simulink model "KUKA_LBR_Simulink_model_flatness_based_control"  (R2017a)
settings: Solver=VariableStepAuto  StartTime=0.0  StopTime=T  RelTol=1e-3
InitFcn:
  | main
values from neighbouring files (symbols this model uses):
  elbowAngle = elbowAngle * pi/180    (= 0)    [KUKA_LBR_init.m]    (also in Untitled2.m)
  KAnaJacNum = [k_ind 0 0 0 0 0 ;                 0  k_ind 0 0 0 0 ;                    0 0 k_ind 0 0 0 ;                      0 0 0 k_ind 0 0 ;                        0 0 0 0 k_ind 0 ;                          0 0 0 0 0 k_ind ;                            ]    [KUKA_LBR_init.m]
  Kuka_LBR_param_simu = Simulink.Parameter(Kuka_LBR_param_simu)    [KUKA_LBR_init.m]
  KUKA_LBR_x0 = [x1_0 x2_0 x3_0 x4_0 x5_0 x6_0 x7_0 x8_0 x9_0 x10_0 x11_0 x12_0 x13_0 x14_0]    [KUKA_LBR_init.m]
  rpyDes = rpyDes * pi/180    [KUKA_LBR_init.m]    (also in Untitled2.m)
  T = 0.5    [KUKA_LBR_init.m]
  vecGlobalConfig = [1; 1; 1]    [KUKA_LBR_init.m]    (also in Untitled2.m = [1, 1, 1])
undefined symbols (not defined in the file or in its folder): Kuka_LBR_param
(part 5 of 19)

== matlab function KUKA_LBR_Simulink_model_flatness_based_control/KUKA_LBR_Computed_Torque ==
  data: KUKA_LBR_param_ input; vecJointPos_ input; tau output; vecJointVel_ input; vecJointAcc_ input
function tau = KUKA_LBR_Computed_Torque(KUKA_LBR_param_,vecJointPos_,vecJointVel_,vecJointAcc_)

q1 = vecJointPos_(1);
q2 = vecJointPos_(2);
q3 = vecJointPos_(3);
q4 = vecJointPos_(4);
q5 = vecJointPos_(5);
q6 = vecJointPos_(6);
q7 = vecJointPos_(7);
q8 = vecJointVel_(1);
q9 = vecJointVel_(2);
q10 = vecJointVel_(3);
q11 = vecJointVel_(4);
q12 = vecJointVel_(5);
q13 = vecJointVel_(6);
q14 = vecJointVel_(7);


dblMassInertFullRow1Col1 = KUKA_LBR_param_.dblLink1InertZZ + (power(KUKA_LBR_param_.dblLink1CogX,2) + power(KUKA_LBR_param_.dblLink1CogY,2))*KUKA_LBR_param_.dblLink1Mass + KUKA_LBR_param_.dblLink2InertZZ + KUKA_LBR_param_.dblLink3InertZZ + KUKA_LBR_param_.dblLink4InertZZ + KUKA_LBR_param_.dblLink5InertZZ + KUKA_LBR_param_.dblLink6InertZZ + KUKA_LBR_param_.dblLink7InertZZ + KUKA_LBR_param_.dblLink2Mass*power(KUKA_LBR_param_.dblLink2CogZ*sin(q1) + cos(q1)*(KUKA_LBR_param_.dblLink2CogX*cos(q2) - KUKA_LBR_param_.dblLink2CogY*sin(q2)),2) + KUKA_LBR_param_.dblLink2Mass*power(KUKA_LBR_param_.dblLink2CogZ*cos(q1) + sin(q1)*(-(KUKA_LBR_param_.dblLink2CogX*cos(q2)) + KUKA_LBR_param_.dblLink2CogY*sin(q2)),2) + KUKA_LBR_param_.dblLink3Mass*power(cos(q1)*(KUKA_LBR_param_.dblLink3CogY*cos(q3) + KUKA_LBR_param_.dblLink3CogX*sin(q3)) + sin(q1)*(-((KUKA_LBR_param_.dblLink23Len + KUKA_LBR_param_.dblLink3CogZ)*sin(q2)) + cos(q2)*(KUKA_LBR_param_.dblLink3CogX*cos(q3) - KUKA_LBR_param_.dblLink3CogY*sin(q3))),2) + KUKA_LBR_param_.dblLink3Mass*power(sin(q1)*(KUKA_LBR_param_.dblLink3CogY*cos(q3) + KUKA_LBR_param_.dblLink3CogX*sin(q3)) + cos(q1)*((KUKA_LBR_param_.dblLink23Len + KUKA_LBR_param_.dblLink3CogZ)*sin(q2) + cos(q2)*(-(KUKA_LBR_param_.dblLink3CogX*cos(q3)) + KUKA_LBR_param_.dblLink3CogY*sin(q3))),2) + KUKA_LBR_param_.dblLink4Mass*power(cos(q1)*(KUKA_LBR_param_.dblLink4CogZ*cos(q3) + sin(q3)*(KUKA_LBR_param_.dblLink4CogX*cos(q4) - KUKA_LBR_param_.dblLink4CogY*sin(q4))) + sin(q1)*(sin(q2)*(-KUKA_LBR_param_.dblLink23Len + KUKA_LBR_param_.dblLink4CogY*cos(q4) + KUKA_LBR_param_.dblLink4CogX*sin(q4)) + cos(q2)*(KUKA_LBR_param_.dblLink4CogX*cos(q3)*cos(q4) - KUKA_LBR_param_.dblLink4CogZ*sin(q3) - KUKA_LBR_param_.dblLink4CogY*cos(q3)*sin(q4))),2) + KUKA_LBR_param_.dblLink4Mass*power(sin(q1)*(KUKA_LBR_param_.dblLink4CogZ*cos(q3) + sin(q3)*(KUKA_LBR_param_.dblLink4CogX*cos(q4) - KUKA_LBR_param_.dblLink4CogY*sin(q4))) + cos(q1)*(sin(q2)*(KUKA_LBR_param_.dblLink23Len - KUKA_LBR_param_.dblLink4CogY*cos(q4) - KUKA_LBR_param_.dblLink4CogX*sin(q4)) + cos(q2)*(-(KUKA_LBR_param_.dblLink4CogX*cos(q3)*cos(q4)) + KUKA_LBR_param_.dblLink4CogZ*sin(q3) + KUKA_LBR_param_.dblLink4CogY*cos(q3)*sin(q4))),2) + KUKA_LBR_param_.dblLink5Mass*power(sin(q1)*(cos(q3)*(KUKA_LBR_param_.dblLink5CogY*cos(q5) + KUKA_LBR_param_.dblLink5CogX*sin(q5)) + sin(q3)*((KUKA_LBR_param_.dblLink45Len + KUKA_LBR_param_.dblLink5CogZ)*sin(q4) + cos(q4)*(KUKA_LBR_param_.dblLink5CogX*cos(q5) - KUKA_LBR_param_.dblLink5CogY*sin(q5)))) + cos(q1)*(sin(q2)*(KUKA_LBR_param_.dblLink23Len + (KUKA_LBR_param_.dblLink45Len + KUKA_LBR_param_.dblLink5CogZ)*cos(q4) - KUKA_LBR_param_.dblLink5CogX*cos(q5)*sin(q4) + KUKA_LBR_param_.dblLink5CogY*sin(q4)*sin(q5)) + cos(q2)*(sin(q3)*(KUKA_LBR_param_.dblLink5CogY*cos(q5) + KUKA_LBR_param_.dblLink5CogX*sin(q5)) - cos(q3)*((KUKA_LBR_param_.dblLink45Len + KUKA_LBR_param_.dblLink5CogZ)*sin(q4) + cos(q4)*(KUKA_LBR_param_.dblLink5CogX*cos(q5) - KUKA_LBR_param_.dblLink5CogY*sin(q5))))),2) + KUKA_LBR_param_.dblLink5Mass*power(cos(q1)*(cos(q3)*(KUKA_LBR_param_.dblLink5CogY*cos(q5) + KUKA_LBR_param_.dblLink5CogX*sin(q5)) + sin(q3)*((KUKA_LBR_param_.dblLink45Len + KUKA_LBR_param_.dblLink5CogZ)*sin(q4) + cos(q4)*(KUKA_LBR_param_.dblLink5CogX*cos(q5) - KUKA_LBR_param_.dblLink5CogY*sin(q5)))) + sin(q1)*(-(sin(q2)*(KUKA_LBR_param_.dblLink23Len + (KUKA_LBR_param_.dblLink45Len + KUKA_LBR_param_.dblLink5CogZ)*cos(q4) - KUKA_LBR_param_.dblLink5CogX*cos(q5)*sin(q4) + KUKA_LBR_param_.dblLink5CogY*sin(q4)*sin(q5))) + cos(q2)*(-(sin(q3)*(KUKA_LBR_param_.dblLink5CogY*cos(q5) + KUKA_LBR_param_.dblLink5CogX*sin(q5))) + cos(q3)*((KUKA_LBR_param_.dblLink45Len + KUKA_LBR_param_.dblLink5CogZ)*sin(q4) + cos(q4)*(KUKA_LBR_param_.dblLink5CogX*cos(q5) - KUKA_LBR_param_.dblLink5CogY*sin(q5))))),2) + KUKA_LBR_param_.dblLink6Mass*power(sin(q1)*(-(cos(q3)*(KUKA_LBR_param_.dblLink6CogZ*cos(q5) + sin(q5)*(-(KUKA_LBR_param_.dblLink6CogX*cos(q6)) + KUKA_LBR_param_.dblLink6CogY*sin(q6)))) + sin(q3)*(sin(q4)*(KUKA_LBR_param_.dblLink45Len + KUKA_LBR_param_.dblLink6CogY*cos(q6) + KUKA_LBR_param_.dblLink6CogX*sin(q6)) + cos(q4)*(KUKA_LBR_param_.dblLink6CogX*cos(q5)*cos(q6) + KUKA_LBR_param_.dblLink6CogZ*sin(q5) - KUKA_LBR_param_.dblLink6CogY*cos(q5)*sin(q6)))) - cos(q1)*(-(sin(q2)*(KUKA_LBR_param_.dblLink23Len - KUKA_LBR_param_.dblLink6CogX*cos(q5)*cos(q6)*sin(q4) - KUKA_LBR_param_.dblLink6CogZ*sin(q4)*sin(q5) + KUKA_LBR_param_.dblLink6CogY*cos(q5)*sin(q4)*sin(q6) + cos(q4)*(KUKA_LBR_param_.dblLink45Len + KUKA_LBR_param_.dblLink6CogY*cos(q6) + KUKA_LBR_param_.dblLink6CogX*sin(q6)))) + cos(q2)*(sin(q3)*(KUKA_LBR_param_.dblLink6CogZ*cos(q5) + sin(q5)*(-(KUKA_LBR_param_.dblLink6CogX*cos(q6)) + KUKA_LBR_param_.dblLink6CogY*sin(q6))) + cos(q3)*(sin(q4)*(KUKA_LBR_param_.dblLink45Len + KUKA_LBR_param_.dblLink6CogY*cos(q6) + KUKA_LBR_param_.dblLink6CogX*sin(q6)) + cos(q4)*(KUKA_LBR_param_.dblLink6CogX*cos(q5)*cos(q6) + KUKA_LBR_param_.dblLink6CogZ*sin(q5) - KUKA_LBR_param_.dblLink6CogY*cos(q5)*sin(q6))))),2) + KUKA_LBR_param_.dblLink6Mass*power(cos(q1)*(-(cos(q3)*(KUKA_LBR_param_.dblLink6CogZ*cos(q5) + sin(q5)*(-(KUKA_LBR_param_.dblLink6CogX*cos(q6)) + KUKA_LBR_param_.dblLink6CogY*sin(q6)))) + sin(q3)*(sin(q4)*(KUKA_LBR_param_.dblLink45Len + KUKA_LBR_param_.dblLink6CogY*cos(q6) + KUKA_LBR_param_.dblLink6CogX*sin(q6)) + cos(q4)*(KUKA_LBR_param_.dblLink6CogX*cos(q5)*cos(q6) + KUKA_LBR_param_.dblLink6CogZ*sin(q5) - KUKA_LBR_param_.dblLink6CogY*cos(q5)*sin(q6)))) + sin(q1)*(-(sin(q2)*(KUKA_LBR_param_.dblLink23Len - KUKA_LBR_param_.dblLink6CogX*cos(q5)*cos(q6)*sin(q4) - KUKA_LBR_param_.dblLink6CogZ*sin(q4)*sin(q5) + KUKA_LBR_param_.dblLink6CogY*cos(q5)*sin(q4)*sin(q6) + cos(q4)*(KUKA_LBR_param_.dblLink45Len + KUKA_LBR_param_.dblLink6CogY*cos(q6) + KUKA_LBR_param_.dblLink6CogX*sin(q6)))) + cos(q2)*(sin(q3)*(KUKA_LBR_param_.dblLink6CogZ*cos(q5) + sin(q5)*(-(KUKA_LBR_param_.dblLink6CogX*cos(q6)) + KUKA_LBR_param_.dblLink6CogY*sin(q6))) + cos(q3)*(sin(q4)*(KUKA_LBR_param_.dblLink45Len + KUKA_LBR_param_.dblLink6CogY*cos(q6) + KUKA_LBR_param_.dblLink6CogX*sin(q6)) + cos(q4)*(KUKA_LBR_param_.dblLink6CogX*cos(q5)*cos(q6) + KUKA_LBR_param_.dblLink6CogZ*sin(q5) - KUKA_LBR_param_.dblLink6CogY*cos(q5)*sin(q6))))),2) + KUKA_LBR_param_.dblLink7Mass*power(cos(q1)*(cos(q3)*(cos(q5)*(KUKA_LBR_param_.dblLink7CogY*cos(q7) + KUKA_LBR_param_.dblLink7CogX*sin(q7)) + sin(q5)*(KUKA_LBR_param_.dblLink7CogX*cos(q6)*cos(q7) - KUKA_LBR_param_.dblLink7CogZ*sin(q6) - KUKA_LBR_param_.dblLink7CogY*cos(q6)*sin(q7))) + sin(q3)*(sin(q4)*(KUKA_LBR_param_.dblLink45Len + KUKA_LBR_param_.dblLink7CogZ*cos(q6) + KUKA_LBR_param_.dblLink7CogX*cos(q7)*sin(q6) - KUKA_LBR_param_.dblLink7CogY*sin(q6)*sin(q7)) - cos(q4)*(sin(q5)*(KUKA_LBR_param_.dblLink7CogY*cos(q7) + KUKA_LBR_param_.dblLink7CogX*sin(q7)) + cos(q5)*(-(KUKA_LBR_param_.dblLink7CogX*cos(q6)*cos(q7)) + KUKA_LBR_param_.dblLink7CogZ*sin(q6) + KUKA_LBR_param_.dblLink7CogY*cos(q6)*sin(q7))))) + sin(q1)*(-(sin(q2)*(KUKA_LBR_param_.dblLink23Len + KUKA_LBR_param_.dblLink7CogY*cos(q7)*sin(q4)*sin(q5) + KUKA_LBR_param_.dblLink7CogX*sin(q4)*sin(q5)*sin(q7) + cos(q5)*sin(q4)*(-(KUKA_LBR_param_.dblLink7CogX*cos(q6)*cos(q7)) + KUKA_LBR_param_.dblLink7CogZ*sin(q6) + KUKA_LBR_param_.dblLink7CogY*cos(q6)*sin(q7)) + cos(q4)*(KUKA_LBR_param_.dblLink45Len + KUKA_LBR_param_.dblLink7CogZ*cos(q6) + KUKA_LBR_param_.dblLink7CogX*cos(q7)*sin(q6) - KUKA_LBR_param_.dblLink7CogY*sin(q6)*sin(q7)))) + cos(q2)*(-(sin(q3)*(cos(q5)*(KUKA_LBR_param_.dblLink7CogY*cos(q7) + KUKA_LBR_param_.dblLink7CogX*sin(q7)) + sin(q5)*(KUKA_LBR_param_.dblLink7CogX*cos(q6)*cos(q7) - KUKA_LBR_param_.dblLink7CogZ*sin(q6) - KUKA_LBR_param_.dblLink7CogY*cos(q6)*sin(q7)))) + cos(q3)*(sin(q4)*(KUKA_LBR_param_.dblLink45Len + KUKA_LBR_param_.dblLink7CogZ*cos(q6) + KUKA_LBR_param_.dblLink7CogX*cos(q7)*sin(q6) - KUKA_LBR_param_.dblLink7CogY*sin(q6)*sin(q7)) - cos(q4)*(sin(q5)*(KUKA_LBR_param_.dblLink7CogY*cos(q7) + KUKA_LBR_param_.dblLink7CogX*sin(q7)) + cos(q5)*(-(KUKA_LBR_param_.dblLink7CogX*cos(q6)*cos(q7)) + KUKA_LBR_param_.dblLink7CogZ*sin(q6) + KUKA_LBR_param_.dblLink7CogY*cos(q6)*sin(q7)))))),2) + KUKA_LBR_param_.dblLink7Mass*power(sin(q1)*(cos(q3)*(cos(q5)*(KUKA_LBR_param_.dblLink7CogY*cos(q7) + KUKA_LBR_param_.dblLink7CogX*sin(q7)) + sin(q5)*(KUKA_LBR_param_.dblLink7CogX*cos(q6)*cos(q7) - KUKA_LBR_param_.dblLink7CogZ*sin(q6) - KUKA_LBR_param_.dblLink7CogY*cos(q6)*sin(q7))) + sin(q3)*(sin(q4)*(KUKA_LBR_param_.dblLink45Len + KUKA_LBR_param_.dblLink7CogZ*cos(q6) + KUKA_LBR_param_.dblLink7CogX*cos(q7)*sin(q6) - KUKA_LBR_param_.dblLink7CogY*sin(q6)*sin(q7)) - cos(q4)*(sin(q5)*(KUKA_LBR_param_.dblLink7CogY*cos(q7) + KUKA_LBR_param_.dblLink7CogX*sin(q7)) + cos(q5)*(-(KUKA_LBR_param_.dblLink7CogX*cos(q6)*cos(q7)) + KUKA_LBR_param_.dblLink7CogZ*sin(q6) + KUKA_LBR_param_.dblLink7CogY*cos(q6)*sin(q7))))) + cos(q1)*(sin(q2)*(KUKA_LBR_param_.dblLink23Len + KUKA_LBR_param_.dblLink7CogY*cos(q7)*sin(q4)*sin(q5) + KUKA_LBR_param_.dblLink7CogX*sin(q4)*sin(q5)*sin(q7) + cos(q5)*sin(q4)*(-(KUKA_LBR_param_.dblLink7CogX*cos(q6)*cos(q7)) + KUKA_LBR_param_.dblLink7CogZ*sin(q6) + KUKA_LBR_param_.dblLink7CogY*cos(q6)*sin(q7)) + cos(q4)*(KUKA_LBR_param_.dblLink45Len + KUKA_LBR_param_.dblLink7CogZ*cos(q6) + KUKA_LBR_param_.dblLink7CogX*cos(q7)*sin(q6) - KUKA_LBR_param_.dblLink7CogY*sin(q6)*sin(q7))) + cos(q2)*(sin(q3)*(cos(q5)*(KUKA_LBR_param_.dblLink7CogY*cos(q7) + KUKA_LBR_param_.dblLink7CogX*sin(q7)) + sin(q5)*(KUKA_LBR_param_.dblLink7CogX*cos(q6)*cos(q7) - KUKA_LBR_param_.dblLink7CogZ*sin(q6) - KUKA_LBR_param_.dblLink7CogY*cos(q6)*sin(q7))) + cos(q3)*(-(sin(q4)*(KUKA_LBR_param_.dblLink45Len + KUKA_LBR_param_.dblLink7CogZ*cos(q6) + KUKA_LBR_param_.dblLink7CogX*cos(q7)*sin(q6) - KUKA_LBR_param_.dblLink7CogY*sin(q6)*sin(q7))) + cos(q4)*(sin(q5)*(KUKA_LBR_param_.dblLink7CogY*cos(q7) + KUKA_LBR_param_.dblLink7CogX*sin(q7)) + cos(q5)*(-(KUKA_LBR_param_.dblLink7CogX*cos(q6)*cos(q7)) + KUKA_LBR_param_.dblLink7CogZ*sin(q6) + KUKA_LBR_param_.dblLink7CogY*cos(q6)*sin(q7)))))),2);
dblMassInertFullRow1Col2 = KUKA_LBR_param_.dblLink2InertYZ*cos(q1) + KUKA_LBR_param_.dblLink3InertYZ*cos(q1) + KUKA_LBR_param_.dblLink4InertYZ*cos(q1) + KUKA_LBR_param_.dblLink5InertYZ*cos(q1) + KUKA_LBR_param_.dblLink6InertYZ*cos(q1) + KUKA_LBR_param_.dblLink7InertYZ*cos(q1) - KUKA_LBR_param_.dblLink2CogY*KUKA_LBR_param_.dblLink2CogZ*KUKA_LBR_param_.dblLink2Mass*cos(q2) - KUKA_LBR_param_.dblLink2InertXZ*sin(q1) - KUKA_LBR_param_.dblLink3InertXZ*sin(q1) - KUKA_LBR_param_.dblLink4InertXZ*sin(q1) - KUKA_LBR_param_.dblLink5InertXZ*sin(q1) - KUKA_LBR_param_.dblLink6InertXZ*sin(q1) - KUKA_LBR_param_.dblLink7InertXZ*sin(q1) - KUKA_LBR_param_.dblLink2CogX*KUKA_LBR_param_.dblLink2CogZ*KUKA_LBR_param_.dblLink2Mass*sin(q2) + KUKA_LBR_param_.dblLink3CogX*KUKA_LBR_param_.dblLink3CogY*KUKA_LBR_param_.dblLink3Mass*power(cos(q3),2)*sin(q2) + power(KUKA_LBR_param_.dblLink3CogX,2)*KUKA_LBR_param_.dblLink3Mass*cos(q3)*sin(q2)*sin(q3) - power(KUKA_LBR_param_.dblLink3CogY,2)*KUKA_LBR_param_.dblLink3Mass*cos(q3)*sin(q2)*sin(q3) - KUKA_LBR_param_.dblLink3CogX*KUKA_LBR_param_.dblLink3CogY*KUKA_LBR_param_.dblLink3Mass*sin(q2)*power(sin(q3),2) + (KUKA_LBR_param_.dblLink23Len + KUKA_LBR_param_.dblLink3CogZ)*KUKA_LBR_param_.dblLink3Mass*cos(q2)*(KUKA_LBR_param_.dblLink3CogY*cos(q3) + KUKA_LBR_param_.dblLink3CogX*sin(q3)) + KUKA_LBR_param_.dblLink4Mass*cos(q1)*(cos(q2)*(KUKA_LBR_param_.dblLink23Len - KUKA_LBR_param_.dblLink4CogY*cos(q4) - KUKA_LBR_param_.dblLink4CogX*sin(q4)) - sin(q2)*(KUKA_LBR_param_.dblLink4CogZ*sin(q3) + cos(q3)*(-(KUKA_LBR_param_.dblLink4CogX*cos(q4)) + KUKA_LBR_param_.dblLink4CogY*sin(q4))))*(cos(q1)*(KUKA_LBR_param_.dblLink4CogZ*cos(q3) + sin(q3)*(KUKA_LBR_param_.dblLink4CogX*cos(q4) - KUKA_LBR_param_.dblLink4CogY*sin(q4))) + sin(q1)*(sin(q2)*(-KUKA_LBR_param_.dblLink23Len + KUKA_LBR_param_.dblLink4CogY*cos(q4) + KUKA_LBR_param_.dblLink4CogX*sin(q4)) + cos(q2)*(KUKA_LBR_param_.dblLink4CogX*cos(q3)*cos(q4) - KUKA_LBR_param_.dblLink4CogZ*sin(q3) - KUKA_LBR_param_.dblLink4CogY*cos(q3)*sin(q4)))) + KUKA_LBR_param_.dblLink4Mass*sin(q1)*(cos(q2)*(KUKA_LBR_param_.dblLink23Len - KUKA_LBR_param_.dblLink4CogY*cos(q4) - KUKA_LBR_param_.dblLink4CogX*sin(q4)) - sin(q2)*(KUKA_LBR_param_.dblLink4CogZ*sin(q3) + cos(q3)*(-(KUKA_LBR_param_.dblLink4CogX*cos(q4)) + KUKA_LBR_param_.dblLink4CogY*sin(q4))))*(sin(q1)*(KUKA_LBR_param_.dblLink4CogZ*cos(q3) + sin(q3)*(KUKA_LBR_param_.dblLink4CogX*cos(q4) - KUKA_LBR_param_.dblLink4CogY*sin(q4))) + cos(q1)*(sin(q2)*(KUKA_LBR_param_.dblLink23Len - KUKA_LBR_param_.dblLink4CogY*cos(q4) - KUKA_LBR_param_.dblLink4CogX*sin(q4)) + cos(q2)*(-(KUKA_LBR_param_.dblLink4CogX*cos(q3)*cos(q4)) + KUKA_LBR_param_.dblLink4CogZ*sin(q3) + KUKA_LBR_param_.dblLink4CogY*cos(q3)*sin(q4)))) + KUKA_LBR_param_.dblLink5Mass*sin(q1)*(cos(q2)*(KUKA_LBR_param_.dblLink23Len + (KUKA_LBR_param_.dblLink45Len + KUKA_LBR_param_.dblLink5CogZ)*cos(q4) - KUKA_LBR_param_.dblLink5CogX*cos(q5)*sin(q4) + KUKA_LBR_param_.dblLink5CogY*sin(q4)*sin(q5)) + sin(q2)*(-(sin(q3)*(KUKA_LBR_param_.dblLink5CogY*cos(q5) + KUKA_LBR_param_.dblLink5CogX*sin(q5))) + cos(q3)*((KUKA_LBR_param_.dblLink45Len + KUKA_LBR_param_.dblLink5CogZ)*sin(q4) + cos(q4)*(KUKA_LBR_param_.dblLink5CogX*cos(q5) - KUKA_LBR_param_.dblLink5CogY*sin(q5)))))*(sin(q1)*(cos(q3)*(KUKA_LBR_param_.dblLink5CogY*cos(q5) + KUKA_LBR_param_.dblLink5CogX*sin(q5)) + sin(q3)*((KUKA_LBR_param_.dblLink45Len + KUKA_LBR_param_.dblLink5CogZ)*sin(q4) + cos(q4)*(KUKA_LBR_param_.dblLink5CogX*cos(q5) - KUKA_LBR_param_.dblLink5CogY*sin(q5)))) + cos(q1)*(sin(q2)*(KUKA_LBR_param_.dblLink23Len + (KUKA_LBR_param_.dblLink45Len + KUKA_LBR_param_.dblLink5CogZ)*cos(q4) - KUKA_LBR_param_.dblLink5CogX*cos(q5)*sin(q4) + KUKA_LBR_param_.dblLink5CogY*sin(q4)*sin(q5)) + cos(q2)*(sin(q3)*(KUKA_LBR_param_.dblLink5CogY*cos(q5) + KUKA_LBR_param_.dblLink5CogX*sin(q5)) - cos(q3)*((KUKA_LBR_param_.dblLink45Len + KUKA_LBR_param_.dblLink5CogZ)*sin(q4) + cos(q4)*(KUKA_LBR_param_.dblLink5CogX*cos(q5) - KUKA_LBR_param_.dblLink5CogY*sin(q5)))))) + KUKA_LBR_param_.dblLink5Mass*cos(q1)*(cos(q2)*(KUKA_LBR_param_.dblLink23Len + (KUKA_LBR_param_.dblLink45Len + KUKA_LBR_param_.dblLink5CogZ)*cos(q4) - KUKA_LBR_param_.dblLink5CogX*cos(q5)*sin(q4) + KUKA_LBR_param_.dblLink5CogY*sin(q4)*sin(q5)) + sin(q2)*(-(sin(q3)*(KUKA_LBR_param_.dblLink5CogY*cos(q5) + KUKA_LBR_param_.dblLink5CogX*sin(q5))) + cos(q3)*((KUKA_LBR_param_.dblLink45Len + KUKA_LBR_param_.dblLink5CogZ)*sin(q4) + cos(q4)*(KUKA_LBR_param_.dblLink5CogX*cos(q5) - KUKA_LBR_param_.dblLink5CogY*sin(q5)))))*(cos(q1)*(cos(q3)*(KUKA_LBR_param_.dblLink5CogY*cos(q5) + KUKA_LBR_param_.dblLink5CogX*sin(q5)) + sin(q3)*((KUKA_LBR_param_.dblLink45Len + KUKA_LBR_param_.dblLink5CogZ)*sin(q4) + cos(q4)*(KUKA_LBR_param_.dblLink5CogX*cos(q5) - KUKA_LBR_param_.dblLink5CogY*sin(q5)))) + sin(q1)*(-(sin(q2)*(KUKA_LBR_param_.dblLink23Len + (KUKA_LBR_param_.dblLink45Len + KUKA_LBR_param_.dblLink5CogZ)*cos(q4) - KUKA_LBR_param_.dblLink5CogX*cos(q5)*sin(q4) + KUKA_LBR_param_.dblLink5CogY*sin(q4)*sin(q5))) + cos(q2)*(-(sin(q3)*(KUKA_LBR_param_.dblLink5CogY*cos(q5) + KUKA_LBR_param_.dblLink5CogX*sin(q5))) + cos(q3)*((KUKA_LBR_param_.dblLink45Len + KUKA_LBR_param_.dblLink5CogZ)*sin(q4) + cos(q4)*(KUKA_LBR_param_.dblLink5CogX*cos(q5) - KUKA_LBR_param_.dblLink5CogY*sin(q5)))))) + KUKA_LBR_param_.dblLink6Mass*sin(q1)*(cos(q2)*(KUKA_LBR_param_.dblLink23Len - KUKA_LBR_param_.dblLink6CogX*cos(q5)*cos(q6)*sin(q4) - KUKA_LBR_param_.dblLink6CogZ*sin(q4)*sin(q5) + KUKA_LBR_param_.dblLink6CogY*cos(q5)*sin(q4)*sin(q6) + cos(q4)*(KUKA_LBR_param_.dblLink45Len + KUKA_LBR_param_.dblLink6CogY*cos(q6) + KUKA_LBR_param_.dblLink6CogX*sin(q6))) + sin(q2)*(sin(q3)*(KUKA_LBR_param_.dblLink6CogZ*cos(q5) + sin(q5)*(-(KUKA_LBR_param_.dblLink6CogX*cos(q6)) + KUKA_LBR_param_.dblLink6CogY*sin(q6))) + cos(q3)*(sin(q4)*(KUKA_LBR_param_.dblLink45Len + KUKA_LBR_param_.dblLink6CogY*cos(q6) + KUKA_LBR_param_.dblLink6CogX*sin(q6)) + cos(q4)*(KUKA_LBR_param_.dblLink6CogX*cos(q5)*cos(q6) + KUKA_LBR_param_.dblLink6CogZ*sin(q5) - KUKA_LBR_param_.dblLink6CogY*cos(q5)*sin(q6)))))*(sin(q1)*(-(cos(q3)*(KUKA_LBR_param_.dblLink6CogZ*cos(q5) + sin(q5)*(-(KUKA_LBR_param_.dblLink6CogX*cos(q6)) + KUKA_LBR_param_.dblLink6CogY*sin(q6)))) + sin(q3)*(sin(q4)*(KUKA_LBR_param_.dblLink45Len + KUKA_LBR_param_.dblLink6CogY*cos(q6) + KUKA_LBR_param_.dblLink6CogX*sin(q6)) + cos(q4)*(KUKA_LBR_param_.dblLink6CogX*cos(q5)*cos(q6) + KUKA_LBR_param_.dblLink6CogZ*sin(q5) - KUKA_LBR_param_.dblLink6CogY*cos(q5)*sin(q6)))) - cos(q1)*(-(sin(q2)*(KUKA_LBR_param_.dblLink23Len - KUKA_LBR_param_.dblLink6CogX*cos(q5)*cos(q6)*sin(q4) - KUKA_LBR_param_.dblLink6CogZ*sin(q4)*sin(q5) + KUKA_LBR_param_.dblLink6CogY*cos(q5)*sin(q4)*sin(q6) + cos(q4)*(KUKA_LBR_param_.dblLink45Len + KUKA_LBR_param_.dblLink6CogY*cos(q6) + KUKA_LBR_param_.dblLink6CogX*sin(q6)))) + cos(q2)*(sin(q3)*(KUKA_LBR_param_.dblLink6CogZ*cos(q5) + sin(q5)*(-(KUKA_LBR_param_.dblLink6CogX*cos(q6)) + KUKA_LBR_param_.dblLink6CogY*sin(q6))) + cos(q3)*(sin(q4)*(KUKA_LBR_param_.dblLink45Len + KUKA_LBR_param_.dblLink6CogY*cos(q6) + KUKA_LBR_param_.dblLink6CogX*sin(q6)) + cos(q4)*(KUKA_LBR_param_.dblLink6CogX*cos(q5)*cos(q6) + KUKA_LBR_param_.dblLink6CogZ*sin(q5) - KUKA_LBR_param_.dblLink6CogY*cos(q5)*sin(q6)))))) + KUKA_LBR_param_.dblLink6Mass*cos(q1)*(cos(q2)*(KUKA_LBR_param_.dblLink23Len - KUKA_LBR_param_.dblLink6CogX*cos(q5)*cos(q6)*sin(q4) - KUKA_LBR_param_.dblLink6CogZ*sin(q4)*sin(q5) + KUKA_LBR_param_.dblLink6CogY*cos(q5)*sin(q4)*sin(q6) + cos(q4)*(KUKA_LBR_param_.dblLink45Len + KUKA_LBR_param_.dblLink6CogY*cos(q6) + KUKA_LBR_param_.dblLink6CogX*sin(q6))) + sin(q2)*(sin(q3)*(KUKA_LBR_param_.dblLink6CogZ*cos(q5) + sin(q5)*(-(KUKA_LBR_param_.dblLink6CogX*cos(q6)) + KUKA_LBR_param_.dblLink6CogY*sin(q6))) + cos(q3)*(sin(q4)*(KUKA_LBR_param_.dblLink45Len + KUKA_LBR_param_.dblLink6CogY*cos(q6) + KUKA_LBR_param_.dblLink6CogX*sin(q6)) + cos(q4)*(KUKA_LBR_param_.dblLink6CogX*cos(q5)*cos(q6) + KUKA_LBR_param_.dblLink6CogZ*sin(q5) - KUKA_LBR_param_.dblLink6CogY*cos(q5)*sin(q6)))))*(cos(q1)*(-(cos(q3)*(KUKA_LBR_param_.dblLink6CogZ*cos(q5) + sin(q5)*(-(KUKA_LBR_param_.dblLink6CogX*cos(q6)) + KUKA_LBR_param_.dblLink6CogY*sin(q6)))) + sin(q3)*(sin(q4)*(KUKA_LBR_param_.dblLink45Len + KUKA_LBR_param_.dblLink6CogY*cos(q6) + KUKA_LBR_param_.dblLink6CogX*sin(q6)) + cos(q4)*(KUKA_LBR_param_.dblLink6CogX*cos(q5)*cos(q6) + KUKA_LBR_param_.dblLink6CogZ*sin(q5) - KUKA_LBR_param_.dblLink6CogY*cos(q5)*sin(q6)))) + sin(q1)*(-(sin(q2)*(KUKA_LBR_param_.dblLink23Len - KUKA_LBR_param_.dblLink6CogX*cos(q5)*cos(q6)*sin(q4) - KUKA_LBR_param_.dblLink6CogZ*sin(q4)*sin(q5) + KUKA_LBR_param_.dblLink6CogY*cos(q5)*sin(q4)*sin(q6) + cos(q4)*(KUKA_LBR_param_.dblLink45Len + KUKA_LBR_param_.dblLink6CogY*cos(q6) + KUKA_LBR_param_.dblLink6CogX*sin(q6)))) + cos(q2)*(sin(q3)*(KUKA_LBR_param_.dblLink6CogZ*cos(q5) + sin(q5)*(-(KUKA_LBR_param_.dblLink6CogX*cos(q6)) + KUKA_LBR_param_.dblLink6CogY*sin(q6))) + cos(q3)*(sin(q4)*(KUKA_LBR_param_.dblLink45Len + KUKA_LBR_param_.dblLink6CogY*cos(q6) + KUKA_LBR_param_.dblLink6CogX*sin(q6)) + cos(q4)*(KUKA_LBR_param_.dblLink6CogX*cos(q5)*cos(q6) + KUKA_LBR_param_.dblLink6CogZ*sin(q5) - KUKA_LBR_param_.dblLink6CogY*cos(q5)*sin(q6)))))) + KUKA_LBR_param_.dblLink7Mass*sin(q1)*(cos(q2)*(KUKA_LBR_param_.dblLink23Len + KUKA_LBR_param_.dblLink7CogY*cos(q7)*sin(q4)*sin(q5) + KUKA_LBR_param_.dblLink7CogX*sin(q4)*sin(q5)*sin(q7) + cos(q5)*sin(q4)*(-(KUKA_LBR_param_.dblLink7CogX*cos(q6)*cos(q7)) + KUKA_LBR_param_.dblLink7CogZ*sin(q6) + KUKA_LBR_param_.dblLink7CogY*cos(q6)*sin(q7)) + cos(q4)*(KUKA_LBR_param_.dblLink45Len + KUKA_LBR_param_.dblLink7CogZ*cos(q6) + KUKA_LBR_param_.dblLink7CogX*cos(q7)*sin(q6) - KUKA_LBR_param_.dblLink7CogY*sin(q6)*sin(q7))) + sin(q2)*(-(sin(q3)*(cos(q5)*(KUKA_LBR_param_.dblLink7CogY*cos(q7) + KUKA_LBR_param_.dblLink7CogX*sin(q7)) + sin(q5)*(KUKA_LBR_param_.dblLink7CogX*cos(q6)*cos(q7) - KUKA_LBR_param_.dblLink7CogZ*sin(q6) - KUKA_LBR_param_.dblLink7CogY*cos(q6)*sin(q7)))) + cos(q3)*(sin(q4)*(KUKA_LBR_param_.dblLink45Len + KUKA_LBR_param_.dblLink7CogZ*cos(q6) + KUKA_LBR_param_.dblLink7CogX*cos(q7)*sin(q6) - KUKA_LBR_param_.dblLink7CogY*sin(q6)*sin(q7)) - cos(q4)*(sin(q5)*(KUKA_LBR_param_.dblLink7CogY*cos(q7) + KUKA_LBR_param_.dblLink7CogX*sin(q7)) + cos(q5)*(-(KUKA_LBR_param_.dblLink7CogX*cos(q6)*cos(q7)) + KUKA_LBR_param_.dblLink7CogZ*sin(q6) + KUKA_LBR_param_.dblLink7CogY*cos(q6)*sin(q7))))))*(sin(q1)*(cos(q3)*(cos(q5)*(KUKA_LBR_param_.dblLink7CogY*cos(q7) + KUKA_LBR_param_.dblLink7CogX*sin(q7)) + sin(q5)*(KUKA_LBR_param_.dblLink7CogX*cos(q6)*cos(q7) - KUKA_LBR_param_.dblLink7CogZ*sin(q6) - KUKA_LBR_param_.dblLink7CogY*cos(q6)*sin(q7))) + sin(q3)*(sin(q4)*(KUKA_LBR_param_.dblLink45Len + KUKA_LBR_param_.dblLink7CogZ*cos(q6) + KUKA_LBR_param_.dblLink7CogX*cos(q7)*sin(q6) - KUKA_LBR_param_.dblLink7CogY*sin(q6)*sin(q7)) - cos(q4)*(sin(q5)*(KUKA_LBR_param_.dblLink7CogY*cos(q7) + KUKA_LBR_param_.dblLink7CogX*sin(q7)) + cos(q5)*(-(KUKA_LBR_param_.dblLink7CogX*cos(q6)*cos(q7)) + KUKA_LBR_param_.dblLink7CogZ*sin(q6) + KUKA_LBR_param_.dblLink7CogY*cos(q6)*sin(q7))))) + cos(q1)*(sin(q2)*(KUKA_LBR_param_.dblLink23Len + KUKA_LBR_param_.dblLink7CogY*cos(q7)*sin(q4)*sin(q5) + KUKA_LBR_param_.dblLink7CogX*sin(q4)*sin(q5)*sin(q7) + cos(q5)*sin(q4)*(-(KUKA_LBR_param_.dblLink7CogX*cos(q6)*cos(q7)) + KUKA_LBR_param_.dblLink7CogZ*sin(q6) + KUKA_LBR_param_.dblLink7CogY*cos(q6)*sin(q7)) + cos(q4)*(KUKA_LBR_param_.dblLink45Len + KUKA_LBR_param_.dblLink7CogZ*cos(q6) + KUKA_LBR_param_.dblLink7CogX*cos(q7)*sin(q6) - KUKA_LBR_param_.dblLink7CogY*sin(q6)*sin(q7))) + cos(q2)*(sin(q3)*(cos(q5)*(KUKA_LBR_param_.dblLink7CogY*cos(q7) + KUKA_LBR_param_.dblLink7CogX*sin(q7)) + sin(q5)*(KUKA_LBR_param_.dblLink7CogX*cos(q6)*cos(q7) - KUKA_LBR_param_.dblLink7CogZ*sin(q6) - KUKA_LBR_param_.dblLink7CogY*cos(q6)*sin(q7))) + cos(q3)*(-(sin(q4)*(KUKA_LBR_param_.dblLink45Len + KUKA_LBR_param_.dblLink7CogZ*cos(q6) + KUKA_LBR_param_.dblLink7CogX*cos(q7)*sin(q6) - KUKA_LBR_param_.dblLink7CogY*sin(q6)*sin(q7))) + cos(q4)*(sin(q5)*(KUKA_LBR_param_.dblLink7CogY*cos(q7) + KUKA_LBR_param_.dblLink7CogX*sin(q7)) + cos(q5)*(-(KUKA_LBR_param_.dblLink7CogX*cos(q6)*cos(q7)) + KUKA_LBR_param_.dblLink7CogZ*sin(q6) + KUKA_LBR_param_.dblLink7CogY*cos(q6)*sin(q7))))))) - KUKA_LBR_param_.dblLink7Mass*cos(q1)*(cos(q2)*(KUKA_LBR_param_.dblLink23Len + KUKA_LBR_param_.dblLink7CogY*cos(q7)*sin(q4)*sin(q5) + KUKA_LBR_param_.dblLink7CogX*sin(q4)*sin(q5)*sin(q7) + cos(q5)*sin(q4)*(-(KUKA_LBR_param_.dblLink7CogX*cos(q6)*cos(q7)) + KUKA_LBR_param_.dblLink7CogZ*sin(q6) + KUKA_LBR_param_.dblLink7CogY*cos(q6)*sin(q7)) + cos(q4)*(KUKA_LBR_param_.dblLink45Len + KUKA_LBR_param_.dblLink7CogZ*cos(q6) + KUKA_LBR_param_.dblLink7CogX*cos(q7)*sin(q6) - KUKA_LBR_param_.dblLink7CogY*sin(q6)*sin(q7))) + sin(q2)*(-(sin(q3)*(cos(q5)*(KUKA_LBR_param_.dblLink7CogY*cos(q7) + KUKA_LBR_param_.dblLink7CogX*sin(q7)) + sin(q5)*(KUKA_LBR_param_.dblLink7CogX*cos(q6)*cos(q7) - KUKA_LBR_param_.dblLink7CogZ*sin(q6) - KUKA_LBR_param_.dblLink7CogY*cos(q6)*sin(q7)))) + cos(q3)*(sin(q4)*(KUKA_LBR_param_.dblLink45Len + KUKA_LBR_param_.dblLink7CogZ*cos(q6) + KUKA_LBR_param_.dblLink7CogX*cos(q7)*sin(q6) - KUKA_LBR_param_.dblLink7CogY*sin(q6)*sin(q7)) - cos(q4)*(sin(q5)*(KUKA_LBR_param_.dblLink7CogY*cos(q7) + KUKA_LBR_param_.dblLink7CogX*sin(q7)) + cos(q5)*(-(KUKA_LBR_param_.dblLink7CogX*cos(q6)*cos(q7)) + KUKA_LBR_param_.dblLink7CogZ*sin(q6) + KUKA_LBR_param_.dblLink7CogY*cos(q6)*sin(q7))))))*(cos(q1)*(-(cos(q3)*(cos(q5)*(KUKA_LBR_param_.dblLink7CogY*cos(q7) + KUKA_LBR_param_.dblLink7CogX*sin(q7)) + sin(q5)*(KUKA_LBR_param_.dblLink7CogX*cos(q6)*cos(q7) - KUKA_LBR_param_.dblLink7CogZ*sin(q6) - KUKA_LBR_param_.dblLink7CogY*cos(q6)*sin(q7)))) + sin(q3)*(-(sin(q4)*(KUKA_LBR_param_.dblLink45Len + KUKA_LBR_param_.dblLink7CogZ*cos(q6) + KUKA_LBR_param_.dblLink7CogX*cos(q7)*sin(q6) - KUKA_LBR_param_.dblLink7CogY*sin(q6)*sin(q7))) + cos(q4)*(sin(q5)*(KUKA_LBR_param_.dblLink7CogY*cos(q7) + KUKA_LBR_param_.dblLink7CogX*sin(q7)) + cos(q5)*(-(KUKA_LBR_param_.dblLink7CogX*cos(q6)*cos(q7)) + KUKA_LBR_param_.dblLink7CogZ*sin(q6) + KUKA_LBR_param_.dblLink7CogY*cos(q6)*sin(q7))))) + sin(q1)*(sin(q2)*(KUKA_LBR_param_.dblLink23Len + KUKA_LBR_param_.dblLink7CogY*cos(q7)*sin(q4)*sin(q5) + KUKA_LBR_param_.dblLink7CogX*sin(q4)*sin(q5)*sin(q7) + cos(q5)*sin(q4)*(-(KUKA_LBR_param_.dblLink7CogX*cos(q6)*cos(q7)) + KUKA_LBR_param_.dblLink7CogZ*sin(q6) + KUKA_LBR_param_.dblLink7CogY*cos(q6)*sin(q7)) + cos(q4)*(KUKA_LBR_param_.dblLink45Len + KUKA_LBR_param_.dblLink7CogZ*cos(q6) + KUKA_LBR_param_.dblLink7CogX*cos(q7)*sin(q6) - KUKA_LBR_param_.dblLink7CogY*sin(q6)*sin(q7))) + cos(q2)*(sin(q3)*(cos(q5)*(KUKA_LBR_param_.dblLink7CogY*cos(q7) + KUKA_LBR_param_.dblLink7CogX*sin(q7)) + sin(q5)*(KUKA_LBR_param_.dblLink7CogX*cos(q6)*cos(q7) - KUKA_LBR_param_.dblLink7CogZ*sin(q6) - KUKA_LBR_param_.dblLink7CogY*cos(q6)*sin(q7))) + cos(q3)*(-(sin(q4)*(KUKA_LBR_param_.dblLink45Len + KUKA_LBR_param_.dblLink7CogZ*cos(q6) + KUKA_LBR_param_.dblLink7CogX*cos(q7)*sin(q6) - KUKA_LBR_param_.dblLink7CogY*sin(q6)*sin(q7))) + cos(q4)*(sin(q5)*(KUKA_LBR_param_.dblLink7CogY*cos(q7) + KUKA_LBR_param_.dblLink7CogX*sin(q7)) + cos(q5)*(-(KUKA_LBR_param_.dblLink7CogX*cos(q6)*cos(q7)) + KUKA_LBR_param_.dblLink7CogZ*sin(q6) + KUKA_LBR_param_.dblLink7CogY*cos(q6)*sin(q7)))))));
dblMassInertFullRow1Col3 = (KUKA_LBR_param_.dblLink3InertZZ + (power(KUKA_LBR_param_.dblLink3CogX,2) + power(KUKA_LBR_param_.dblLink3CogY,2))*KUKA_LBR_param_.dblLink3Mass)*cos(q2) + KUKA_LBR_param_.dblLink5InertZZ*cos(q2) + KUKA_LBR_param_.dblLink6InertZZ*cos(q2) + KUKA_LBR_param_.dblLink7InertZZ*cos(q2) + KUKA_LBR_param_.dblLink5InertXZ*cos(q1)*sin(q2) + KUKA_LBR_param_.dblLink6InertXZ*cos(q1)*sin(q2) + KUKA_LBR_param_.dblLink7InertXZ*cos(q1)*sin(q2) + KUKA_LBR_param_.dblLink5InertYZ*sin(q1)*sin(q2) + KUKA_LBR_param_.dblLink6InertYZ*sin(q1)*sin(q2) + KUKA_LBR_param_.dblLink7InertYZ*sin(q1)*sin(q2) + sin(q2)*(KUKA_LBR_param_.dblLink3InertXZ*cos(q1) - KUKA_LBR_param_.dblLink3CogX*(KUKA_LBR_param_.dblLink23Len + KUKA_LBR_param_.dblLink3CogZ)*KUKA_LBR_param_.dblLink3Mass*cos(q3) + KUKA_LBR_param_.dblLink3InertYZ*sin(q1) + KUKA_LBR_param_.dblLink23Len*KUKA_LBR_param_.dblLink3CogY*KUKA_LBR_param_.dblLink3Mass*sin(q3) + KUKA_LBR_param_.dblLink3CogY*KUKA_LBR_param_.dblLink3CogZ*KUKA_LBR_param_.dblLink3Mass*sin(q3)) + (2*sin(q2)*(KUKA_LBR_param_.dblLink4InertXZ*cos(q1) + KUKA_LBR_param_.dblLink4InertYZ*sin(q1) + KUKA_LBR_param_.dblLink23Len*KUKA_LBR_param_.dblLink4CogZ*KUKA_LBR_param_.dblLink4Mass*sin(q3) - KUKA_LBR_param_.dblLink4CogY*KUKA_LBR_param_.dblLink4CogZ*KUKA_LBR_param_.dblLink4Mass*cos(q4)*sin(q3) - KUKA_LBR_param_.dblLink4CogX*KUKA_LBR_param_.dblLink4CogZ*KUKA_LBR_param_.dblLink4Mass*sin(q3)*sin(q4) + KUKA_LBR_param_.dblLink4Mass*cos(q3)*(-KUKA_LBR_param_.dblLink23Len + KUKA_LBR_param_.dblLink4CogY*cos(q4) + KUKA_LBR_param_.dblLink4CogX*sin(q4))*(KUKA_LBR_param_.dblLink4CogX*cos(q4) - KUKA_LBR_param_.dblLink4CogY*sin(q4))) + cos(q2)*(2*KUKA_LBR_param_.dblLink4InertZZ + power(KUKA_LBR_param_.dblLink4CogX,2)*KUKA_LBR_param_.dblLink4Mass + power(KUKA_LBR_param_.dblLink4CogY,2)*KUKA_LBR_param_.dblLink4Mass + 2*power(KUKA_LBR_param_.dblLink4CogZ,2)*KUKA_LBR_param_.dblLink4Mass + (power(KUKA_LBR_param_.dblLink4CogX,2) - power(KUKA_LBR_param_.dblLink4CogY,2))*KUKA_LBR_param_.dblLink4Mass*cos(2*q4) - 2*KUKA_LBR_param_.dblLink4CogX*KUKA_LBR_param_.dblLink4CogY*KUKA_LBR_param_.dblLink4Mass*sin(2*q4)))/2.0 + KUKA_LBR_param_.dblLink5Mass*(cos(q1)*(sin(q3)*(KUKA_LBR_param_.dblLink5CogY*cos(q5) + KUKA_LBR_param_.dblLink5CogX*sin(q5)) - cos(q3)*((KUKA_LBR_param_.dblLink45Len + KUKA_LBR_param_.dblLink5CogZ)*sin(q4) + cos(q4)*(KUKA_LBR_param_.dblLink5CogX*cos(q5) - KUKA_LBR_param_.dblLink5CogY*sin(q5)))) + cos(q2)*sin(q1)*(cos(q3)*(KUKA_LBR_param_.dblLink5CogY*cos(q5) + KUKA_LBR_param_.dblLink5CogX*sin(q5)) + sin(q3)*((KUKA_LBR_param_.dblLink45Len + KUKA_LBR_param_.dblLink5CogZ)*sin(q4) + cos(q4)*(KUKA_LBR_param_.dblLink5CogX*cos(q5) - KUKA_LBR_param_.dblLink5CogY*sin(q5)))))*(sin(q1)*(cos(q3)*(KUKA_LBR_param_.dblLink5CogY*cos(q5) + KUKA_LBR_param_.dblLink5CogX*sin(q5)) + sin(q3)*((KUKA_LBR_param_.dblLink45Len + KUKA_LBR_param_.dblLink5CogZ)*sin(q4) + cos(q4)*(KUKA_LBR_param_.dblLink5CogX*cos(q5) - KUKA_LBR_param_.dblLink5CogY*sin(q5)))) + cos(q1)*(sin(q2)*(KUKA_LBR_param_.dblLink23Len + (KUKA_LBR_param_.dblLink45Len + KUKA_LBR_param_.dblLink5CogZ)*cos(q4) - KUKA_LBR_param_.dblLink5CogX*cos(q5)*sin(q4) + KUKA_LBR_param_.dblLink5CogY*sin(q4)*sin(q5)) + cos(q2)*(sin(q3)*(KUKA_LBR_param_.dblLink5CogY*cos(q5) + KUKA_LBR_param_.dblLink5CogX*sin(q5)) - cos(q3)*((KUKA_LBR_param_.dblLink45Len + KUKA_LBR_param_.dblLink5CogZ)*sin(q4) + cos(q4)*(KUKA_LBR_param_.dblLink5CogX*cos(q5) - KUKA_LBR_param_.dblLink5CogY*sin(q5)))))) + KUKA_LBR_param_.dblLink5Mass*(sin(q1)*(-(sin(q3)*(KUKA_LBR_param_.dblLink5CogY*cos(q5) + KUKA_LBR_param_.dblLink5CogX*sin(q5))) + cos(q3)*((KUKA_LBR_param_.dblLink45Len + KUKA_LBR_param_.dblLink5CogZ)*sin(q4) + cos(q4)*(KUKA_LBR_param_.dblLink5CogX*cos(q5) - KUKA_LBR_param_.dblLink5CogY*sin(q5)))) + cos(q1)*cos(q2)*(cos(q3)*(KUKA_LBR_param_.dblLink5CogY*cos(q5) + KUKA_LBR_param_.dblLink5CogX*sin(q5)) + sin(q3)*((KUKA_LBR_param_.dblLink45Len + KUKA_LBR_param_.dblLink5CogZ)*sin(q4) + cos(q4)*(KUKA_LBR_param_.dblLink5CogX*cos(q5) - KUKA_LBR_param_.dblLink5CogY*sin(q5)))))*(cos(q1)*(cos(q3)*(KUKA_LBR_param_.dblLink5CogY*cos(q5) + KUKA_LBR_param_.dblLink5CogX*sin(q5)) + sin(q3)*((KUKA_LBR_param_.dblLink45Len + KUKA_LBR_param_.dblLink5CogZ)*sin(q4) + cos(q4)*(KUKA_LBR_param_.dblLink5CogX*cos(q5) - KUKA_LBR_param_.dblLink5CogY*sin(q5)))) + sin(q1)*(-(sin(q2)*(KUKA_LBR_param_.dblLink23Len + (KUKA_LBR_param_.dblLink45Len + KUKA_LBR_param_.dblLink5CogZ)*cos(q4) - KUKA_LBR_param_.dblLink5CogX*cos(q5)*sin(q4) + KUKA_LBR_param_.dblLink5CogY*sin(q4)*sin(q5))) + cos(q2)*(-(sin(q3)*(KUKA_LBR_param_.dblLink5CogY*cos(q5) + KUKA_LBR_param_.dblLink5CogX*sin(q5))) + cos(q3)*((KUKA_LBR_param_.dblLink45Len + KUKA_LBR_param_.dblLink5CogZ)*sin(q4) + cos(q4)*(KUKA_LBR_param_.dblLink5CogX*cos(q5) - KUKA_LBR_param_.dblLink5CogY*sin(q5)))))) + KUKA_LBR_param_.dblLink6Mass*(cos(q1)*(sin(q3)*(KUKA_LBR_param_.dblLink6CogZ*cos(q5) + sin(q5)*(-(KUKA_LBR_param_.dblLink6CogX*cos(q6)) + KUKA_LBR_param_.dblLink6CogY*sin(q6))) + cos(q3)*(sin(q4)*(KUKA_LBR_param_.dblLink45Len + KUKA_LBR_param_.dblLink6CogY*cos(q6) + KUKA_LBR_param_.dblLink6CogX*sin(q6)) + cos(q4)*(KUKA_LBR_param_.dblLink6CogX*cos(q5)*cos(q6) + KUKA_LBR_param_.dblLink6CogZ*sin(q5) - KUKA_LBR_param_.dblLink6CogY*cos(q5)*sin(q6)))) + cos(q2)*sin(q1)*(cos(q3)*(KUKA_LBR_param_.dblLink6CogZ*cos(q5) + sin(q5)*(-(KUKA_LBR_param_.dblLink6CogX*cos(q6)) + KUKA_LBR_param_.dblLink6CogY*sin(q6))) - sin(q3)*(sin(q4)*(KUKA_LBR_param_.dblLink45Len + KUKA_LBR_param_.dblLink6CogY*cos(q6) + KUKA_LBR_param_.dblLink6CogX*sin(q6)) + cos(q4)*(KUKA_LBR_param_.dblLink6CogX*cos(q5)*cos(q6) + KUKA_LBR_param_.dblLink6CogZ*sin(q5) - KUKA_LBR_param_.dblLink6CogY*cos(q5)*sin(q6)))))*(sin(q1)*(cos(q3)*(KUKA_LBR_param_.dblLink6CogZ*cos(q5) + sin(q5)*(-(KUKA_LBR_param_.dblLink6CogX*cos(q6)) + KUKA_LBR_param_.dblLink6CogY*sin(q6))) - sin(q3)*(sin(q4)*(KUKA_LBR_param_.dblLink45Len + KUKA_LBR_param_.dblLink6CogY*cos(q6) + KUKA_LBR_param_.dblLink6CogX*sin(q6)) + cos(q4)*(KUKA_LBR_param_.dblLink6CogX*cos(q5)*cos(q6) + KUKA_LBR_param_.dblLink6CogZ*sin(q5) - KUKA_LBR_param_.dblLink6CogY*cos(q5)*sin(q6)))) + cos(q1)*(-(sin(q2)*(KUKA_LBR_param_.dblLink23Len - KUKA_LBR_param_.dblLink6CogX*cos(q5)*cos(q6)*sin(q4) - KUKA_LBR_param_.dblLink6CogZ*sin(q4)*sin(q5) + KUKA_LBR_param_.dblLink6CogY*cos(q5)*sin(q4)*sin(q6) + cos(q4)*(KUKA_LBR_param_.dblLink45Len + KUKA_LBR_param_.dblLink6CogY*cos(q6) + KUKA_LBR_param_.dblLink6CogX*sin(q6)))) + cos(q2)*(sin(q3)*(KUKA_LBR_param_.dblLink6CogZ*cos(q5) + sin(q5)*(-(KUKA_LBR_param_.dblLink6CogX*cos(q6)) + KUKA_LBR_param_.dblLink6CogY*sin(q6))) + cos(q3)*(sin(q4)*(KUKA_LBR_param_.dblLink45Len + KUKA_LBR_param_.dblLink6CogY*cos(q6) + KUKA_LBR_param_.dblLink6CogX*sin(q6)) + cos(q4)*(KUKA_LBR_param_.dblLink6CogX*cos(q5)*cos(q6) + KUKA_LBR_param_.dblLink6CogZ*sin(q5) - KUKA_LBR_param_.dblLink6CogY*cos(q5)*sin(q6)))))) + KUKA_LBR_param_.dblLink6Mass*(sin(q1)*(sin(q3)*(KUKA_LBR_param_.dblLink6CogZ*cos(q5) + sin(q5)*(-(KUKA_LBR_param_.dblLink6CogX*cos(q6)) + KUKA_LBR_param_.dblLink6CogY*sin(q6))) + cos(q3)*(sin(q4)*(KUKA_LBR_param_.dblLink45Len + KUKA_LBR_param_.dblLink6CogY*cos(q6) + KUKA_LBR_param_.dblLink6CogX*sin(q6)) + cos(q4)*(KUKA_LBR_param_.dblLink6CogX*cos(q5)*cos(q6) + KUKA_LBR_param_.dblLink6CogZ*sin(q5) - KUKA_LBR_param_.dblLink6CogY*cos(q5)*sin(q6)))) + cos(q1)*cos(q2)*(-(cos(q3)*(KUKA_LBR_param_.dblLink6CogZ*cos(q5) + sin(q5)*(-(KUKA_LBR_param_.dblLink6CogX*cos(q6)) + KUKA_LBR_param_.dblLink6CogY*sin(q6)))) + sin(q3)*(sin(q4)*(KUKA_LBR_param_.dblLink45Len + KUKA_LBR_param_.dblLink6CogY*cos(q6) + KUKA_LBR_param_.dblLink6CogX*sin(q6)) + cos(q4)*(KUKA_LBR_param_.dblLink6CogX*cos(q5)*cos(q6) + KUKA_LBR_param_.dblLink6CogZ*sin(q5) - KUKA_LBR_param_.dblLink6CogY*cos(q5)*sin(q6)))))*(cos(q1)*(-(cos(q3)*(KUKA_LBR_param_.dblLink6CogZ*cos(q5) + sin(q5)*(-(KUKA_LBR_param_.dblLink6CogX*cos(q6)) + KUKA_LBR_param_.dblLink6CogY*sin(q6)))) + sin(q3)*(sin(q4)*(KUKA_LBR_param_.dblLink45Len + KUKA_LBR_param_.dblLink6CogY*cos(q6) + KUKA_LBR_param_.dblLink6CogX*sin(q6)) + cos(q4)*(KUKA_LBR_param_.dblLink6CogX*cos(q5)*cos(q6) + KUKA_LBR_param_.dblLink6CogZ*sin(q5) - KUKA_LBR_param_.dblLink6CogY*cos(q5)*sin(q6)))) + sin(q1)*(-(sin(q2)*(KUKA_LBR_param_.dblLink23Len - KUKA_LBR_param_.dblLink6CogX*cos(q5)*cos(q6)*sin(q4) - KUKA_LBR_param_.dblLink6CogZ*sin(q4)*sin(q5) + KUKA_LBR_param_.dblLink6CogY*cos(q5)*sin(q4)*sin(q6) + cos(q4)*(KUKA_LBR_param_.dblLink45Len + KUKA_LBR_param_.dblLink6CogY*cos(q6) + KUKA_LBR_param_.dblLink6CogX*sin(q6)))) + cos(q2)*(sin(q3)*(KUKA_LBR_param_.dblLink6CogZ*cos(q5) + sin(q5)*(-(KUKA_LBR_param_.dblLink6CogX*cos(q6)) + KUKA_LBR_param_.dblLink6CogY*sin(q6))) + cos(q3)*(sin(q4)*(KUKA_LBR_param_.dblLink45Len + KUKA_LBR_param_.dblLink6CogY*cos(q6) + KUKA_LBR_param_.dblLink6CogX*sin(q6)) + cos(q4)*(KUKA_LBR_param_.dblLink6CogX*cos(q5)*cos(q6) + KUKA_LBR_param_.dblLink6CogZ*sin(q5) - KUKA_LBR_param_.dblLink6CogY*cos(q5)*sin(q6)))))) + KUKA_LBR_param_.dblLink7Mass*(sin(q1)*(-(sin(q3)*(cos(q5)*(KUKA_LBR_param_.dblLink7CogY*cos(q7) + KUKA_LBR_param_.dblLink7CogX*sin(q7)) + sin(q5)*(KUKA_LBR_param_.dblLink7CogX*cos(q6)*cos(q7) - KUKA_LBR_param_.dblLink7CogZ*sin(q6) - KUKA_LBR_param_.dblLink7CogY*cos(q6)*sin(q7)))) + cos(q3)*(sin(q4)*(KUKA_LBR_param_.dblLink45Len + KUKA_LBR_param_.dblLink7CogZ*cos(q6) + KUKA_LBR_param_.dblLink7CogX*cos(q7)*sin(q6) - KUKA_LBR_param_.dblLink7CogY*sin(q6)*sin(q7)) - cos(q4)*(sin(q5)*(KUKA_LBR_param_.dblLink7CogY*cos(q7) + KUKA_LBR_param_.dblLink7CogX*sin(q7)) + cos(q5)*(-(KUKA_LBR_param_.dblLink7CogX*cos(q6)*cos(q7)) + KUKA_LBR_param_.dblLink7CogZ*sin(q6) + KUKA_LBR_param_.dblLink7CogY*cos(q6)*sin(q7))))) + cos(q1)*cos(q2)*(cos(q3)*(cos(q5)*(KUKA_LBR_param_.dblLink7CogY*cos(q7) + KUKA_LBR_param_.dblLink7CogX*sin(q7)) + sin(q5)*(KUKA_LBR_param_.dblLink7CogX*cos(q6)*cos(q7) - KUKA_LBR_param_.dblLink7CogZ*sin(q6) - KUKA_LBR_param_.dblLink7CogY*cos(q6)*sin(q7))) + sin(q3)*(sin(q4)*(KUKA_LBR_param_.dblLink45Len + KUKA_LBR_param_.dblLink7CogZ*cos(q6) + KUKA_LBR_param_.dblLink7CogX*cos(q7)*sin(q6) - KUKA_LBR_param_.dblLink7CogY*sin(q6)*sin(q7)) - cos(q4)*(sin(q5)*(KUKA_LBR_param_.dblLink7CogY*cos(q7) + KUKA_LBR_param_.dblLink7CogX*sin(q7)) + cos(q5)*(-(KUKA_LBR_param_.dblLink7CogX*cos(q6)*cos(q7)) + KUKA_LBR_param_.dblLink7CogZ*sin(q6) + KUKA_LBR_param_.dblLink7CogY*cos(q6)*sin(q7))))))*(cos(q1)*(cos(q3)*(cos(q5)*(KUKA_LBR_param_.dblLink7CogY*cos(q7) + KUKA_LBR_param_.dblLink7CogX*sin(q7)) + sin(q5)*(KUKA_LBR_param_.dblLink7CogX*cos(q6)*cos(q7) - KUKA_LBR_param_.dblLink7CogZ*sin(q6) - KUKA_LBR_param_.dblLink7CogY*cos(q6)*sin(q7))) + sin(q3)*(sin(q4)*(KUKA_LBR_param_.dblLink45Len + KUKA_LBR_param_.dblLink7CogZ*cos(q6) + KUKA_LBR_param_.dblLink7CogX*cos(q7)*sin(q6) - KUKA_LBR_param_.dblLink7CogY*sin(q6)*sin(q7)) - cos(q4)*(sin(q5)*(KUKA_LBR_param_.dblLink7CogY*cos(q7) + KUKA_LBR_param_.dblLink7CogX*sin(q7)) + cos(q5)*(-(KUKA_LBR_param_.dblLink7CogX*cos(q6)*cos(q7)) + KUKA_LBR_param_.dblLink7CogZ*sin(q6) + KUKA_LBR_param_.dblLink7CogY*cos(q6)*sin(q7))))) + sin(q1)*(-(sin(q2)*(KUKA_LBR_param_.dblLink23Len + KUKA_LBR_param_.dblLink7CogY*cos(q7)*sin(q4)*sin(q5) + KUKA_LBR_param_.dblLink7CogX*sin(q4)*sin(q5)*sin(q7) + cos(q5)*sin(q4)*(-(KUKA_LBR_param_.dblLink7CogX*cos(q6)*cos(q7)) + KUKA_LBR_param_.dblLink7CogZ*sin(q6) + KUKA_LBR_param_.dblLink7CogY*cos(q6)*sin(q7)) + cos(q4)*(KUKA_LBR_param_.dblLink45Len + KUKA_LBR_param_.dblLink7CogZ*cos(q6) + KUKA_LBR_param_.dblLink7CogX*cos(q7)*sin(q6) - KUKA_LBR_param_.dblLink7CogY*sin(q6)*sin(q7)))) + cos(q2)*(-(sin(q3)*(cos(q5)*(KUKA_LBR_param_.dblLink7CogY*cos(q7) + KUKA_LBR_param_.dblLink7CogX*sin(q7)) + sin(q5)*(KUKA_LBR_param_.dblLink7CogX*cos(q6)*cos(q7) - KUKA_LBR_param_.dblLink7CogZ*sin(q6) - KUKA_LBR_param_.dblLink7CogY*cos(q6)*sin(q7)))) + cos(q3)*(sin(q4)*(KUKA_LBR_param_.dblLink45Len + KUKA_LBR_param_.dblLink7CogZ*cos(q6) + KUKA_LBR_param_.dblLink7CogX*cos(q7)*sin(q6) - KUKA_LBR_param_.dblLink7CogY*sin(q6)*sin(q7)) - cos(q4)*(sin(q5)*(KUKA_LBR_param_.dblLink7CogY*cos(q7) + KUKA_LBR_param_.dblLink7CogX*sin(q7)) + cos(q5)*(-(KUKA_LBR_param_.dblLink7CogX*cos(q6)*cos(q7)) + KUKA_LBR_param_.dblLink7CogZ*sin(q6) + KUKA_LBR_param_.dblLink7CogY*cos(q6)*sin(q7))))))) + KUKA_LBR_param_.dblLink7Mass*(cos(q2)*sin(q1)*(cos(q3)*(cos(q5)*(KUKA_LBR_param_.dblLink7CogY*cos(q7) + KUKA_LBR_param_.dblLink7CogX*sin(q7)) + sin(q5)*(KUKA_LBR_param_.dblLink7CogX*cos(q6)*cos(q7) - KUKA_LBR_param_.dblLink7CogZ*sin(q6) - KUKA_LBR_param_.dblLink7CogY*cos(q6)*sin(q7))) + sin(q3)*(sin(q4)*(KUKA_LBR_param_.dblLink45Len + KUKA_LBR_param_.dblLink7CogZ*cos(q6) + KUKA_LBR_param_.dblLink7CogX*cos(q7)*sin(q6) - KUKA_LBR_param_.dblLink7CogY*sin(q6)*sin(q7)) - cos(q4)*(sin(q5)*(KUKA_LBR_param_.dblLink7CogY*cos(q7) + KUKA_LBR_param_.dblLink7CogX*sin(q7)) + cos(q5)*(-(KUKA_LBR_param_.dblLink7CogX*cos(q6)*cos(q7)) + KUKA_LBR_param_.dblLink7CogZ*sin(q6) + KUKA_LBR_param_.dblLink7CogY*cos(q6)*sin(q7))))) + cos(q1)*(sin(q3)*(cos(q5)*(KUKA_LBR_param_.dblLink7CogY*cos(q7) + KUKA_LBR_param_.dblLink7CogX*sin(q7)) + sin(q5)*(KUKA_LBR_param_.dblLink7CogX*cos(q6)*cos(q7) - KUKA_LBR_param_.dblLink7CogZ*sin(q6) - KUKA_LBR_param_.dblLink7CogY*cos(q6)*sin(q7))) + cos(q3)*(-(sin(q4)*(KUKA_LBR_param_.dblLink45Len + KUKA_LBR_param_.dblLink7CogZ*cos(q6) + KUKA_LBR_param_.dblLink7CogX*cos(q7)*sin(q6) - KUKA_LBR_param_.dblLink7CogY*sin(q6)*sin(q7))) + cos(q4)*(sin(q5)*(KUKA_LBR_param_.dblLink7CogY*cos(q7) + KUKA_LBR_param_.dblLink7CogX*sin(q7)) + cos(q5)*(-(KUKA_LBR_param_.dblLink7CogX*cos(q6)*cos(q7)) + KUKA_LBR_param_.dblLink7CogZ*sin(q6) + KUKA_LBR_param_.dblLink7CogY*cos(q6)*sin(q7))))))*(sin(q1)*(cos(q3)*(cos(q5)*(KUKA_LBR_param_.dblLink7CogY*cos(q7) + KUKA_LBR_param_.dblLink7CogX*sin(q7)) + sin(q5)*(KUKA_LBR_param_.dblLink7CogX*cos(q6)*cos(q7) - KUKA_LBR_param_.dblLink7CogZ*sin(q6) - KUKA_LBR_param_.dblLink7CogY*cos(q6)*sin(q7))) + sin(q3)*(sin(q4)*(KUKA_LBR_param_.dblLink45Len + KUKA_LBR_param_.dblLink7CogZ*cos(q6) + KUKA_LBR_param_.dblLink7CogX*cos(q7)*sin(q6) - KUKA_LBR_param_.dblLink7CogY*sin(q6)*sin(q7)) - cos(q4)*(sin(q5)*(KUKA_LBR_param_.dblLink7CogY*cos(q7) + KUKA_LBR_param_.dblLink7CogX*sin(q7)) + cos(q5)*(-(KUKA_LBR_param_.dblLink7CogX*cos(q6)*cos(q7)) + KUKA_LBR_param_.dblLink7CogZ*sin(q6) + KUKA_LBR_param_.dblLink7CogY*cos(q6)*sin(q7))))) + cos(q1)*(sin(q2)*(KUKA_LBR_param_.dblLink23Len + KUKA_LBR_param_.dblLink7CogY*cos(q7)*sin(q4)*sin(q5) + KUKA_LBR_param_.dblLink7CogX*sin(q4)*sin(q5)*sin(q7) + cos(q5)*sin(q4)*(-(KUKA_LBR_param_.dblLink7CogX*cos(q6)*cos(q7)) + KUKA_LBR_param_.dblLink7CogZ*sin(q6) + KUKA_LBR_param_.dblLink7CogY*cos(q6)*sin(q7)) + cos(q4)*(KUKA_LBR_param_.dblLink45Len + KUKA_LBR_param_.dblLink7CogZ*cos(q6) + KUKA_LBR_param_.dblLink7CogX*cos(q7)*sin(q6) - KUKA_LBR_param_.dblLink7CogY*sin(q6)*sin(q7))) + cos(q2)*(sin(q3)*(cos(q5)*(KUKA_LBR_param_.dblLink7CogY*cos(q7) + KUKA_LBR_param_.dblLink7CogX*sin(q7)) + sin(q5)*(KUKA_LBR_param_.dblLink7CogX*cos(q6)*cos(q7) - KUKA_LBR_param_.dblLink7CogZ*sin(q6) - KUKA_LBR_param_.dblLink7CogY*cos(q6)*sin(q7))) + cos(q3)*(-(sin(q4)*(KUKA_LBR_param_.dblLink45Len + KUKA_LBR_param_.dblLink7CogZ*cos(q6) + KUKA_LBR_param_.dblLink7CogX*cos(q7)*sin(q6) - KUKA_LBR_param_.dblLink7CogY*sin(q6)*sin(q7))) + cos(q4)*(sin(q5)*(KUKA_LBR_param_.dblLink7CogY*cos(q7) + KUKA_LBR_param_.dblLink7CogX*sin(q7)) + cos(q5)*(-(KUKA_LBR_param_.dblLink7CogX*cos(q6)*cos(q7)) + KUKA_LBR_param_.dblLink7CogZ*sin(q6) + KUKA_LBR_param_.dblLink7CogY*cos(q6)*sin(q7)))))));
dblMassInertFullRow1Col4 = KUKA_LBR_param_.dblLink4InertXZ*cos(q3)*sin(q1) - KUKA_LBR_param_.dblLink4CogX*KUKA_LBR_param_.dblLink4CogZ*KUKA_LBR_param_.dblLink4Mass*cos(q3)*cos(q4)*sin(q2) - KUKA_LBR_param_.dblLink4InertZZ*sin(q2)*sin(q3) - power(KUKA_LBR_param_.dblLink4CogX,2)*KUKA_LBR_param_.dblLink4Mass*sin(q2)*sin(q3) - power(KUKA_LBR_param_.dblLink4CogY,2)*KUKA_LBR_param_.dblLink4Mass*sin(q2)*sin(q3) - KUKA_LBR_param_.dblLink7InertZZ*sin(q2)*sin(q3) + KUKA_LBR_param_.dblLink23Len*KUKA_LBR_param_.dblLink4CogY*KUKA_LBR_param_.dblLink4Mass*cos(q4)*sin(q2)*sin(q3) + cos(q1)*(-(KUKA_LBR_param_.dblLink4InertYZ*cos(q3)) + KUKA_LBR_param_.dblLink4InertXZ*cos(q2)*sin(q3)) + KUKA_LBR_param_.dblLink7InertXZ*(cos(q3)*sin(q1) + cos(q1)*cos(q2)*sin(q3)) + KUKA_LBR_param_.dblLink7InertYZ*(-(cos(q1)*cos(q3)) + cos(q2)*sin(q1)*sin(q3)) + KUKA_LBR_param_.dblLink4CogY*KUKA_LBR_param_.dblLink4CogZ*KUKA_LBR_param_.dblLink4Mass*cos(q3)*sin(q2)*sin(q4) + KUKA_LBR_param_.dblLink23Len*KUKA_LBR_param_.dblLink4CogX*KUKA_LBR_param_.dblLink4Mass*sin(q2)*sin(q3)*sin(q4) + cos(q2)*(KUKA_LBR_param_.dblLink4CogY*KUKA_LBR_param_.dblLink4CogZ*KUKA_LBR_param_.dblLink4Mass*cos(q4) + KUKA_LBR_param_.dblLink4InertYZ*sin(q1)*sin(q3) + KUKA_LBR_param_.dblLink4CogX*KUKA_LBR_param_.dblLink4CogZ*KUKA_LBR_param_.dblLink4Mass*sin(q4)) + (2*KUKA_LBR_param_.dblLink5InertXZ*cos(q3)*sin(q1) - 2*KUKA_LBR_param_.dblLink5CogX*KUKA_LBR_param_.dblLink5CogY*KUKA_LBR_param_.dblLink5Mass*cos(q3)*cos(q4)*power(cos(q5),2)*sin(q2) - 2*KUKA_LBR_param_.dblLink5InertZZ*sin(q2)*sin(q3) - 2*power(KUKA_LBR_param_.dblLink45Len,2)*KUKA_LBR_param_.dblLink5Mass*sin(q2)*sin(q3) - power(KUKA_LBR_param_.dblLink5CogX,2)*KUKA_LBR_param_.dblLink5Mass*sin(q2)*sin(q3) - power(KUKA_LBR_param_.dblLink5CogY,2)*KUKA_LBR_param_.dblLink5Mass*sin(q2)*sin(q3) - 4*KUKA_LBR_param_.dblLink45Len*KUKA_LBR_param_.dblLink5CogZ*KUKA_LBR_param_.dblLink5Mass*sin(q2)*sin(q3) - 2*power(KUKA_LBR_param_.dblLink5CogZ,2)*KUKA_LBR_param_.dblLink5Mass*sin(q2)*sin(q3) - 2*KUKA_LBR_param_.dblLink23Len*KUKA_LBR_param_.dblLink45Len*KUKA_LBR_param_.dblLink5Mass*cos(q4)*sin(q2)*sin(q3) - 2*KUKA_LBR_param_.dblLink23Len*KUKA_LBR_param_.dblLink5CogZ*KUKA_LBR_param_.dblLink5Mass*cos(q4)*sin(q2)*sin(q3) - power(KUKA_LBR_param_.dblLink5CogX,2)*KUKA_LBR_param_.dblLink5Mass*power(cos(q5),2)*sin(q2)*sin(q3) + power(KUKA_LBR_param_.dblLink5CogY,2)*KUKA_LBR_param_.dblLink5Mass*power(cos(q5),2)*sin(q2)*sin(q3) + cos(q1)*(-2*KUKA_LBR_param_.dblLink5InertYZ*cos(q3) + 2*KUKA_LBR_param_.dblLink5InertXZ*cos(q2)*sin(q3)) - 2*KUKA_LBR_param_.dblLink45Len*KUKA_LBR_param_.dblLink5CogY*KUKA_LBR_param_.dblLink5Mass*cos(q3)*cos(q5)*sin(q2)*sin(q4) - 2*KUKA_LBR_param_.dblLink5CogY*KUKA_LBR_param_.dblLink5CogZ*KUKA_LBR_param_.dblLink5Mass*cos(q3)*cos(q5)*sin(q2)*sin(q4) + 2*KUKA_LBR_param_.dblLink23Len*KUKA_LBR_param_.dblLink5CogX*KUKA_LBR_param_.dblLink5Mass*cos(q5)*sin(q2)*sin(q3)*sin(q4) - 2*power(KUKA_LBR_param_.dblLink5CogX,2)*KUKA_LBR_param_.dblLink5Mass*cos(q3)*cos(q4)*cos(q5)*sin(q2)*sin(q5) + 4*KUKA_LBR_param_.dblLink5CogX*KUKA_LBR_param_.dblLink5CogY*KUKA_LBR_param_.dblLink5Mass*cos(q5)*sin(q2)*sin(q3)*sin(q5) - 2*KUKA_LBR_param_.dblLink45Len*KUKA_LBR_param_.dblLink5CogX*KUKA_LBR_param_.dblLink5Mass*cos(q3)*sin(q2)*sin(q4)*sin(q5) - 2*KUKA_LBR_param_.dblLink5CogX*KUKA_LBR_param_.dblLink5CogZ*KUKA_LBR_param_.dblLink5Mass*cos(q3)*sin(q2)*sin(q4)*sin(q5) - 2*KUKA_LBR_param_.dblLink23Len*KUKA_LBR_param_.dblLink5CogY*KUKA_LBR_param_.dblLink5Mass*sin(q2)*sin(q3)*sin(q4)*sin(q5) + 2*KUKA_LBR_param_.dblLink5CogX*KUKA_LBR_param_.dblLink5CogY*KUKA_LBR_param_.dblLink5Mass*cos(q3)*cos(q4)*sin(q2)*power(sin(q5),2) + power(KUKA_LBR_param_.dblLink5CogX,2)*KUKA_LBR_param_.dblLink5Mass*sin(q2)*sin(q3)*power(sin(q5),2) - power(KUKA_LBR_param_.dblLink5CogY,2)*KUKA_LBR_param_.dblLink5Mass*sin(q2)*sin(q3)*power(sin(q5),2) + power(KUKA_LBR_param_.dblLink5CogY,2)*KUKA_LBR_param_.dblLink5Mass*cos(q3)*cos(q4)*sin(q2)*sin(2*q5) - cos(q2)*(-2*KUKA_LBR_param_.dblLink5InertYZ*sin(q1)*sin(q3) + 2*(KUKA_LBR_param_.dblLink45Len + KUKA_LBR_param_.dblLink5CogZ)*KUKA_LBR_param_.dblLink5Mass*cos(q4)*(KUKA_LBR_param_.dblLink5CogY*cos(q5) + KUKA_LBR_param_.dblLink5CogX*sin(q5)) + KUKA_LBR_param_.dblLink5Mass*sin(q4)*(-2*KUKA_LBR_param_.dblLink5CogX*KUKA_LBR_param_.dblLink5CogY*cos(2*q5) + (-power(KUKA_LBR_param_.dblLink5CogX,2) + power(KUKA_LBR_param_.dblLink5CogY,2))*sin(2*q5))))/2.0 + (4*KUKA_LBR_param_.dblLink6InertXZ*cos(q3)*sin(q1) + 4*KUKA_LBR_param_.dblLink6CogX*KUKA_LBR_param_.dblLink6CogZ*KUKA_LBR_param_.dblLink6Mass*cos(q3)*cos(q4)*power(cos(q5),2)*cos(q6)*sin(q2) - 4*KUKA_LBR_param_.dblLink6InertZZ*sin(q2)*sin(q3) - 4*power(KUKA_LBR_param_.dblLink45Len,2)*KUKA_LBR_param_.dblLink6Mass*sin(q2)*sin(q3) - 3*power(KUKA_LBR_param_.dblLink6CogX,2)*KUKA_LBR_param_.dblLink6Mass*sin(q2)*sin(q3) - 3*power(KUKA_LBR_param_.dblLink6CogY,2)*KUKA_LBR_param_.dblLink6Mass*sin(q2)*sin(q3) - 2*power(KUKA_LBR_param_.dblLink6CogZ,2)*KUKA_LBR_param_.dblLink6Mass*sin(q2)*sin(q3) - 4*KUKA_LBR_param_.dblLink23Len*KUKA_LBR_param_.dblLink45Len*KUKA_LBR_param_.dblLink6Mass*cos(q4)*sin(q2)*sin(q3) - power(KUKA_LBR_param_.dblLink6CogX,2)*KUKA_LBR_param_.dblLink6Mass*power(cos(q5),2)*sin(q2)*sin(q3) - power(KUKA_LBR_param_.dblLink6CogY,2)*KUKA_LBR_param_.dblLink6Mass*power(cos(q5),2)*sin(q2)*sin(q3) + 2*power(KUKA_LBR_param_.dblLink6CogZ,2)*KUKA_LBR_param_.dblLink6Mass*power(cos(q5),2)*sin(q2)*sin(q3) - 8*KUKA_LBR_param_.dblLink45Len*KUKA_LBR_param_.dblLink6CogY*KUKA_LBR_param_.dblLink6Mass*cos(q6)*sin(q2)*sin(q3) - 4*KUKA_LBR_param_.dblLink23Len*KUKA_LBR_param_.dblLink6CogY*KUKA_LBR_param_.dblLink6Mass*cos(q4)*cos(q6)*sin(q2)*sin(q3) + power(KUKA_LBR_param_.dblLink6CogX,2)*KUKA_LBR_param_.dblLink6Mass*power(cos(q6),2)*sin(q2)*sin(q3) - power(KUKA_LBR_param_.dblLink6CogY,2)*KUKA_LBR_param_.dblLink6Mass*power(cos(q6),2)*sin(q2)*sin(q3) - power(KUKA_LBR_param_.dblLink6CogX,2)*KUKA_LBR_param_.dblLink6Mass*power(cos(q5),2)*power(cos(q6),2)*sin(q2)*sin(q3) + power(KUKA_LBR_param_.dblLink6CogY,2)*KUKA_LBR_param_.dblLink6Mass*power(cos(q5),2)*power(cos(q6),2)*sin(q2)*sin(q3) + cos(q1)*(-4*KUKA_LBR_param_.dblLink6InertYZ*cos(q3) + 4*KUKA_LBR_param_.dblLink6InertXZ*cos(q2)*sin(q3)) + 4*KUKA_LBR_param_.dblLink45Len*KUKA_LBR_param_.dblLink6CogZ*KUKA_LBR_param_.dblLink6Mass*cos(q3)*cos(q5)*sin(q2)*sin(q4) + 4*KUKA_LBR_param_.dblLink6CogY*KUKA_LBR_param_.dblLink6CogZ*KUKA_LBR_param_.dblLink6Mass*cos(q3)*cos(q5)*cos(q6)*sin(q2)*sin(q4) + 4*KUKA_LBR_param_.dblLink23Len*KUKA_LBR_param_.dblLink6CogX*KUKA_LBR_param_.dblLink6Mass*cos(q5)*cos(q6)*sin(q2)*sin(q3)*sin(q4) - 2*power(KUKA_LBR_param_.dblLink6CogX,2)*KUKA_LBR_param_.dblLink6Mass*cos(q3)*cos(q4)*cos(q5)*sin(q2)*sin(q5) - 2*power(KUKA_LBR_param_.dblLink6CogY,2)*KUKA_LBR_param_.dblLink6Mass*cos(q3)*cos(q4)*cos(q5)*sin(q2)*sin(q5) + 4*power(KUKA_LBR_param_.dblLink6CogZ,2)*KUKA_LBR_param_.dblLink6Mass*cos(q3)*cos(q4)*cos(q5)*sin(q2)*sin(q5) - 2*power(KUKA_LBR_param_.dblLink6CogX,2)*KUKA_LBR_param_.dblLink6Mass*cos(q3)*cos(q4)*cos(q5)*power(cos(q6),2)*sin(q2)*sin(q5) - 8*KUKA_LBR_param_.dblLink6CogX*KUKA_LBR_param_.dblLink6CogZ*KUKA_LBR_param_.dblLink6Mass*cos(q5)*cos(q6)*sin(q2)*sin(q3)*sin(q5) - 4*KUKA_LBR_param_.dblLink45Len*KUKA_LBR_param_.dblLink6CogX*KUKA_LBR_param_.dblLink6Mass*cos(q3)*cos(q6)*sin(q2)*sin(q4)*sin(q5) - 4*KUKA_LBR_param_.dblLink6CogX*KUKA_LBR_param_.dblLink6CogY*KUKA_LBR_param_.dblLink6Mass*cos(q3)*power(cos(q6),2)*sin(q2)*sin(q4)*sin(q5) + 4*KUKA_LBR_param_.dblLink23Len*KUKA_LBR_param_.dblLink6CogZ*KUKA_LBR_param_.dblLink6Mass*sin(q2)*sin(q3)*sin(q4)*sin(q5) - 4*KUKA_LBR_param_.dblLink6CogX*KUKA_LBR_param_.dblLink6CogZ*KUKA_LBR_param_.dblLink6Mass*cos(q3)*cos(q4)*cos(q6)*sin(q2)*power(sin(q5),2) + power(KUKA_LBR_param_.dblLink6CogX,2)*KUKA_LBR_param_.dblLink6Mass*sin(q2)*sin(q3)*power(sin(q5),2) + power(KUKA_LBR_param_.dblLink6CogY,2)*KUKA_LBR_param_.dblLink6Mass*sin(q2)*sin(q3)*power(sin(q5),2) - 2*power(KUKA_LBR_param_.dblLink6CogZ,2)*KUKA_LBR_param_.dblLink6Mass*sin(q2)*sin(q3)*power(sin(q5),2) + power(KUKA_LBR_param_.dblLink6CogX,2)*KUKA_LBR_param_.dblLink6Mass*power(cos(q6),2)*sin(q2)*sin(q3)*power(sin(q5),2) - power(KUKA_LBR_param_.dblLink6CogY,2)*KUKA_LBR_param_.dblLink6Mass*power(cos(q6),2)*sin(q2)*sin(q3)*power(sin(q5),2) + power(KUKA_LBR_param_.dblLink6CogY,2)*KUKA_LBR_param_.dblLink6Mass*cos(q3)*cos(q4)*power(cos(q6),2)*sin(q2)*sin(2*q5) - 4*KUKA_LBR_param_.dblLink6CogY*KUKA_LBR_param_.dblLink6CogZ*KUKA_LBR_param_.dblLink6Mass*cos(q3)*cos(q4)*power(cos(q5),2)*sin(q2)*sin(q6) - 8*KUKA_LBR_param_.dblLink45Len*KUKA_LBR_param_.dblLink6CogX*KUKA_LBR_param_.dblLink6Mass*sin(q2)*sin(q3)*sin(q6) - 4*KUKA_LBR_param_.dblLink23Len*KUKA_LBR_param_.dblLink6CogX*KUKA_LBR_param_.dblLink6Mass*cos(q4)*sin(q2)*sin(q3)*sin(q6) - 4*KUKA_LBR_param_.dblLink6CogX*KUKA_LBR_param_.dblLink6CogY*KUKA_LBR_param_.dblLink6Mass*cos(q6)*sin(q2)*sin(q3)*sin(q6) + 4*KUKA_LBR_param_.dblLink6CogX*KUKA_LBR_param_.dblLink6CogY*KUKA_LBR_param_.dblLink6Mass*power(cos(q5),2)*cos(q6)*sin(q2)*sin(q3)*sin(q6) + 4*KUKA_LBR_param_.dblLink6CogX*KUKA_LBR_param_.dblLink6CogZ*KUKA_LBR_param_.dblLink6Mass*cos(q3)*cos(q5)*sin(q2)*sin(q4)*sin(q6) - 4*KUKA_LBR_param_.dblLink23Len*KUKA_LBR_param_.dblLink6CogY*KUKA_LBR_param_.dblLink6Mass*cos(q5)*sin(q2)*sin(q3)*sin(q4)*sin(q6) + 8*KUKA_LBR_param_.dblLink6CogX*KUKA_LBR_param_.dblLink6CogY*KUKA_LBR_param_.dblLink6Mass*cos(q3)*cos(q4)*cos(q5)*cos(q6)*sin(q2)*sin(q5)*sin(q6) + 8*KUKA_LBR_param_.dblLink6CogY*KUKA_LBR_param_.dblLink6CogZ*KUKA_LBR_param_.dblLink6Mass*cos(q5)*sin(q2)*sin(q3)*sin(q5)*sin(q6) + 4*KUKA_LBR_param_.dblLink45Len*KUKA_LBR_param_.dblLink6CogY*KUKA_LBR_param_.dblLink6Mass*cos(q3)*sin(q2)*sin(q4)*sin(q5)*sin(q6) - 4*power(KUKA_LBR_param_.dblLink6CogX,2)*KUKA_LBR_param_.dblLink6Mass*cos(q3)*cos(q6)*sin(q2)*sin(q4)*sin(q5)*sin(q6) + 4*power(KUKA_LBR_param_.dblLink6CogY,2)*KUKA_LBR_param_.dblLink6Mass*cos(q3)*cos(q6)*sin(q2)*sin(q4)*sin(q5)*sin(q6) + 4*KUKA_LBR_param_.dblLink6CogY*KUKA_LBR_param_.dblLink6CogZ*KUKA_LBR_param_.dblLink6Mass*cos(q3)*cos(q4)*sin(q2)*power(sin(q5),2)*sin(q6) - 4*KUKA_LBR_param_.dblLink6CogX*KUKA_LBR_param_.dblLink6CogY*KUKA_LBR_param_.dblLink6Mass*cos(q6)*sin(q2)*sin(q3)*power(sin(q5),2)*sin(q6) - power(KUKA_LBR_param_.dblLink6CogX,2)*KUKA_LBR_param_.dblLink6Mass*sin(q2)*sin(q3)*power(sin(q6),2) + power(KUKA_LBR_param_.dblLink6CogY,2)*KUKA_LBR_param_.dblLink6Mass*sin(q2)*sin(q3)*power(sin(q6),2) + power(KUKA_LBR_param_.dblLink6CogX,2)*KUKA_LBR_param_.dblLink6Mass*power(cos(q5),2)*sin(q2)*sin(q3)*power(sin(q6),2) - power(KUKA_LBR_param_.dblLink6CogY,2)*KUKA_LBR_param_.dblLink6Mass*power(cos(q5),2)*sin(q2)*sin(q3)*power(sin(q6),2) - 2*power(KUKA_LBR_param_.dblLink6CogY,2)*KUKA_LBR_param_.dblLink6Mass*cos(q3)*cos(q4)*cos(q5)*sin(q2)*sin(q5)*power(sin(q6),2) + 4*KUKA_LBR_param_.dblLink6CogX*KUKA_LBR_param_.dblLink6CogY*KUKA_LBR_param_.dblLink6Mass*cos(q3)*sin(q2)*sin(q4)*sin(q5)*power(sin(q6),2) - power(KUKA_LBR_param_.dblLink6CogX,2)*KUKA_LBR_param_.dblLink6Mass*sin(q2)*sin(q3)*power(sin(q5),2)*power(sin(q6),2) + power(KUKA_LBR_param_.dblLink6CogY,2)*KUKA_LBR_param_.dblLink6Mass*sin(q2)*sin(q3)*power(sin(q5),2)*power(sin(q6),2) + power(KUKA_LBR_param_.dblLink6CogX,2)*KUKA_LBR_param_.dblLink6Mass*cos(q3)*cos(q4)*sin(q2)*sin(2*q5)*power(sin(q6),2) + cos(q2)*(4*KUKA_LBR_param_.dblLink6InertYZ*sin(q1)*sin(q3) + 4*KUKA_LBR_param_.dblLink6Mass*cos(q4)*(KUKA_LBR_param_.dblLink45Len + KUKA_LBR_param_.dblLink6CogY*cos(q6) + KUKA_LBR_param_.dblLink6CogX*sin(q6))*(KUKA_LBR_param_.dblLink6CogZ*cos(q5) + sin(q5)*(-(KUKA_LBR_param_.dblLink6CogX*cos(q6)) + KUKA_LBR_param_.dblLink6CogY*sin(q6))) + KUKA_LBR_param_.dblLink6Mass*sin(q4)*(4*KUKA_LBR_param_.dblLink6CogX*KUKA_LBR_param_.dblLink6CogZ*cos(q6)*power(sin(q5),2) + power(KUKA_LBR_param_.dblLink6CogX,2)*sin(2*q5) + power(KUKA_LBR_param_.dblLink6CogY,2)*sin(2*q5) + power(KUKA_LBR_param_.dblLink6CogX,2)*power(cos(q6),2)*sin(2*q5) - 4*KUKA_LBR_param_.dblLink6CogY*KUKA_LBR_param_.dblLink6CogZ*power(sin(q5),2)*sin(q6) + power(KUKA_LBR_param_.dblLink6CogY,2)*sin(2*q5)*power(sin(q6),2) - 4*KUKA_LBR_param_.dblLink6CogZ*power(cos(q5),2)*(KUKA_LBR_param_.dblLink6CogX*cos(q6) - KUKA_LBR_param_.dblLink6CogY*sin(q6)) - 2*cos(q5)*sin(q5)*(2*power(KUKA_LBR_param_.dblLink6CogZ,2) + power(KUKA_LBR_param_.dblLink6CogY,2)*power(cos(q6),2) + 4*KUKA_LBR_param_.dblLink6CogX*KUKA_LBR_param_.dblLink6CogY*cos(q6)*sin(q6) + power(KUKA_LBR_param_.dblLink6CogX,2)*power(sin(q6),2)))))/4.0 + KUKA_LBR_param_.dblLink7Mass*(cos(q4)*(-(sin(q1)*sin(q2)*sin(q5)*(KUKA_LBR_param_.dblLink7CogY*cos(q7) + KUKA_LBR_param_.dblLink7CogX*sin(q7))) + cos(q1)*sin(q3)*(KUKA_LBR_param_.dblLink45Len + KUKA_LBR_param_.dblLink7CogZ*cos(q6) + KUKA_LBR_param_.dblLink7CogX*cos(q7)*sin(q6) - KUKA_LBR_param_.dblLink7CogY*sin(q6)*sin(q7)) - cos(q5)*sin(q1)*sin(q2)*(KUKA_LBR_param_.dblLink7CogZ*sin(q6) + cos(q6)*(-(KUKA_LBR_param_.dblLink7CogX*cos(q7)) + KUKA_LBR_param_.dblLink7CogY*sin(q7)))) + sin(q4)*(sin(q1)*sin(q2)*(KUKA_LBR_param_.dblLink45Len + KUKA_LBR_param_.dblLink7CogZ*cos(q6) + KUKA_LBR_param_.dblLink7CogX*cos(q7)*sin(q6) - KUKA_LBR_param_.dblLink7CogY*sin(q6)*sin(q7)) + cos(q1)*sin(q3)*(sin(q5)*(KUKA_LBR_param_.dblLink7CogY*cos(q7) + KUKA_LBR_param_.dblLink7CogX*sin(q7)) + cos(q5)*(-(KUKA_LBR_param_.dblLink7CogX*cos(q6)*cos(q7)) + KUKA_LBR_param_.dblLink7CogZ*sin(q6) + KUKA_LBR_param_.dblLink7CogY*cos(q6)*sin(q7)))) + cos(q2)*cos(q3)*sin(q1)*(cos(q4)*(KUKA_LBR_param_.dblLink45Len + KUKA_LBR_param_.dblLink7CogZ*cos(q6) + KUKA_LBR_param_.dblLink7CogX*cos(q7)*sin(q6) - KUKA_LBR_param_.dblLink7CogY*sin(q6)*sin(q7)) + sin(q4)*(sin(q5)*(KUKA_LBR_param_.dblLink7CogY*cos(q7) + KUKA_LBR_param_.dblLink7CogX*sin(q7)) + cos(q5)*(-(KUKA_LBR_param_.dblLink7CogX*cos(q6)*cos(q7)) + KUKA_LBR_param_.dblLink7CogZ*sin(q6) + KUKA_LBR_param_.dblLink7CogY*cos(q6)*sin(q7)))))*(sin(q1)*(-(cos(q3)*(cos(q5)*(KUKA_LBR_param_.dblLink7CogY*cos(q7) + KUKA_LBR_param_.dblLink7CogX*sin(q7)) + sin(q5)*(KUKA_LBR_param_.dblLink7CogX*cos(q6)*cos(q7) - KUKA_LBR_param_.dblLink7CogZ*sin(q6) - KUKA_LBR_param_.dblLink7CogY*cos(q6)*sin(q7)))) + sin(q3)*(-(sin(q4)*(KUKA_LBR_param_.dblLink45Len + KUKA_LBR_param_.dblLink7CogZ*cos(q6) + KUKA_LBR_param_.dblLink7CogX*cos(q7)*sin(q6) - KUKA_LBR_param_.dblLink7CogY*sin(q6)*sin(q7))) + cos(q4)*(sin(q5)*(KUKA_LBR_param_.dblLink7CogY*cos(q7) + KUKA_LBR_param_.dblLink7CogX*sin(q7)) + cos(q5)*(-(KUKA_LBR_param_.dblLink7CogX*cos(q6)*cos(q7)) + KUKA_LBR_param_.dblLink7CogZ*sin(q6) + KUKA_LBR_param_.dblLink7CogY*cos(q6)*sin(q7))))) + cos(q1)*(-(sin(q2)*(KUKA_LBR_param_.dblLink23Len + KUKA_LBR_param_.dblLink7CogY*cos(q7)*sin(q4)*sin(q5) + KUKA_LBR_param_.dblLink7CogX*sin(q4)*sin(q5)*sin(q7) + cos(q5)*sin(q4)*(-(KUKA_LBR_param_.dblLink7CogX*cos(q6)*cos(q7)) + KUKA_LBR_param_.dblLink7CogZ*sin(q6) + KUKA_LBR_param_.dblLink7CogY*cos(q6)*sin(q7)) + cos(q4)*(KUKA_LBR_param_.dblLink45Len + KUKA_LBR_param_.dblLink7CogZ*cos(q6) + KUKA_LBR_param_.dblLink7CogX*cos(q7)*sin(q6) - KUKA_LBR_param_.dblLink7CogY*sin(q6)*sin(q7)))) + cos(q2)*(-(sin(q3)*(cos(q5)*(KUKA_LBR_param_.dblLink7CogY*cos(q7) + KUKA_LBR_param_.dblLink7CogX*sin(q7)) + sin(q5)*(KUKA_LBR_param_.dblLink7CogX*cos(q6)*cos(q7) - KUKA_LBR_param_.dblLink7CogZ*sin(q6) - KUKA_LBR_param_.dblLink7CogY*cos(q6)*sin(q7)))) + cos(q3)*(sin(q4)*(KUKA_LBR_param_.dblLink45Len + KUKA_LBR_param_.dblLink7CogZ*cos(q6) + KUKA_LBR_param_.dblLink7CogX*cos(q7)*sin(q6) - KUKA_LBR_param_.dblLink7CogY*sin(q6)*sin(q7)) - cos(q4)*(sin(q5)*(KUKA_LBR_param_.dblLink7CogY*cos(q7) + KUKA_LBR_param_.dblLink7CogX*sin(q7)) + cos(q5)*(-(KUKA_LBR_param_.dblLink7CogX*cos(q6)*cos(q7)) + KUKA_LBR_param_.dblLink7CogZ*sin(q6) + KUKA_LBR_param_.dblLink7CogY*cos(q6)*sin(q7))))))) + KUKA_LBR_param_.dblLink7Mass*(sin(q1)*sin(q3)*(cos(q4)*(KUKA_LBR_param_.dblLink45Len + KUKA_LBR_param_.dblLink7CogZ*cos(q6) + KUKA_LBR_param_.dblLink7CogX*cos(q7)*sin(q6) - KUKA_LBR_param_.dblLink7CogY*sin(q6)*sin(q7)) + sin(q4)*(sin(q5)*(KUKA_LBR_param_.dblLink7CogY*cos(q7) + KUKA_LBR_param_.dblLink7CogX*sin(q7)) + cos(q5)*(-(KUKA_LBR_param_.dblLink7CogX*cos(q6)*cos(q7)) + KUKA_LBR_param_.dblLink7CogZ*sin(q6) + KUKA_LBR_param_.dblLink7CogY*cos(q6)*sin(q7)))) - cos(q1)*(sin(q2)*(sin(q4)*(KUKA_LBR_param_.dblLink45Len + KUKA_LBR_param_.dblLink7CogZ*cos(q6) + KUKA_LBR_param_.dblLink7CogX*cos(q7)*sin(q6) - KUKA_LBR_param_.dblLink7CogY*sin(q6)*sin(q7)) - cos(q4)*(sin(q5)*(KUKA_LBR_param_.dblLink7CogY*cos(q7) + KUKA_LBR_param_.dblLink7CogX*sin(q7)) + cos(q5)*(-(KUKA_LBR_param_.dblLink7CogX*cos(q6)*cos(q7)) + KUKA_LBR_param_.dblLink7CogZ*sin(q6) + KUKA_LBR_param_.dblLink7CogY*cos(q6)*sin(q7)))) + cos(q2)*cos(q3)*(cos(q4)*(KUKA_LBR_param_.dblLink45Len + KUKA_LBR_param_.dblLink7CogZ*cos(q6) + KUKA_LBR_param_.dblLink7CogX*cos(q7)*sin(q6) - KUKA_LBR_param_.dblLink7CogY*sin(q6)*sin(q7)) + sin(q4)*(sin(q5)*(KUKA_LBR_param_.dblLink7CogY*cos(q7) + KUKA_LBR_param_.dblLink7CogX*sin(q7)) + cos(q5)*(-(KUKA_LBR_param_.dblLink7CogX*cos(q6)*cos(q7)) + KUKA_LBR_param_.dblLink7CogZ*sin(q6) + KUKA_LBR_param_.dblLink7CogY*cos(q6)*sin(q7))))))*(cos(q1)*(cos(q3)*(cos(q5)*(KUKA_LBR_param_.dblLink7CogY*cos(q7) + KUKA_LBR_param_.dblLink7CogX*sin(q7)) + sin(q5)*(KUKA_LBR_param_.dblLink7CogX*cos(q6)*cos(q7) - KUKA_LBR_param_.dblLink7CogZ*sin(q6) - KUKA_LBR_param_.dblLink7CogY*cos(q6)*sin(q7))) + sin(q3)*(sin(q4)*(KUKA_LBR_param_.dblLink45Len + KUKA_LBR_param_.dblLink7CogZ*cos(q6) + KUKA_LBR_param_.dblLink7CogX*cos(q7)*sin(q6) - KUKA_LBR_param_.dblLink7CogY*sin(q6)*sin(q7)) - cos(q4)*(sin(q5)*(KUKA_LBR_param_.dblLink7CogY*cos(q7) + KUKA_LBR_param_.dblLink7CogX*sin(q7)) + cos(q5)*(-(KUKA_LBR_param_.dblLink7CogX*cos(q6)*cos(q7)) + KUKA_LBR_param_.dblLink7CogZ*sin(q6) + KUKA_LBR_param_.dblLink7CogY*cos(q6)*sin(q7))))) + sin(q1)*(-(sin(q2)*(KUKA_LBR_param_.dblLink23Len + KUKA_LBR_param_.dblLink7CogY*cos(q7)*sin(q4)*sin(q5) + KUKA_LBR_param_.dblLink7CogX*sin(q4)*sin(q5)*sin(q7) + cos(q5)*sin(q4)*(-(KUKA_LBR_param_.dblLink7CogX*cos(q6)*cos(q7)) + KUKA_LBR_param_.dblLink7CogZ*sin(q6) + KUKA_LBR_param_.dblLink7CogY*cos(q6)*sin(q7)) + cos(q4)*(KUKA_LBR_param_.dblLink45Len + KUKA_LBR_param_.dblLink7CogZ*cos(q6) + KUKA_LBR_param_.dblLink7CogX*cos(q7)*sin(q6) - KUKA_LBR_param_.dblLink7CogY*sin(q6)*sin(q7)))) + cos(q2)*(-(sin(q3)*(cos(q5)*(KUKA_LBR_param_.dblLink7CogY*cos(q7) + KUKA_LBR_param_.dblLink7CogX*sin(q7)) + sin(q5)*(KUKA_LBR_param_.dblLink7CogX*cos(q6)*cos(q7) - KUKA_LBR_param_.dblLink7CogZ*sin(q6) - KUKA_LBR_param_.dblLink7CogY*cos(q6)*sin(q7)))) + cos(q3)*(sin(q4)*(KUKA_LBR_param_.dblLink45Len + KUKA_LBR_param_.dblLink7CogZ*cos(q6) + KUKA_LBR_param_.dblLink7CogX*cos(q7)*sin(q6) - KUKA_LBR_param_.dblLink7CogY*sin(q6)*sin(q7)) - cos(q4)*(sin(q5)*(KUKA_LBR_param_.dblLink7CogY*cos(q7) + KUKA_LBR_param_.dblLink7CogX*sin(q7)) + cos(q5)*(-(KUKA_LBR_param_.dblLink7CogX*cos(q6)*cos(q7)) + KUKA_LBR_param_.dblLink7CogZ*sin(q6) + KUKA_LBR_param_.dblLink7CogY*cos(q6)*sin(q7)))))));
dblMassInertFullRow1Col5 = -(KUKA_LBR_param_.dblLink23Len*KUKA_LBR_param_.dblLink5CogX*KUKA_LBR_param_.dblLink5Mass*cos(q3)*cos(q5)*sin(q2)) - KUKA_LBR_param_.dblLink45Len*KUKA_LBR_param_.dblLink5CogX*KUKA_LBR_param_.dblLink5Mass*cos(q3)*cos(q4)*cos(q5)*sin(q2) - KUKA_LBR_param_.dblLink5CogX*KUKA_LBR_param_.dblLink5CogZ*KUKA_LBR_param_.dblLink5Mass*cos(q3)*cos(q4)*cos(q5)*sin(q2) + KUKA_LBR_param_.dblLink5InertYZ*cos(q4)*sin(q1)*sin(q2) + KUKA_LBR_param_.dblLink45Len*KUKA_LBR_param_.dblLink5CogY*KUKA_LBR_param_.dblLink5Mass*cos(q5)*sin(q2)*sin(q3) + KUKA_LBR_param_.dblLink5CogY*KUKA_LBR_param_.dblLink5CogZ*KUKA_LBR_param_.dblLink5Mass*cos(q5)*sin(q2)*sin(q3) + KUKA_LBR_param_.dblLink23Len*KUKA_LBR_param_.dblLink5CogY*KUKA_LBR_param_.dblLink5Mass*cos(q4)*cos(q5)*sin(q2)*sin(q3) + KUKA_LBR_param_.dblLink5InertZZ*cos(q3)*sin(q2)*sin(q4) + power(KUKA_LBR_param_.dblLink5CogX,2)*KUKA_LBR_param_.dblLink5Mass*cos(q3)*sin(q2)*sin(q4) + power(KUKA_LBR_param_.dblLink5CogY,2)*KUKA_LBR_param_.dblLink5Mass*cos(q3)*sin(q2)*sin(q4) + KUKA_LBR_param_.dblLink5InertXZ*sin(q1)*sin(q3)*sin(q4) + KUKA_LBR_param_.dblLink7InertZZ*(cos(q2)*cos(q4) + cos(q3)*sin(q2)*sin(q4)) + cos(q1)*(KUKA_LBR_param_.dblLink5InertXZ*cos(q4)*sin(q2) - KUKA_LBR_param_.dblLink5InertYZ*sin(q3)*sin(q4)) + KUKA_LBR_param_.dblLink7InertYZ*(cos(q4)*sin(q1)*sin(q2) - (cos(q2)*cos(q3)*sin(q1) + cos(q1)*sin(q3))*sin(q4)) + KUKA_LBR_param_.dblLink7InertXZ*(sin(q1)*sin(q3)*sin(q4) + cos(q1)*(cos(q4)*sin(q2) - cos(q2)*cos(q3)*sin(q4))) + KUKA_LBR_param_.dblLink23Len*KUKA_LBR_param_.dblLink5CogY*KUKA_LBR_param_.dblLink5Mass*cos(q3)*sin(q2)*sin(q5) + KUKA_LBR_param_.dblLink45Len*KUKA_LBR_param_.dblLink5CogY*KUKA_LBR_param_.dblLink5Mass*cos(q3)*cos(q4)*sin(q2)*sin(q5) + KUKA_LBR_param_.dblLink5CogY*KUKA_LBR_param_.dblLink5CogZ*KUKA_LBR_param_.dblLink5Mass*cos(q3)*cos(q4)*sin(q2)*sin(q5) + KUKA_LBR_param_.dblLink45Len*KUKA_LBR_param_.dblLink5CogX*KUKA_LBR_param_.dblLink5Mass*sin(q2)*sin(q3)*sin(q5) + KUKA_LBR_param_.dblLink5CogX*KUKA_LBR_param_.dblLink5CogZ*KUKA_LBR_param_.dblLink5Mass*sin(q2)*sin(q3)*sin(q5) + KUKA_LBR_param_.dblLink23Len*KUKA_LBR_param_.dblLink5CogX*KUKA_LBR_param_.dblLink5Mass*cos(q4)*sin(q2)*sin(q3)*sin(q5) + cos(q2)*((KUKA_LBR_param_.dblLink5InertZZ + (power(KUKA_LBR_param_.dblLink5CogX,2) + power(KUKA_LBR_param_.dblLink5CogY,2))*KUKA_LBR_param_.dblLink5Mass)*cos(q4) - sin(q4)*(KUKA_LBR_param_.dblLink5InertXZ*cos(q1)*cos(q3) - KUKA_LBR_param_.dblLink5CogX*(KUKA_LBR_param_.dblLink45Len + KUKA_LBR_param_.dblLink5CogZ)*KUKA_LBR_param_.dblLink5Mass*cos(q5) + KUKA_LBR_param_.dblLink5InertYZ*cos(q3)*sin(q1) + KUKA_LBR_param_.dblLink45Len*KUKA_LBR_param_.dblLink5CogY*KUKA_LBR_param_.dblLink5Mass*sin(q5) + KUKA_LBR_param_.dblLink5CogY*KUKA_LBR_param_.dblLink5CogZ*KUKA_LBR_param_.dblLink5Mass*sin(q5))) + (-2*KUKA_LBR_param_.dblLink23Len*KUKA_LBR_param_.dblLink6CogX*KUKA_LBR_param_.dblLink6Mass*cos(q3)*cos(q5)*cos(q6)*sin(q2) - 2*KUKA_LBR_param_.dblLink45Len*KUKA_LBR_param_.dblLink6CogX*KUKA_LBR_param_.dblLink6Mass*cos(q3)*cos(q4)*cos(q5)*cos(q6)*sin(q2) - 2*KUKA_LBR_param_.dblLink6CogX*KUKA_LBR_param_.dblLink6CogY*KUKA_LBR_param_.dblLink6Mass*cos(q3)*cos(q4)*cos(q5)*power(cos(q6),2)*sin(q2) + 2*KUKA_LBR_param_.dblLink6InertYZ*cos(q4)*sin(q1)*sin(q2) - 2*KUKA_LBR_param_.dblLink45Len*KUKA_LBR_param_.dblLink6CogZ*KUKA_LBR_param_.dblLink6Mass*cos(q5)*sin(q2)*sin(q3) - 2*KUKA_LBR_param_.dblLink23Len*KUKA_LBR_param_.dblLink6CogZ*KUKA_LBR_param_.dblLink6Mass*cos(q4)*cos(q5)*sin(q2)*sin(q3) - 2*KUKA_LBR_param_.dblLink6CogY*KUKA_LBR_param_.dblLink6CogZ*KUKA_LBR_param_.dblLink6Mass*cos(q5)*cos(q6)*sin(q2)*sin(q3) + 2*KUKA_LBR_param_.dblLink6InertZZ*cos(q3)*sin(q2)*sin(q4) + power(KUKA_LBR_param_.dblLink6CogX,2)*KUKA_LBR_param_.dblLink6Mass*cos(q3)*sin(q2)*sin(q4) + power(KUKA_LBR_param_.dblLink6CogY,2)*KUKA_LBR_param_.dblLink6Mass*cos(q3)*sin(q2)*sin(q4) + 2*power(KUKA_LBR_param_.dblLink6CogZ,2)*KUKA_LBR_param_.dblLink6Mass*cos(q3)*sin(q2)*sin(q4) + power(KUKA_LBR_param_.dblLink6CogX,2)*KUKA_LBR_param_.dblLink6Mass*cos(q3)*power(cos(q6),2)*sin(q2)*sin(q4) - power(KUKA_LBR_param_.dblLink6CogY,2)*KUKA_LBR_param_.dblLink6Mass*cos(q3)*power(cos(q6),2)*sin(q2)*sin(q4) + 2*KUKA_LBR_param_.dblLink6InertXZ*sin(q1)*sin(q3)*sin(q4) + 2*cos(q1)*(KUKA_LBR_param_.dblLink6InertXZ*cos(q4)*sin(q2) - KUKA_LBR_param_.dblLink6InertYZ*sin(q3)*sin(q4)) - 2*KUKA_LBR_param_.dblLink23Len*KUKA_LBR_param_.dblLink6CogZ*KUKA_LBR_param_.dblLink6Mass*cos(q3)*sin(q2)*sin(q5) - 2*KUKA_LBR_param_.dblLink45Len*KUKA_LBR_param_.dblLink6CogZ*KUKA_LBR_param_.dblLink6Mass*cos(q3)*cos(q4)*sin(q2)*sin(q5) - 2*KUKA_LBR_param_.dblLink6CogY*KUKA_LBR_param_.dblLink6CogZ*KUKA_LBR_param_.dblLink6Mass*cos(q3)*cos(q4)*cos(q6)*sin(q2)*sin(q5) + 2*KUKA_LBR_param_.dblLink45Len*KUKA_LBR_param_.dblLink6CogX*KUKA_LBR_param_.dblLink6Mass*cos(q6)*sin(q2)*sin(q3)*sin(q5) + 2*KUKA_LBR_param_.dblLink23Len*KUKA_LBR_param_.dblLink6CogX*KUKA_LBR_param_.dblLink6Mass*cos(q4)*cos(q6)*sin(q2)*sin(q3)*sin(q5) + 2*KUKA_LBR_param_.dblLink6CogX*KUKA_LBR_param_.dblLink6CogY*KUKA_LBR_param_.dblLink6Mass*power(cos(q6),2)*sin(q2)*sin(q3)*sin(q5) + 2*KUKA_LBR_param_.dblLink23Len*KUKA_LBR_param_.dblLink6CogY*KUKA_LBR_param_.dblLink6Mass*cos(q3)*cos(q5)*sin(q2)*sin(q6) + 2*KUKA_LBR_param_.dblLink45Len*KUKA_LBR_param_.dblLink6CogY*KUKA_LBR_param_.dblLink6Mass*cos(q3)*cos(q4)*cos(q5)*sin(q2)*sin(q6) - 2*power(KUKA_LBR_param_.dblLink6CogX,2)*KUKA_LBR_param_.dblLink6Mass*cos(q3)*cos(q4)*cos(q5)*cos(q6)*sin(q2)*sin(q6) - 2*KUKA_LBR_param_.dblLink6CogX*KUKA_LBR_param_.dblLink6CogZ*KUKA_LBR_param_.dblLink6Mass*cos(q5)*sin(q2)*sin(q3)*sin(q6) - 4*KUKA_LBR_param_.dblLink6CogX*KUKA_LBR_param_.dblLink6CogY*KUKA_LBR_param_.dblLink6Mass*cos(q3)*cos(q6)*sin(q2)*sin(q4)*sin(q6) - 2*KUKA_LBR_param_.dblLink6CogX*KUKA_LBR_param_.dblLink6CogZ*KUKA_LBR_param_.dblLink6Mass*cos(q3)*cos(q4)*sin(q2)*sin(q5)*sin(q6) - 2*KUKA_LBR_param_.dblLink45Len*KUKA_LBR_param_.dblLink6CogY*KUKA_LBR_param_.dblLink6Mass*sin(q2)*sin(q3)*sin(q5)*sin(q6) - 2*KUKA_LBR_param_.dblLink23Len*KUKA_LBR_param_.dblLink6CogY*KUKA_LBR_param_.dblLink6Mass*cos(q4)*sin(q2)*sin(q3)*sin(q5)*sin(q6) - 2*power(KUKA_LBR_param_.dblLink6CogY,2)*KUKA_LBR_param_.dblLink6Mass*cos(q6)*sin(q2)*sin(q3)*sin(q5)*sin(q6) + 2*KUKA_LBR_param_.dblLink6CogX*KUKA_LBR_param_.dblLink6CogY*KUKA_LBR_param_.dblLink6Mass*cos(q3)*cos(q4)*cos(q5)*sin(q2)*power(sin(q6),2) - power(KUKA_LBR_param_.dblLink6CogX,2)*KUKA_LBR_param_.dblLink6Mass*cos(q3)*sin(q2)*sin(q4)*power(sin(q6),2) + power(KUKA_LBR_param_.dblLink6CogY,2)*KUKA_LBR_param_.dblLink6Mass*cos(q3)*sin(q2)*sin(q4)*power(sin(q6),2) - 2*KUKA_LBR_param_.dblLink6CogX*KUKA_LBR_param_.dblLink6CogY*KUKA_LBR_param_.dblLink6Mass*sin(q2)*sin(q3)*sin(q5)*power(sin(q6),2) + power(KUKA_LBR_param_.dblLink6CogY,2)*KUKA_LBR_param_.dblLink6Mass*cos(q3)*cos(q4)*cos(q5)*sin(q2)*sin(2*q6) + power(KUKA_LBR_param_.dblLink6CogX,2)*KUKA_LBR_param_.dblLink6Mass*sin(q2)*sin(q3)*sin(q5)*sin(2*q6) + cos(q2)*(-2*sin(q4)*(KUKA_LBR_param_.dblLink6InertXZ*cos(q1)*cos(q3) + KUKA_LBR_param_.dblLink6InertYZ*cos(q3)*sin(q1) - KUKA_LBR_param_.dblLink45Len*KUKA_LBR_param_.dblLink6CogZ*KUKA_LBR_param_.dblLink6Mass*sin(q5) - KUKA_LBR_param_.dblLink6CogY*KUKA_LBR_param_.dblLink6CogZ*KUKA_LBR_param_.dblLink6Mass*cos(q6)*sin(q5) - KUKA_LBR_param_.dblLink6CogX*KUKA_LBR_param_.dblLink6CogZ*KUKA_LBR_param_.dblLink6Mass*sin(q5)*sin(q6) + KUKA_LBR_param_.dblLink6Mass*cos(q5)*(KUKA_LBR_param_.dblLink45Len + KUKA_LBR_param_.dblLink6CogY*cos(q6) + KUKA_LBR_param_.dblLink6CogX*sin(q6))*(-(KUKA_LBR_param_.dblLink6CogX*cos(q6)) + KUKA_LBR_param_.dblLink6CogY*sin(q6))) + cos(q4)*(2*KUKA_LBR_param_.dblLink6InertZZ + power(KUKA_LBR_param_.dblLink6CogX,2)*KUKA_LBR_param_.dblLink6Mass + power(KUKA_LBR_param_.dblLink6CogY,2)*KUKA_LBR_param_.dblLink6Mass + 2*power(KUKA_LBR_param_.dblLink6CogZ,2)*KUKA_LBR_param_.dblLink6Mass + (power(KUKA_LBR_param_.dblLink6CogX,2) - power(KUKA_LBR_param_.dblLink6CogY,2))*KUKA_LBR_param_.dblLink6Mass*cos(2*q6) - 2*KUKA_LBR_param_.dblLink6CogX*KUKA_LBR_param_.dblLink6CogY*KUKA_LBR_param_.dblLink6Mass*sin(2*q6))))/2.0 + KUKA_LBR_param_.dblLink7Mass*(sin(q1)*(-(cos(q4)*sin(q3)*(cos(q5)*(KUKA_LBR_param_.dblLink7CogY*cos(q7) + KUKA_LBR_param_.dblLink7CogX*sin(q7)) + sin(q5)*(KUKA_LBR_param_.dblLink7CogX*cos(q6)*cos(q7) - KUKA_LBR_param_.dblLink7CogZ*sin(q6) - KUKA_LBR_param_.dblLink7CogY*cos(q6)*sin(q7)))) - cos(q3)*(sin(q5)*(KUKA_LBR_param_.dblLink7CogY*cos(q7) + KUKA_LBR_param_.dblLink7CogX*sin(q7)) + cos(q5)*(-(KUKA_LBR_param_.dblLink7CogX*cos(q6)*cos(q7)) + KUKA_LBR_param_.dblLink7CogZ*sin(q6) + KUKA_LBR_param_.dblLink7CogY*cos(q6)*sin(q7)))) + cos(q1)*(sin(q2)*sin(q4)*(cos(q5)*(KUKA_LBR_param_.dblLink7CogY*cos(q7) + KUKA_LBR_param_.dblLink7CogX*sin(q7)) + sin(q5)*(KUKA_LBR_param_.dblLink7CogX*cos(q6)*cos(q7) - KUKA_LBR_param_.dblLink7CogZ*sin(q6) - KUKA_LBR_param_.dblLink7CogY*cos(q6)*sin(q7))) + cos(q2)*(cos(q3)*cos(q4)*(cos(q5)*(KUKA_LBR_param_.dblLink7CogY*cos(q7) + KUKA_LBR_param_.dblLink7CogX*sin(q7)) + sin(q5)*(KUKA_LBR_param_.dblLink7CogX*cos(q6)*cos(q7) - KUKA_LBR_param_.dblLink7CogZ*sin(q6) - KUKA_LBR_param_.dblLink7CogY*cos(q6)*sin(q7))) - sin(q3)*(sin(q5)*(KUKA_LBR_param_.dblLink7CogY*cos(q7) + KUKA_LBR_param_.dblLink7CogX*sin(q7)) + cos(q5)*(-(KUKA_LBR_param_.dblLink7CogX*cos(q6)*cos(q7)) + KUKA_LBR_param_.dblLink7CogZ*sin(q6) + KUKA_LBR_param_.dblLink7CogY*cos(q6)*sin(q7))))))*(cos(q1)*(cos(q3)*(cos(q5)*(KUKA_LBR_param_.dblLink7CogY*cos(q7) + KUKA_LBR_param_.dblLink7CogX*sin(q7)) + sin(q5)*(KUKA_LBR_param_.dblLink7CogX*cos(q6)*cos(q7) - KUKA_LBR_param_.dblLink7CogZ*sin(q6) - KUKA_LBR_param_.dblLink7CogY*cos(q6)*sin(q7))) + sin(q3)*(sin(q4)*(KUKA_LBR_param_.dblLink45Len + KUKA_LBR_param_.dblLink7CogZ*cos(q6) + KUKA_LBR_param_.dblLink7CogX*cos(q7)*sin(q6) - KUKA_LBR_param_.dblLink7CogY*sin(q6)*sin(q7)) - cos(q4)*(sin(q5)*(KUKA_LBR_param_.dblLink7CogY*cos(q7) + KUKA_LBR_param_.dblLink7CogX*sin(q7)) + cos(q5)*(-(KUKA_LBR_param_.dblLink7CogX*cos(q6)*cos(q7)) + KUKA_LBR_param_.dblLink7CogZ*sin(q6) + KUKA_LBR_param_.dblLink7CogY*cos(q6)*sin(q7))))) + sin(q1)*(-(sin(q2)*(KUKA_LBR_param_.dblLink23Len + KUKA_LBR_param_.dblLink7CogY*cos(q7)*sin(q4)*sin(q5) + KUKA_LBR_param_.dblLink7CogX*sin(q4)*sin(q5)*sin(q7) + cos(q5)*sin(q4)*(-(KUKA_LBR_param_.dblLink7CogX*cos(q6)*cos(q7)) + KUKA_LBR_param_.dblLink7CogZ*sin(q6) + KUKA_LBR_param_.dblLink7CogY*cos(q6)*sin(q7)) + cos(q4)*(KUKA_LBR_param_.dblLink45Len + KUKA_LBR_param_.dblLink7CogZ*cos(q6) + KUKA_LBR_param_.dblLink7CogX*cos(q7)*sin(q6) - KUKA_LBR_param_.dblLink7CogY*sin(q6)*sin(q7)))) + cos(q2)*(-(sin(q3)*(cos(q5)*(KUKA_LBR_param_.dblLink7CogY*cos(q7) + KUKA_LBR_param_.dblLink7CogX*sin(q7)) + sin(q5)*(KUKA_LBR_param_.dblLink7CogX*cos(q6)*cos(q7) - KUKA_LBR_param_.dblLink7CogZ*sin(q6) - KUKA_LBR_param_.dblLink7CogY*cos(q6)*sin(q7)))) + cos(q3)*(sin(q4)*(KUKA_LBR_param_.dblLink45Len + KUKA_LBR_param_.dblLink7CogZ*cos(q6) + KUKA_LBR_param_.dblLink7CogX*cos(q7)*sin(q6) - KUKA_LBR_param_.dblLink7CogY*sin(q6)*sin(q7)) - cos(q4)*(sin(q5)*(KUKA_LBR_param_.dblLink7CogY*cos(q7) + KUKA_LBR_param_.dblLink7CogX*sin(q7)) + cos(q5)*(-(KUKA_LBR_param_.dblLink7CogX*cos(q6)*cos(q7)) + KUKA_LBR_param_.dblLink7CogZ*sin(q6) + KUKA_LBR_param_.dblLink7CogY*cos(q6)*sin(q7))))))) + KUKA_LBR_param_.dblLink7Mass*(cos(q1)*(cos(q4)*sin(q3)*(cos(q5)*(KUKA_LBR_param_.dblLink7CogY*cos(q7) + KUKA_LBR_param_.dblLink7CogX*sin(q7)) + sin(q5)*(KUKA_LBR_param_.dblLink7CogX*cos(q6)*cos(q7) - KUKA_LBR_param_.dblLink7CogZ*sin(q6) - KUKA_LBR_param_.dblLink7CogY*cos(q6)*sin(q7))) + cos(q3)*(sin(q5)*(KUKA_LBR_param_.dblLink7CogY*cos(q7) + KUKA_LBR_param_.dblLink7CogX*sin(q7)) + cos(q5)*(-(KUKA_LBR_param_.dblLink7CogX*cos(q6)*cos(q7)) + KUKA_LBR_param_.dblLink7CogZ*sin(q6) + KUKA_LBR_param_.dblLink7CogY*cos(q6)*sin(q7)))) + sin(q1)*(sin(q2)*sin(q4)*(cos(q5)*(KUKA_LBR_param_.dblLink7CogY*cos(q7) + KUKA_LBR_param_.dblLink7CogX*sin(q7)) + sin(q5)*(KUKA_LBR_param_.dblLink7CogX*cos(q6)*cos(q7) - KUKA_LBR_param_.dblLink7CogZ*sin(q6) - KUKA_LBR_param_.dblLink7CogY*cos(q6)*sin(q7))) + cos(q2)*(cos(q3)*cos(q4)*(cos(q5)*(KUKA_LBR_param_.dblLink7CogY*cos(q7) + KUKA_LBR_param_.dblLink7CogX*sin(q7)) + sin(q5)*(KUKA_LBR_param_.dblLink7CogX*cos(q6)*cos(q7) - KUKA_LBR_param_.dblLink7CogZ*sin(q6) - KUKA_LBR_param_.dblLink7CogY*cos(q6)*sin(q7))) - sin(q3)*(sin(q5)*(KUKA_LBR_param_.dblLink7CogY*cos(q7) + KUKA_LBR_param_.dblLink7CogX*sin(q7)) + cos(q5)*(-(KUKA_LBR_param_.dblLink7CogX*cos(q6)*cos(q7)) + KUKA_LBR_param_.dblLink7CogZ*sin(q6) + KUKA_LBR_param_.dblLink7CogY*cos(q6)*sin(q7))))))*(sin(q1)*(cos(q3)*(cos(q5)*(KUKA_LBR_param_.dblLink7CogY*cos(q7) + KUKA_LBR_param_.dblLink7CogX*sin(q7)) + sin(q5)*(KUKA_LBR_param_.dblLink7CogX*cos(q6)*cos(q7) - KUKA_LBR_param_.dblLink7CogZ*sin(q6) - KUKA_LBR_param_.dblLink7CogY*cos(q6)*sin(q7))) + sin(q3)*(sin(q4)*(KUKA_LBR_param_.dblLink45Len + KUKA_LBR_param_.dblLink7CogZ*cos(q6) + KUKA_LBR_param_.dblLink7CogX*cos(q7)*sin(q6) - KUKA_LBR_param_.dblLink7CogY*sin(q6)*sin(q7)) - cos(q4)*(sin(q5)*(KUKA_LBR_param_.dblLink7CogY*cos(q7) + KUKA_LBR_param_.dblLink7CogX*sin(q7)) + cos(q5)*(-(KUKA_LBR_param_.dblLink7CogX*cos(q6)*cos(q7)) + KUKA_LBR_param_.dblLink7CogZ*sin(q6) + KUKA_LBR_param_.dblLink7CogY*cos(q6)*sin(q7))))) + cos(q1)*(sin(q2)*(KUKA_LBR_param_.dblLink23Len + KUKA_LBR_param_.dblLink7CogY*cos(q7)*sin(q4)*sin(q5) + KUKA_LBR_param_.dblLink7CogX*sin(q4)*sin(q5)*sin(q7) + cos(q5)*sin(q4)*(-(KUKA_LBR_param_.dblLink7CogX*cos(q6)*cos(q7)) + KUKA_LBR_param_.dblLink7CogZ*sin(q6) + KUKA_LBR_param_.dblLink7CogY*cos(q6)*sin(q7)) + cos(q4)*(KUKA_LBR_param_.dblLink45Len + KUKA_LBR_param_.dblLink7CogZ*cos(q6) + KUKA_LBR_param_.dblLink7CogX*cos(q7)*sin(q6) - KUKA_LBR_param_.dblLink7CogY*sin(q6)*sin(q7))) + cos(q2)*(sin(q3)*(cos(q5)*(KUKA_LBR_param_.dblLink7CogY*cos(q7) + KUKA_LBR_param_.dblLink7CogX*sin(q7)) + sin(q5)*(KUKA_LBR_param_.dblLink7CogX*cos(q6)*cos(q7) - KUKA_LBR_param_.dblLink7CogZ*sin(q6) - KUKA_LBR_param_.dblLink7CogY*cos(q6)*sin(q7))) + cos(q3)*(-(sin(q4)*(KUKA_LBR_param_.dblLink45Len + KUKA_LBR_param_.dblLink7CogZ*cos(q6) + KUKA_LBR_param_.dblLink7CogX*cos(q7)*sin(q6) - KUKA_LBR_param_.dblLink7CogY*sin(q6)*sin(q7))) + cos(q4)*(sin(q5)*(KUKA_LBR_param_.dblLink7CogY*cos(q7) + KUKA_LBR_param_.dblLink7CogX*sin(q7)) + cos(q5)*(-(KUKA_LBR_param_.dblLink7CogX*cos(q6)*cos(q7)) + KUKA_LBR_param_.dblLink7CogZ*sin(q6) + KUKA_LBR_param_.dblLink7CogY*cos(q6)*sin(q7)))))));
dblMassInertFullRow1Col6 = -(KUKA_LBR_param_.dblLink6InertXZ*cos(q3)*cos(q5)*sin(q1)) - KUKA_LBR_param_.dblLink6CogX*KUKA_LBR_param_.dblLink6CogZ*KUKA_LBR_param_.dblLink6Mass*cos(q3)*cos(q4)*cos(q5)*cos(q6)*sin(q2) + KUKA_LBR_param_.dblLink6InertZZ*cos(q5)*sin(q2)*sin(q3) + power(KUKA_LBR_param_.dblLink6CogX,2)*KUKA_LBR_param_.dblLink6Mass*cos(q5)*sin(q2)*sin(q3) + power(KUKA_LBR_param_.dblLink6CogY,2)*KUKA_LBR_param_.dblLink6Mass*cos(q5)*sin(q2)*sin(q3) + KUKA_LBR_param_.dblLink45Len*KUKA_LBR_param_.dblLink6CogY*KUKA_LBR_param_.dblLink6Mass*cos(q5)*cos(q6)*sin(q2)*sin(q3) + KUKA_LBR_param_.dblLink23Len*KUKA_LBR_param_.dblLink6CogY*KUKA_LBR_param_.dblLink6Mass*cos(q4)*cos(q5)*cos(q6)*sin(q2)*sin(q3) - KUKA_LBR_param_.dblLink6CogY*KUKA_LBR_param_.dblLink6CogZ*KUKA_LBR_param_.dblLink6Mass*cos(q3)*cos(q6)*sin(q2)*sin(q4) - KUKA_LBR_param_.dblLink23Len*KUKA_LBR_param_.dblLink6CogX*KUKA_LBR_param_.dblLink6Mass*cos(q6)*sin(q2)*sin(q3)*sin(q4) + KUKA_LBR_param_.dblLink6InertZZ*cos(q3)*cos(q4)*sin(q2)*sin(q5) + power(KUKA_LBR_param_.dblLink6CogX,2)*KUKA_LBR_param_.dblLink6Mass*cos(q3)*cos(q4)*sin(q2)*sin(q5) + power(KUKA_LBR_param_.dblLink6CogY,2)*KUKA_LBR_param_.dblLink6Mass*cos(q3)*cos(q4)*sin(q2)*sin(q5) + KUKA_LBR_param_.dblLink23Len*KUKA_LBR_param_.dblLink6CogY*KUKA_LBR_param_.dblLink6Mass*cos(q3)*cos(q6)*sin(q2)*sin(q5) + KUKA_LBR_param_.dblLink45Len*KUKA_LBR_param_.dblLink6CogY*KUKA_LBR_param_.dblLink6Mass*cos(q3)*cos(q4)*cos(q6)*sin(q2)*sin(q5) + KUKA_LBR_param_.dblLink6InertXZ*cos(q4)*sin(q1)*sin(q3)*sin(q5) + KUKA_LBR_param_.dblLink6CogX*KUKA_LBR_param_.dblLink6CogZ*KUKA_LBR_param_.dblLink6Mass*cos(q6)*sin(q2)*sin(q3)*sin(q5) - KUKA_LBR_param_.dblLink6InertYZ*sin(q1)*sin(q2)*sin(q4)*sin(q5) + KUKA_LBR_param_.dblLink7InertZZ*(cos(q5)*sin(q2)*sin(q3) + (cos(q3)*cos(q4)*sin(q2) - cos(q2)*sin(q4))*sin(q5)) + KUKA_LBR_param_.dblLink7InertXZ*(-(cos(q5)*(cos(q3)*sin(q1) + cos(q1)*cos(q2)*sin(q3))) + (cos(q4)*sin(q1)*sin(q3) - cos(q1)*(cos(q2)*cos(q3)*cos(q4) + sin(q2)*sin(q4)))*sin(q5)) - cos(q1)*(KUKA_LBR_param_.dblLink6InertXZ*cos(q2)*cos(q5)*sin(q3) + (KUKA_LBR_param_.dblLink6InertYZ*cos(q4)*sin(q3) + KUKA_LBR_param_.dblLink6InertXZ*sin(q2)*sin(q4))*sin(q5) + cos(q3)*(-(KUKA_LBR_param_.dblLink6InertYZ*cos(q5)) + KUKA_LBR_param_.dblLink6InertXZ*cos(q2)*cos(q4)*sin(q5))) + KUKA_LBR_param_.dblLink7InertYZ*(cos(q1)*(cos(q3)*cos(q5) - cos(q4)*sin(q3)*sin(q5)) - sin(q1)*(sin(q2)*sin(q4)*sin(q5) + cos(q2)*(cos(q5)*sin(q3) + cos(q3)*cos(q4)*sin(q5)))) + KUKA_LBR_param_.dblLink6CogY*KUKA_LBR_param_.dblLink6CogZ*KUKA_LBR_param_.dblLink6Mass*cos(q3)*cos(q4)*cos(q5)*sin(q2)*sin(q6) + KUKA_LBR_param_.dblLink45Len*KUKA_LBR_param_.dblLink6CogX*KUKA_LBR_param_.dblLink6Mass*cos(q5)*sin(q2)*sin(q3)*sin(q6) + KUKA_LBR_param_.dblLink23Len*KUKA_LBR_param_.dblLink6CogX*KUKA_LBR_param_.dblLink6Mass*cos(q4)*cos(q5)*sin(q2)*sin(q3)*sin(q6) - KUKA_LBR_param_.dblLink6CogX*KUKA_LBR_param_.dblLink6CogZ*KUKA_LBR_param_.dblLink6Mass*cos(q3)*sin(q2)*sin(q4)*sin(q6) + KUKA_LBR_param_.dblLink23Len*KUKA_LBR_param_.dblLink6CogY*KUKA_LBR_param_.dblLink6Mass*sin(q2)*sin(q3)*sin(q4)*sin(q6) + KUKA_LBR_param_.dblLink23Len*KUKA_LBR_param_.dblLink6CogX*KUKA_LBR_param_.dblLink6Mass*cos(q3)*sin(q2)*sin(q5)*sin(q6) + KUKA_LBR_param_.dblLink45Len*KUKA_LBR_param_.dblLink6CogX*KUKA_LBR_param_.dblLink6Mass*cos(q3)*cos(q4)*sin(q2)*sin(q5)*sin(q6) - KUKA_LBR_param_.dblLink6CogY*KUKA_LBR_param_.dblLink6CogZ*KUKA_LBR_param_.dblLink6Mass*sin(q2)*sin(q3)*sin(q5)*sin(q6) - cos(q2)*(sin(q4)*sin(q5)*(KUKA_LBR_param_.dblLink6InertZZ + power(KUKA_LBR_param_.dblLink6CogX,2)*KUKA_LBR_param_.dblLink6Mass + power(KUKA_LBR_param_.dblLink6CogY,2)*KUKA_LBR_param_.dblLink6Mass + KUKA_LBR_param_.dblLink45Len*KUKA_LBR_param_.dblLink6CogY*KUKA_LBR_param_.dblLink6Mass*cos(q6) + KUKA_LBR_param_.dblLink45Len*KUKA_LBR_param_.dblLink6CogX*KUKA_LBR_param_.dblLink6Mass*sin(q6)) + cos(q4)*(KUKA_LBR_param_.dblLink6CogY*KUKA_LBR_param_.dblLink6CogZ*KUKA_LBR_param_.dblLink6Mass*cos(q6) + KUKA_LBR_param_.dblLink6InertYZ*cos(q3)*sin(q1)*sin(q5) + KUKA_LBR_param_.dblLink6CogX*KUKA_LBR_param_.dblLink6CogZ*KUKA_LBR_param_.dblLink6Mass*sin(q6)) + cos(q5)*(KUKA_LBR_param_.dblLink6InertYZ*sin(q1)*sin(q3) + KUKA_LBR_param_.dblLink6CogZ*KUKA_LBR_param_.dblLink6Mass*sin(q4)*(-(KUKA_LBR_param_.dblLink6CogX*cos(q6)) + KUKA_LBR_param_.dblLink6CogY*sin(q6)))) - KUKA_LBR_param_.dblLink7Mass*(sin(q1)*(cos(q6)*(-(KUKA_LBR_param_.dblLink7CogX*cos(q7)*sin(q3)*sin(q4)) + KUKA_LBR_param_.dblLink7CogZ*cos(q3)*sin(q5) + KUKA_LBR_param_.dblLink7CogY*sin(q3)*sin(q4)*sin(q7)) + sin(q6)*(KUKA_LBR_param_.dblLink7CogZ*sin(q3)*sin(q4) + cos(q3)*sin(q5)*(KUKA_LBR_param_.dblLink7CogX*cos(q7) - KUKA_LBR_param_.dblLink7CogY*sin(q7))) + cos(q4)*cos(q5)*sin(q3)*(KUKA_LBR_param_.dblLink7CogZ*cos(q6) + sin(q6)*(KUKA_LBR_param_.dblLink7CogX*cos(q7) - KUKA_LBR_param_.dblLink7CogY*sin(q7)))) - cos(q1)*(sin(q2)*(cos(q4)*(KUKA_LBR_param_.dblLink7CogX*cos(q6)*cos(q7) - KUKA_LBR_param_.dblLink7CogZ*sin(q6) - KUKA_LBR_param_.dblLink7CogY*cos(q6)*sin(q7)) + cos(q5)*sin(q4)*(KUKA_LBR_param_.dblLink7CogZ*cos(q6) + KUKA_LBR_param_.dblLink7CogX*cos(q7)*sin(q6) - KUKA_LBR_param_.dblLink7CogY*sin(q6)*sin(q7))) + cos(q2)*(-(sin(q3)*sin(q5)*(KUKA_LBR_param_.dblLink7CogZ*cos(q6) + sin(q6)*(KUKA_LBR_param_.dblLink7CogX*cos(q7) - KUKA_LBR_param_.dblLink7CogY*sin(q7)))) + cos(q3)*(sin(q4)*(-(KUKA_LBR_param_.dblLink7CogX*cos(q6)*cos(q7)) + KUKA_LBR_param_.dblLink7CogZ*sin(q6) + KUKA_LBR_param_.dblLink7CogY*cos(q6)*sin(q7)) + cos(q4)*cos(q5)*(KUKA_LBR_param_.dblLink7CogZ*cos(q6) + KUKA_LBR_param_.dblLink7CogX*cos(q7)*sin(q6) - KUKA_LBR_param_.dblLink7CogY*sin(q6)*sin(q7))))))*(cos(q1)*(cos(q3)*(cos(q5)*(KUKA_LBR_param_.dblLink7CogY*cos(q7) + KUKA_LBR_param_.dblLink7CogX*sin(q7)) + sin(q5)*(KUKA_LBR_param_.dblLink7CogX*cos(q6)*cos(q7) - KUKA_LBR_param_.dblLink7CogZ*sin(q6) - KUKA_LBR_param_.dblLink7CogY*cos(q6)*sin(q7))) + sin(q3)*(sin(q4)*(KUKA_LBR_param_.dblLink45Len + KUKA_LBR_param_.dblLink7CogZ*cos(q6) + KUKA_LBR_param_.dblLink7CogX*cos(q7)*sin(q6) - KUKA_LBR_param_.dblLink7CogY*sin(q6)*sin(q7)) - cos(q4)*(sin(q5)*(KUKA_LBR_param_.dblLink7CogY*cos(q7) + KUKA_LBR_param_.dblLink7CogX*sin(q7)) + cos(q5)*(-(KUKA_LBR_param_.dblLink7CogX*cos(q6)*cos(q7)) + KUKA_LBR_param_.dblLink7CogZ*sin(q6) + KUKA_LBR_param_.dblLink7CogY*cos(q6)*sin(q7))))) + sin(q1)*(-(sin(q2)*(KUKA_LBR_param_.dblLink23Len + KUKA_LBR_param_.dblLink7CogY*cos(q7)*sin(q4)*sin(q5) + KUKA_LBR_param_.dblLink7CogX*sin(q4)*sin(q5)*sin(q7) + cos(q5)*sin(q4)*(-(KUKA_LBR_param_.dblLink7CogX*cos(q6)*cos(q7)) + KUKA_LBR_param_.dblLink7CogZ*sin(q6) + KUKA_LBR_param_.dblLink7CogY*cos(q6)*sin(q7)) + cos(q4)*(KUKA_LBR_param_.dblLink45Len + KUKA_LBR_param_.dblLink7CogZ*cos(q6) + KUKA_LBR_param_.dblLink7CogX*cos(q7)*sin(q6) - KUKA_LBR_param_.dblLink7CogY*sin(q6)*sin(q7)))) + cos(q2)*(-(sin(q3)*(cos(q5)*(KUKA_LBR_param_.dblLink7CogY*cos(q7) + KUKA_LBR_param_.dblLink7CogX*sin(q7)) + sin(q5)*(KUKA_LBR_param_.dblLink7CogX*cos(q6)*cos(q7) - KUKA_LBR_param_.dblLink7CogZ*sin(q6) - KUKA_LBR_param_.dblLink7CogY*cos(q6)*sin(q7)))) + cos(q3)*(sin(q4)*(KUKA_LBR_param_.dblLink45Len + KUKA_LBR_param_.dblLink7CogZ*cos(q6) + KUKA_LBR_param_.dblLink7CogX*cos(q7)*sin(q6) - KUKA_LBR_param_.dblLink7CogY*sin(q6)*sin(q7)) - cos(q4)*(sin(q5)*(KUKA_LBR_param_.dblLink7CogY*cos(q7) + KUKA_LBR_param_.dblLink7CogX*sin(q7)) + cos(q5)*(-(KUKA_LBR_param_.dblLink7CogX*cos(q6)*cos(q7)) + KUKA_LBR_param_.dblLink7CogZ*sin(q6) + KUKA_LBR_param_.dblLink7CogY*cos(q6)*sin(q7))))))) + KUKA_LBR_param_.dblLink7Mass*(KUKA_LBR_param_.dblLink7CogZ*cos(q5)*cos(q6)*sin(q1)*sin(q2)*sin(q4) - KUKA_LBR_param_.dblLink7CogX*cos(q1)*cos(q6)*cos(q7)*sin(q3)*sin(q4) + KUKA_LBR_param_.dblLink7CogZ*cos(q1)*cos(q3)*cos(q6)*sin(q5) + KUKA_LBR_param_.dblLink7CogX*cos(q5)*cos(q7)*sin(q1)*sin(q2)*sin(q4)*sin(q6) + KUKA_LBR_param_.dblLink7CogZ*cos(q1)*sin(q3)*sin(q4)*sin(q6) + KUKA_LBR_param_.dblLink7CogX*cos(q1)*cos(q3)*cos(q7)*sin(q5)*sin(q6) + KUKA_LBR_param_.dblLink7CogY*cos(q1)*cos(q6)*sin(q3)*sin(q4)*sin(q7) - KUKA_LBR_param_.dblLink7CogY*cos(q5)*sin(q1)*sin(q2)*sin(q4)*sin(q6)*sin(q7) - KUKA_LBR_param_.dblLink7CogY*cos(q1)*cos(q3)*sin(q5)*sin(q6)*sin(q7) + cos(q4)*(cos(q6)*(KUKA_LBR_param_.dblLink7CogX*cos(q7)*sin(q1)*sin(q2) + KUKA_LBR_param_.dblLink7CogZ*cos(q1)*cos(q5)*sin(q3) - KUKA_LBR_param_.dblLink7CogY*sin(q1)*sin(q2)*sin(q7)) - sin(q6)*(KUKA_LBR_param_.dblLink7CogZ*sin(q1)*sin(q2) + cos(q1)*cos(q5)*sin(q3)*(-(KUKA_LBR_param_.dblLink7CogX*cos(q7)) + KUKA_LBR_param_.dblLink7CogY*sin(q7)))) + cos(q2)*sin(q1)*(-(sin(q3)*sin(q5)*(KUKA_LBR_param_.dblLink7CogZ*cos(q6) + sin(q6)*(KUKA_LBR_param_.dblLink7CogX*cos(q7) - KUKA_LBR_param_.dblLink7CogY*sin(q7)))) + cos(q3)*(sin(q4)*(-(KUKA_LBR_param_.dblLink7CogX*cos(q6)*cos(q7)) + KUKA_LBR_param_.dblLink7CogZ*sin(q6) + KUKA_LBR_param_.dblLink7CogY*cos(q6)*sin(q7)) + cos(q4)*cos(q5)*(KUKA_LBR_param_.dblLink7CogZ*cos(q6) + KUKA_LBR_param_.dblLink7CogX*cos(q7)*sin(q6) - KUKA_LBR_param_.dblLink7CogY*sin(q6)*sin(q7)))))*(sin(q1)*(cos(q3)*(cos(q5)*(KUKA_LBR_param_.dblLink7CogY*cos(q7) + KUKA_LBR_param_.dblLink7CogX*sin(q7)) + sin(q5)*(KUKA_LBR_param_.dblLink7CogX*cos(q6)*cos(q7) - KUKA_LBR_param_.dblLink7CogZ*sin(q6) - KUKA_LBR_param_.dblLink7CogY*cos(q6)*sin(q7))) + sin(q3)*(sin(q4)*(KUKA_LBR_param_.dblLink45Len + KUKA_LBR_param_.dblLink7CogZ*cos(q6) + KUKA_LBR_param_.dblLink7CogX*cos(q7)*sin(q6) - KUKA_LBR_param_.dblLink7CogY*sin(q6)*sin(q7)) - cos(q4)*(sin(q5)*(KUKA_LBR_param_.dblLink7CogY*cos(q7) + KUKA_LBR_param_.dblLink7CogX*sin(q7)) + cos(q5)*(-(KUKA_LBR_param_.dblLink7CogX*cos(q6)*cos(q7)) + KUKA_LBR_param_.dblLink7CogZ*sin(q6) + KUKA_LBR_param_.dblLink7CogY*cos(q6)*sin(q7))))) + cos(q1)*(sin(q2)*(KUKA_LBR_param_.dblLink23Len + KUKA_LBR_param_.dblLink7CogY*cos(q7)*sin(q4)*sin(q5) + KUKA_LBR_param_.dblLink7CogX*sin(q4)*sin(q5)*sin(q7) + cos(q5)*sin(q4)*(-(KUKA_LBR_param_.dblLink7CogX*cos(q6)*cos(q7)) + KUKA_LBR_param_.dblLink7CogZ*sin(q6) + KUKA_LBR_param_.dblLink7CogY*cos(q6)*sin(q7)) + cos(q4)*(KUKA_LBR_param_.dblLink45Len + KUKA_LBR_param_.dblLink7CogZ*cos(q6) + KUKA_LBR_param_.dblLink7CogX*cos(q7)*sin(q6) - KUKA_LBR_param_.dblLink7CogY*sin(q6)*sin(q7))) + cos(q2)*(sin(q3)*(cos(q5)*(KUKA_LBR_param_.dblLink7CogY*cos(q7) + KUKA_LBR_param_.dblLink7CogX*sin(q7)) + sin(q5)*(KUKA_LBR_param_.dblLink7CogX*cos(q6)*cos(q7) - KUKA_LBR_param_.dblLink7CogZ*sin(q6) - KUKA_LBR_param_.dblLink7CogY*cos(q6)*sin(q7))) + cos(q3)*(-(sin(q4)*(KUKA_LBR_param_.dblLink45Len + KUKA_LBR_param_.dblLink7CogZ*cos(q6) + KUKA_LBR_param_.dblLink7CogX*cos(q7)*sin(q6) - KUKA_LBR_param_.dblLink7CogY*sin(q6)*sin(q7))) + cos(q4)*(sin(q5)*(KUKA_LBR_param_.dblLink7CogY*cos(q7) + KUKA_LBR_param_.dblLink7CogX*sin(q7)) + cos(q5)*(-(KUKA_LBR_param_.dblLink7CogX*cos(q6)*cos(q7)) + KUKA_LBR_param_.dblLink7CogZ*sin(q6) + KUKA_LBR_param_.dblLink7CogY*cos(q6)*sin(q7)))))));
dblMassInertFullRow1Col7 = KUKA_LBR_param_.dblLink7InertXZ*(cos(q6)*(sin(q1)*sin(q3)*sin(q4) + cos(q1)*(cos(q4)*sin(q2) - cos(q2)*cos(q3)*sin(q4))) - (cos(q5)*(cos(q4)*sin(q1)*sin(q3) - cos(q1)*(cos(q2)*cos(q3)*cos(q4) + sin(q2)*sin(q4))) + (cos(q3)*sin(q1) + cos(q1)*cos(q2)*sin(q3))*sin(q5))*sin(q6)) + KUKA_LBR_param_.dblLink7InertYZ*(cos(q6)*(cos(q4)*sin(q1)*sin(q2) - (cos(q2)*cos(q3)*sin(q1) + cos(q1)*sin(q3))*sin(q4)) + (cos(q5)*sin(q1)*sin(q2)*sin(q4) + cos(q1)*(cos(q4)*cos(q5)*sin(q3) + cos(q3)*sin(q5)) + cos(q2)*sin(q1)*(cos(q3)*cos(q4)*cos(q5) - sin(q3)*sin(q5)))*sin(q6)) + KUKA_LBR_param_.dblLink7InertZZ*(cos(q2)*(cos(q4)*cos(q6) + cos(q5)*sin(q4)*sin(q6)) + sin(q2)*(sin(q3)*sin(q5)*sin(q6) + cos(q3)*(cos(q6)*sin(q4) - cos(q4)*cos(q5)*sin(q6)))) - KUKA_LBR_param_.dblLink7Mass*(sin(q1)*(cos(q3)*(cos(q6)*sin(q5)*(KUKA_LBR_param_.dblLink7CogY*cos(q7) + KUKA_LBR_param_.dblLink7CogX*sin(q7)) + cos(q5)*(-(KUKA_LBR_param_.dblLink7CogX*cos(q7)) + KUKA_LBR_param_.dblLink7CogY*sin(q7))) + sin(q3)*(sin(q4)*sin(q6)*(KUKA_LBR_param_.dblLink7CogY*cos(q7) + KUKA_LBR_param_.dblLink7CogX*sin(q7)) + cos(q4)*(cos(q5)*cos(q6)*(KUKA_LBR_param_.dblLink7CogY*cos(q7) + KUKA_LBR_param_.dblLink7CogX*sin(q7)) + sin(q5)*(KUKA_LBR_param_.dblLink7CogX*cos(q7) - KUKA_LBR_param_.dblLink7CogY*sin(q7))))) - cos(q1)*(sin(q2)*(cos(q7)*(KUKA_LBR_param_.dblLink7CogX*sin(q4)*sin(q5) - KUKA_LBR_param_.dblLink7CogY*cos(q4)*sin(q6)) - (KUKA_LBR_param_.dblLink7CogY*sin(q4)*sin(q5) + KUKA_LBR_param_.dblLink7CogX*cos(q4)*sin(q6))*sin(q7) + cos(q5)*cos(q6)*sin(q4)*(KUKA_LBR_param_.dblLink7CogY*cos(q7) + KUKA_LBR_param_.dblLink7CogX*sin(q7))) + cos(q2)*(sin(q3)*(-(cos(q6)*sin(q5)*(KUKA_LBR_param_.dblLink7CogY*cos(q7) + KUKA_LBR_param_.dblLink7CogX*sin(q7))) + cos(q5)*(KUKA_LBR_param_.dblLink7CogX*cos(q7) - KUKA_LBR_param_.dblLink7CogY*sin(q7))) + cos(q3)*(sin(q4)*sin(q6)*(KUKA_LBR_param_.dblLink7CogY*cos(q7) + KUKA_LBR_param_.dblLink7CogX*sin(q7)) + cos(q4)*(cos(q5)*cos(q6)*(KUKA_LBR_param_.dblLink7CogY*cos(q7) + KUKA_LBR_param_.dblLink7CogX*sin(q7)) + sin(q5)*(KUKA_LBR_param_.dblLink7CogX*cos(q7) - KUKA_LBR_param_.dblLink7CogY*sin(q7)))))))*(cos(q1)*(cos(q3)*(cos(q5)*(KUKA_LBR_param_.dblLink7CogY*cos(q7) + KUKA_LBR_param_.dblLink7CogX*sin(q7)) + sin(q5)*(KUKA_LBR_param_.dblLink7CogX*cos(q6)*cos(q7) - KUKA_LBR_param_.dblLink7CogZ*sin(q6) - KUKA_LBR_param_.dblLink7CogY*cos(q6)*sin(q7))) + sin(q3)*(sin(q4)*(KUKA_LBR_param_.dblLink45Len + KUKA_LBR_param_.dblLink7CogZ*cos(q6) + KUKA_LBR_param_.dblLink7CogX*cos(q7)*sin(q6) - KUKA_LBR_param_.dblLink7CogY*sin(q6)*sin(q7)) - cos(q4)*(sin(q5)*(KUKA_LBR_param_.dblLink7CogY*cos(q7) + KUKA_LBR_param_.dblLink7CogX*sin(q7)) + cos(q5)*(-(KUKA_LBR_param_.dblLink7CogX*cos(q6)*cos(q7)) + KUKA_LBR_param_.dblLink7CogZ*sin(q6) + KUKA_LBR_param_.dblLink7CogY*cos(q6)*sin(q7))))) + sin(q1)*(-(sin(q2)*(KUKA_LBR_param_.dblLink23Len + KUKA_LBR_param_.dblLink7CogY*cos(q7)*sin(q4)*sin(q5) + KUKA_LBR_param_.dblLink7CogX*sin(q4)*sin(q5)*sin(q7) + cos(q5)*sin(q4)*(-(KUKA_LBR_param_.dblLink7CogX*cos(q6)*cos(q7)) + KUKA_LBR_param_.dblLink7CogZ*sin(q6) + KUKA_LBR_param_.dblLink7CogY*cos(q6)*sin(q7)) + cos(q4)*(KUKA_LBR_param_.dblLink45Len + KUKA_LBR_param_.dblLink7CogZ*cos(q6) + KUKA_LBR_param_.dblLink7CogX*cos(q7)*sin(q6) - KUKA_LBR_param_.dblLink7CogY*sin(q6)*sin(q7)))) + cos(q2)*(-(sin(q3)*(cos(q5)*(KUKA_LBR_param_.dblLink7CogY*cos(q7) + KUKA_LBR_param_.dblLink7CogX*sin(q7)) + sin(q5)*(KUKA_LBR_param_.dblLink7CogX*cos(q6)*cos(q7) - KUKA_LBR_param_.dblLink7CogZ*sin(q6) - KUKA_LBR_param_.dblLink7CogY*cos(q6)*sin(q7)))) + cos(q3)*(sin(q4)*(KUKA_LBR_param_.dblLink45Len + KUKA_LBR_param_.dblLink7CogZ*cos(q6) + KUKA_LBR_param_.dblLink7CogX*cos(q7)*sin(q6) - KUKA_LBR_param_.dblLink7CogY*sin(q6)*sin(q7)) - cos(q4)*(sin(q5)*(KUKA_LBR_param_.dblLink7CogY*cos(q7) + KUKA_LBR_param_.dblLink7CogX*sin(q7)) + cos(q5)*(-(KUKA_LBR_param_.dblLink7CogX*cos(q6)*cos(q7)) + KUKA_LBR_param_.dblLink7CogZ*sin(q6) + KUKA_LBR_param_.dblLink7CogY*cos(q6)*sin(q7))))))) + KUKA_LBR_param_.dblLink7Mass*(cos(q1)*(cos(q3)*(cos(q6)*sin(q5)*(KUKA_LBR_param_.dblLink7CogY*cos(q7) + KUKA_LBR_param_.dblLink7CogX*sin(q7)) + cos(q5)*(-(KUKA_LBR_param_.dblLink7CogX*cos(q7)) + KUKA_LBR_param_.dblLink7CogY*sin(q7))) + sin(q3)*(sin(q4)*sin(q6)*(KUKA_LBR_param_.dblLink7CogY*cos(q7) + KUKA_LBR_param_.dblLink7CogX*sin(q7)) + cos(q4)*(cos(q5)*cos(q6)*(KUKA_LBR_param_.dblLink7CogY*cos(q7) + KUKA_LBR_param_.dblLink7CogX*sin(q7)) + sin(q5)*(KUKA_LBR_param_.dblLink7CogX*cos(q7) - KUKA_LBR_param_.dblLink7CogY*sin(q7))))) + sin(q1)*(sin(q2)*(cos(q7)*(KUKA_LBR_param_.dblLink7CogX*sin(q4)*sin(q5) - KUKA_LBR_param_.dblLink7CogY*cos(q4)*sin(q6)) - (KUKA_LBR_param_.dblLink7CogY*sin(q4)*sin(q5) + KUKA_LBR_param_.dblLink7CogX*cos(q4)*sin(q6))*sin(q7) + cos(q5)*cos(q6)*sin(q4)*(KUKA_LBR_param_.dblLink7CogY*cos(q7) + KUKA_LBR_param_.dblLink7CogX*sin(q7))) + cos(q2)*(sin(q3)*(-(cos(q6)*sin(q5)*(KUKA_LBR_param_.dblLink7CogY*cos(q7) + KUKA_LBR_param_.dblLink7CogX*sin(q7))) + cos(q5)*(KUKA_LBR_param_.dblLink7CogX*cos(q7) - KUKA_LBR_param_.dblLink7CogY*sin(q7))) + cos(q3)*(sin(q4)*sin(q6)*(KUKA_LBR_param_.dblLink7CogY*cos(q7) + KUKA_LBR_param_.dblLink7CogX*sin(q7)) + cos(q4)*(cos(q5)*cos(q6)*(KUKA_LBR_param_.dblLink7CogY*cos(q7) + KUKA_LBR_param_.dblLink7CogX*sin(q7)) + sin(q5)*(KUKA_LBR_param_.dblLink7CogX*cos(q7) - KUKA_LBR_param_.dblLink7CogY*sin(q7)))))))*(sin(q1)*(cos(q3)*(cos(q5)*(KUKA_LBR_param_.dblLink7CogY*cos(q7) + KUKA_LBR_param_.dblLink7CogX*sin(q7)) + sin(q5)*(KUKA_LBR_param_.dblLink7CogX*cos(q6)*cos(q7) - KUKA_LBR_param_.dblLink7CogZ*sin(q6) - KUKA_LBR_param_.dblLink7CogY*cos(q6)*sin(q7))) + sin(q3)*(sin(q4)*(KUKA_LBR_param_.dblLink45Len + KUKA_LBR_param_.dblLink7CogZ*cos(q6) + KUKA_LBR_param_.dblLink7CogX*cos(q7)*sin(q6) - KUKA_LBR_param_.dblLink7CogY*sin(q6)*sin(q7)) - cos(q4)*(sin(q5)*(KUKA_LBR_param_.dblLink7CogY*cos(q7) + KUKA_LBR_param_.dblLink7CogX*sin(q7)) + cos(q5)*(-(KUKA_LBR_param_.dblLink7CogX*cos(q6)*cos(q7)) + KUKA_LBR_param_.dblLink7CogZ*sin(q6) + KUKA_LBR_param_.dblLink7CogY*cos(q6)*sin(q7))))) + cos(q1)*(sin(q2)*(KUKA_LBR_param_.dblLink23Len + KUKA_LBR_param_.dblLink7CogY*cos(q7)*sin(q4)*sin(q5) + KUKA_LBR_param_.dblLink7CogX*sin(q4)*sin(q5)*sin(q7) + cos(q5)*sin(q4)*(-(KUKA_LBR_param_.dblLink7CogX*cos(q6)*cos(q7)) + KUKA_LBR_param_.dblLink7CogZ*sin(q6) + KUKA_LBR_param_.dblLink7CogY*cos(q6)*sin(q7)) + cos(q4)*(KUKA_LBR_param_.dblLink45Len + KUKA_LBR_param_.dblLink7CogZ*cos(q6) + KUKA_LBR_param_.dblLink7CogX*cos(q7)*sin(q6) - KUKA_LBR_param_.dblLink7CogY*sin(q6)*sin(q7))) + cos(q2)*(sin(q3)*(cos(q5)*(KUKA_LBR_param_.dblLink7CogY*cos(q7) + KUKA_LBR_param_.dblLink7CogX*sin(q7)) + sin(q5)*(KUKA_LBR_param_.dblLink7CogX*cos(q6)*cos(q7) - KUKA_LBR_param_.dblLink7CogZ*sin(q6) - KUKA_LBR_param_.dblLink7CogY*cos(q6)*sin(q7))) + cos(q3)*(-(sin(q4)*(KUKA_LBR_param_.dblLink45Len + KUKA_LBR_param_.dblLink7CogZ*cos(q6) + KUKA_LBR_param_.dblLink7CogX*cos(q7)*sin(q6) - KUKA_LBR_param_.dblLink7CogY*sin(q6)*sin(q7))) + cos(q4)*(sin(q5)*(KUKA_LBR_param_.dblLink7CogY*cos(q7) + KUKA_LBR_param_.dblLink7CogX*sin(q7)) + cos(q5)*(-(KUKA_LBR_param_.dblLink7CogX*cos(q6)*cos(q7)) + KUKA_LBR_param_.dblLink7CogZ*sin(q6) + KUKA_LBR_param_.dblLink7CogY*cos(q6)*sin(q7)))))));
dblMassInertFullRow2Col1 = KUKA_LBR_param_.dblLink2InertYZ*cos(q1) + KUKA_LBR_param_.dblLink3InertYZ*cos(q1) + KUKA_LBR_param_.dblLink4InertYZ*cos(q1) + KUKA_LBR_param_.dblLink5InertYZ*cos(q1) + KUKA_LBR_param_.dblLink6InertYZ*cos(q1) + KUKA_LBR_param_.dblLink7InertYZ*cos(q1) - KUKA_LBR_param_.dblLink2CogY*KUKA_LBR_param_.dblLink2CogZ*KUKA_LBR_param_.dblLink2Mass*cos(q2) - KUKA_LBR_param_.dblLink2InertXZ*sin(q1) - KUKA_LBR_param_.dblLink3InertXZ*sin(q1) - KUKA_LBR_param_.dblLink4InertXZ*sin(q1) - KUKA_LBR_param_.dblLink5InertXZ*sin(q1) - KUKA_LBR_param_.dblLink6InertXZ*sin(q1) - KUKA_LBR_param_.dblLink7InertXZ*sin(q1) - KUKA_LBR_param_.dblLink2CogX*KUKA_LBR_param_.dblLink2CogZ*KUKA_LBR_param_.dblLink2Mass*sin(q2) + KUKA_LBR_param_.dblLink3CogX*KUKA_LBR_param_.dblLink3CogY*KUKA_LBR_param_.dblLink3Mass*power(cos(q3),2)*sin(q2) + power(KUKA_LBR_param_.dblLink3CogX,2)*KUKA_LBR_param_.dblLink3Mass*cos(q3)*sin(q2)*sin(q3) - power(KUKA_LBR_param_.dblLink3CogY,2)*KUKA_LBR_param_.dblLink3Mass*cos(q3)*sin(q2)*sin(q3) - KUKA_LBR_param_.dblLink3CogX*KUKA_LBR_param_.dblLink3CogY*KUKA_LBR_param_.dblLink3Mass*sin(q2)*power(sin(q3),2) + (KUKA_LBR_param_.dblLink23Len + KUKA_LBR_param_.dblLink3CogZ)*KUKA_LBR_param_.dblLink3Mass*cos(q2)*(KUKA_LBR_param_.dblLink3CogY*cos(q3) + KUKA_LBR_param_.dblLink3CogX*sin(q3)) + KUKA_LBR_param_.dblLink4Mass*cos(q1)*(cos(q2)*(KUKA_LBR_param_.dblLink23Len - KUKA_LBR_param_.dblLink4CogY*cos(q4) - KUKA_LBR_param_.dblLink4CogX*sin(q4)) - sin(q2)*(KUKA_LBR_param_.dblLink4CogZ*sin(q3) + cos(q3)*(-(KUKA_LBR_param_.dblLink4CogX*cos(q4)) + KUKA_LBR_param_.dblLink4CogY*sin(q4))))*(cos(q1)*(KUKA_LBR_param_.dblLink4CogZ*cos(q3) + sin(q3)*(KUKA_LBR_param_.dblLink4CogX*cos(q4) - KUKA_LBR_param_.dblLink4CogY*sin(q4))) + sin(q1)*(sin(q2)*(-KUKA_LBR_param_.dblLink23Len + KUKA_LBR_param_.dblLink4CogY*cos(q4) + KUKA_LBR_param_.dblLink4CogX*sin(q4)) + cos(q2)*(KUKA_LBR_param_.dblLink4CogX*cos(q3)*cos(q4) - KUKA_LBR_param_.dblLink4CogZ*sin(q3) - KUKA_LBR_param_.dblLink4CogY*cos(q3)*sin(q4)))) + KUKA_LBR_param_.dblLink4Mass*sin(q1)*(cos(q2)*(KUKA_LBR_param_.dblLink23Len - KUKA_LBR_param_.dblLink4CogY*cos(q4) - KUKA_LBR_param_.dblLink4CogX*sin(q4)) - sin(q2)*(KUKA_LBR_param_.dblLink4CogZ*sin(q3) + cos(q3)*(-(KUKA_LBR_param_.dblLink4CogX*cos(q4)) + KUKA_LBR_param_.dblLink4CogY*sin(q4))))*(sin(q1)*(KUKA_LBR_param_.dblLink4CogZ*cos(q3) + sin(q3)*(KUKA_LBR_param_.dblLink4CogX*cos(q4) - KUKA_LBR_param_.dblLink4CogY*sin(q4))) + cos(q1)*(sin(q2)*(KUKA_LBR_param_.dblLink23Len - KUKA_LBR_param_.dblLink4CogY*cos(q4) - KUKA_LBR_param_.dblLink4CogX*sin(q4)) + cos(q2)*(-(KUKA_LBR_param_.dblLink4CogX*cos(q3)*cos(q4)) + KUKA_LBR_param_.dblLink4CogZ*sin(q3) + KUKA_LBR_param_.dblLink4CogY*cos(q3)*sin(q4)))) + KUKA_LBR_param_.dblLink5Mass*sin(q1)*(cos(q2)*(KUKA_LBR_param_.dblLink23Len + (KUKA_LBR_param_.dblLink45Len + KUKA_LBR_param_.dblLink5CogZ)*cos(q4) - KUKA_LBR_param_.dblLink5CogX*cos(q5)*sin(q4) + KUKA_LBR_param_.dblLink5CogY*sin(q4)*sin(q5)) + sin(q2)*(-(sin(q3)*(KUKA_LBR_param_.dblLink5CogY*cos(q5) + KUKA_LBR_param_.dblLink5CogX*sin(q5))) + cos(q3)*((KUKA_LBR_param_.dblLink45Len + KUKA_LBR_param_.dblLink5CogZ)*sin(q4) + cos(q4)*(KUKA_LBR_param_.dblLink5CogX*cos(q5) - KUKA_LBR_param_.dblLink5CogY*sin(q5)))))*(sin(q1)*(cos(q3)*(KUKA_LBR_param_.dblLink5CogY*cos(q5) + KUKA_LBR_param_.dblLink5CogX*sin(q5)) + sin(q3)*((KUKA_LBR_param_.dblLink45Len + KUKA_LBR_param_.dblLink5CogZ)*sin(q4) + cos(q4)*(KUKA_LBR_param_.dblLink5CogX*cos(q5) - KUKA_LBR_param_.dblLink5CogY*sin(q5)))) + cos(q1)*(sin(q2)*(KUKA_LBR_param_.dblLink23Len + (KUKA_LBR_param_.dblLink45Len + KUKA_LBR_param_.dblLink5CogZ)*cos(q4) - KUKA_LBR_param_.dblLink5CogX*cos(q5)*sin(q4) + KUKA_LBR_param_.dblLink5CogY*sin(q4)*sin(q5)) + cos(q2)*(sin(q3)*(KUKA_LBR_param_.dblLink5CogY*cos(q5) + KUKA_LBR_param_.dblLink5CogX*sin(q5)) - cos(q3)*((KUKA_LBR_param_.dblLink45Len + KUKA_LBR_param_.dblLink5CogZ)*sin(q4) + cos(q4)*(KUKA_LBR_param_.dblLink5CogX*cos(q5) - KUKA_LBR_param_.dblLink5CogY*sin(q5)))))) + KUKA_LBR_param_.dblLink5Mass*cos(q1)*(cos(q2)*(KUKA_LBR_param_.dblLink23Len + (KUKA_LBR_param_.dblLink45Len + KUKA_LBR_param_.dblLink5CogZ)*cos(q4) - KUKA_LBR_param_.dblLink5CogX*cos(q5)*sin(q4) + KUKA_LBR_param_.dblLink5CogY*sin(q4)*sin(q5)) + sin(q2)*(-(sin(q3)*(KUKA_LBR_param_.dblLink5CogY*cos(q5) + KUKA_LBR_param_.dblLink5CogX*sin(q5))) + cos(q3)*((KUKA_LBR_param_.dblLink45Len + KUKA_LBR_param_.dblLink5CogZ)*sin(q4) + cos(q4)*(KUKA_LBR_param_.dblLink5CogX*cos(q5) - KUKA_LBR_param_.dblLink5CogY*sin(q5)))))*(cos(q1)*(cos(q3)*(KUKA_LBR_param_.dblLink5CogY*cos(q5) + KUKA_LBR_param_.dblLink5CogX*sin(q5)) + sin(q3)*((KUKA_LBR_param_.dblLink45Len + KUKA_LBR_param_.dblLink5CogZ)*sin(q4) + cos(q4)*(KUKA_LBR_param_.dblLink5CogX*cos(q5) - KUKA_LBR_param_.dblLink5CogY*sin(q5)))) + sin(q1)*(-(sin(q2)*(KUKA_LBR_param_.dblLink23Len + (KUKA_LBR_param_.dblLink45Len + KUKA_LBR_param_.dblLink5CogZ)*cos(q4) - KUKA_LBR_param_.dblLink5CogX*cos(q5)*sin(q4) + KUKA_LBR_param_.dblLink5CogY*sin(q4)*sin(q5))) + cos(q2)*(-(sin(q3)*(KUKA_LBR_param_.dblLink5CogY*cos(q5) + KUKA_LBR_param_.dblLink5CogX*sin(q5))) + cos(q3)*((KUKA_LBR_param_.dblLink45Len + KUKA_LBR_param_.dblLink5CogZ)*sin(q4) + cos(q4)*(KUKA_LBR_param_.dblLink5CogX*cos(q5) - KUKA_LBR_param_.dblLink5CogY*sin(q5)))))) + KUKA_LBR_param_.dblLink6Mass*sin(q1)*(cos(q2)*(KUKA_LBR_param_.dblLink23Len - KUKA_LBR_param_.dblLink6CogX*cos(q5)*cos(q6)*sin(q4) - KUKA_LBR_param_.dblLink6CogZ*sin(q4)*sin(q5) + KUKA_LBR_param_.dblLink6CogY*cos(q5)*sin(q4)*sin(q6) + cos(q4)*(KUKA_LBR_param_.dblLink45Len + KUKA_LBR_param_.dblLink6CogY*cos(q6) + KUKA_LBR_param_.dblLink6CogX*sin(q6))) + sin(q2)*(sin(q3)*(KUKA_LBR_param_.dblLink6CogZ*cos(q5) + sin(q5)*(-(KUKA_LBR_param_.dblLink6CogX*cos(q6)) + KUKA_LBR_param_.dblLink6CogY*sin(q6))) + cos(q3)*(sin(q4)*(KUKA_LBR_param_.dblLink45Len + KUKA_LBR_param_.dblLink6CogY*cos(q6) + KUKA_LBR_param_.dblLink6CogX*sin(q6)) + cos(q4)*(KUKA_LBR_param_.dblLink6CogX*cos(q5)*cos(q6) + KUKA_LBR_param_.dblLink6CogZ*sin(q5) - KUKA_LBR_param_.dblLink6CogY*cos(q5)*sin(q6)))))*(sin(q1)*(-(cos(q3)*(KUKA_LBR_param_.dblLink6CogZ*cos(q5) + sin(q5)*(-(KUKA_LBR_param_.dblLink6CogX*cos(q6)) + KUKA_LBR_param_.dblLink6CogY*sin(q6)))) + sin(q3)*(sin(q4)*(KUKA_LBR_param_.dblLink45Len + KUKA_LBR_param_.dblLink6CogY*cos(q6) + KUKA_LBR_param_.dblLink6CogX*sin(q6)) + cos(q4)*(KUKA_LBR_param_.dblLink6CogX*cos(q5)*cos(q6) + KUKA_LBR_param_.dblLink6CogZ*sin(q5) - KUKA_LBR_param_.dblLink6CogY*cos(q5)*sin(q6)))) - cos(q1)*(-(sin(q2)*(KUKA_LBR_param_.dblLink23Len - KUKA_LBR_param_.dblLink6CogX*cos(q5)*cos(q6)*sin(q4) - KUKA_LBR_param_.dblLink6CogZ*sin(q4)*sin(q5) + KUKA_LBR_param_.dblLink6CogY*cos(q5)*sin(q4)*sin(q6) + cos(q4)*(KUKA_LBR_param_.dblLink45Len + KUKA_LBR_param_.dblLink6CogY*cos(q6) + KUKA_LBR_param_.dblLink6CogX*sin(q6)))) + cos(q2)*(sin(q3)*(KUKA_LBR_param_.dblLink6CogZ*cos(q5) + sin(q5)*(-(KUKA_LBR_param_.dblLink6CogX*cos(q6)) + KUKA_LBR_param_.dblLink6CogY*sin(q6))) + cos(q3)*(sin(q4)*(KUKA_LBR_param_.dblLink45Len + KUKA_LBR_param_.dblLink6CogY*cos(q6) + KUKA_LBR_param_.dblLink6CogX*sin(q6)) + cos(q4)*(KUKA_LBR_param_.dblLink6CogX*cos(q5)*cos(q6) + KUKA_LBR_param_.dblLink6CogZ*sin(q5) - KUKA_LBR_param_.dblLink6CogY*cos(q5)*sin(q6)))))) + KUKA_LBR_param_.dblLink6Mass*cos(q1)*(cos(q2)*(KUKA_LBR_param_.dblLink23Len - KUKA_LBR_param_.dblLink6CogX*cos(q5)*cos(q6)*sin(q4) - KUKA_LBR_param_.dblLink6CogZ*sin(q4)*sin(q5) + KUKA_LBR_param_.dblLink6CogY*cos(q5)*sin(q4)*sin(q6) + cos(q4)*(KUKA_LBR_param_.dblLink45Len + KUKA_LBR_param_.dblLink6CogY*cos(q6) + KUKA_LBR_param_.dblLink6CogX*sin(q6))) + sin(q2)*(sin(q3)*(KUKA_LBR_param_.dblLink6CogZ*cos(q5) + sin(q5)*(-(KUKA_LBR_param_.dblLink6CogX*cos(q6)) + KUKA_LBR_param_.dblLink6CogY*sin(q6))) + cos(q3)*(sin(q4)*(KUKA_LBR_param_.dblLink45Len + KUKA_LBR_param_.dblLink6CogY*cos(q6) + KUKA_LBR_param_.dblLink6CogX*sin(q6)) + cos(q4)*(KUKA_LBR_param_.dblLink6CogX*cos(q5)*cos(q6) + KUKA_LBR_param_.dblLink6CogZ*sin(q5) - KUKA_LBR_param_.dblLink6CogY*cos(q5)*sin(q6)))))*(cos(q1)*(-(cos(q3)*(KUKA_LBR_param_.dblLink6CogZ*cos(q5) + sin(q5)*(-(KUKA_LBR_param_.dblLink6CogX*cos(q6)) + KUKA_LBR_param_.dblLink6CogY*sin(q6)))) + sin(q3)*(sin(q4)*(KUKA_LBR_param_.dblLink45Len + KUKA_LBR_param_.dblLink6CogY*cos(q6) + KUKA_LBR_param_.dblLink6CogX*sin(q6)) + cos(q4)*(KUKA_LBR_param_.dblLink6CogX*cos(q5)*cos(q6) + KUKA_LBR_param_.dblLink6CogZ*sin(q5) - KUKA_LBR_param_.dblLink6CogY*cos(q5)*sin(q6)))) + sin(q1)*(-(sin(q2)*(KUKA_LBR_param_.dblLink23Len - KUKA_LBR_param_.dblLink6CogX*cos(q5)*cos(q6)*sin(q4) - KUKA_LBR_param_.dblLink6CogZ*sin(q4)*sin(q5) + KUKA_LBR_param_.dblLink6CogY*cos(q5)*sin(q4)*sin(q6) + cos(q4)*(KUKA_LBR_param_.dblLink45Len + KUKA_LBR_param_.dblLink6CogY*cos(q6) + KUKA_LBR_param_.dblLink6CogX*sin(q6)))) + cos(q2)*(sin(q3)*(KUKA_LBR_param_.dblLink6CogZ*cos(q5) + sin(q5)*(-(KUKA_LBR_param_.dblLink6CogX*cos(q6)) + KUKA_LBR_param_.dblLink6CogY*sin(q6))) + cos(q3)*(sin(q4)*(KUKA_LBR_param_.dblLink45Len + KUKA_LBR_param_.dblLink6CogY*cos(q6) + KUKA_LBR_param_.dblLink6CogX*sin(q6)) + cos(q4)*(KUKA_LBR_param_.dblLink6CogX*cos(q5)*cos(q6) + KUKA_LBR_param_.dblLink6CogZ*sin(q5) - KUKA_LBR_param_.dblLink6CogY*cos(q5)*sin(q6)))))) + KUKA_LBR_param_.dblLink7Mass*sin(q1)*(cos(q2)*(KUKA_LBR_param_.dblLink23Len + KUKA_LBR_param_.dblLink7CogY*cos(q7)*sin(q4)*sin(q5) + KUKA_LBR_param_.dblLink7CogX*sin(q4)*sin(q5)*sin(q7) + cos(q5)*sin(q4)*(-(KUKA_LBR_param_.dblLink7CogX*cos(q6)*cos(q7)) + KUKA_LBR_param_.dblLink7CogZ*sin(q6) + KUKA_LBR_param_.dblLink7CogY*cos(q6)*sin(q7)) + cos(q4)*(KUKA_LBR_param_.dblLink45Len + KUKA_LBR_param_.dblLink7CogZ*cos(q6) + KUKA_LBR_param_.dblLink7CogX*cos(q7)*sin(q6) - KUKA_LBR_param_.dblLink7CogY*sin(q6)*sin(q7))) + sin(q2)*(-(sin(q3)*(cos(q5)*(KUKA_LBR_param_.dblLink7CogY*cos(q7) + KUKA_LBR_param_.dblLink7CogX*sin(q7)) + sin(q5)*(KUKA_LBR_param_.dblLink7CogX*cos(q6)*cos(q7) - KUKA_LBR_param_.dblLink7CogZ*sin(q6) - KUKA_LBR_param_.dblLink7CogY*cos(q6)*sin(q7)))) + cos(q3)*(sin(q4)*(KUKA_LBR_param_.dblLink45Len + KUKA_LBR_param_.dblLink7CogZ*cos(q6) + KUKA_LBR_param_.dblLink7CogX*cos(q7)*sin(q6) - KUKA_LBR_param_.dblLink7CogY*sin(q6)*sin(q7)) - cos(q4)*(sin(q5)*(KUKA_LBR_param_.dblLink7CogY*cos(q7) + KUKA_LBR_param_.dblLink7CogX*sin(q7)) + cos(q5)*(-(KUKA_LBR_param_.dblLink7CogX*cos(q6)*cos(q7)) + KUKA_LBR_param_.dblLink7CogZ*sin(q6) + KUKA_LBR_param_.dblLink7CogY*cos(q6)*sin(q7))))))*(sin(q1)*(cos(q3)*(cos(q5)*(KUKA_LBR_param_.dblLink7CogY*cos(q7) + KUKA_LBR_param_.dblLink7CogX*sin(q7)) + sin(q5)*(KUKA_LBR_param_.dblLink7CogX*cos(q6)*cos(q7) - KUKA_LBR_param_.dblLink7CogZ*sin(q6) - KUKA_LBR_param_.dblLink7CogY*cos(q6)*sin(q7))) + sin(q3)*(sin(q4)*(KUKA_LBR_param_.dblLink45Len + KUKA_LBR_param_.dblLink7CogZ*cos(q6) + KUKA_LBR_param_.dblLink7CogX*cos(q7)*sin(q6) - KUKA_LBR_param_.dblLink7CogY*sin(q6)*sin(q7)) - cos(q4)*(sin(q5)*(KUKA_LBR_param_.dblLink7CogY*cos(q7) + KUKA_LBR_param_.dblLink7CogX*sin(q7)) + cos(q5)*(-(KUKA_LBR_param_.dblLink7CogX*cos(q6)*cos(q7)) + KUKA_LBR_param_.dblLink7CogZ*sin(q6) + KUKA_LBR_param_.dblLink7CogY*cos(q6)*sin(q7))))) + cos(q1)*(sin(q2)*(KUKA_LBR_param_.dblLink23Len + KUKA_LBR_param_.dblLink7CogY*cos(q7)*sin(q4)*sin(q5) + KUKA_LBR_param_.dblLink7CogX*sin(q4)*sin(q5)*sin(q7) + cos(q5)*sin(q4)*(-(KUKA_LBR_param_.dblLink7CogX*cos(q6)*cos(q7)) + KUKA_LBR_param_.dblLink7CogZ*sin(q6) + KUKA_LBR_param_.dblLink7CogY*cos(q6)*sin(q7)) + cos(q4)*(KUKA_LBR_param_.dblLink45Len + KUKA_LBR_param_.dblLink7CogZ*cos(q6) + KUKA_LBR_param_.dblLink7CogX*cos(q7)*sin(q6) - KUKA_LBR_param_.dblLink7CogY*sin(q6)*sin(q7))) + cos(q2)*(sin(q3)*(cos(q5)*(KUKA_LBR_param_.dblLink7CogY*cos(q7) + KUKA_LBR_param_.dblLink7CogX*sin(q7)) + sin(q5)*(KUKA_LBR_param_.dblLink7CogX*cos(q6)*cos(q7) - KUKA_LBR_param_.dblLink7CogZ*sin(q6) - KUKA_LBR_param_.dblLink7CogY*cos(q6)*sin(q7))) + cos(q3)*(-(sin(q4)*(KUKA_LBR_param_.dblLink45Len + KUKA_LBR_param_.dblLink7CogZ*cos(q6) + KUKA_LBR_param_.dblLink7CogX*cos(q7)*sin(q6) - KUKA_LBR_param_.dblLink7CogY*sin(q6)*sin(q7))) + cos(q4)*(sin(q5)*(KUKA_LBR_param_.dblLink7CogY*cos(q7) + KUKA_LBR_param_.dblLink7CogX*sin(q7)) + cos(q5)*(-(KUKA_LBR_param_.dblLink7CogX*cos(q6)*cos(q7)) + KUKA_LBR_param_.dblLink7CogZ*sin(q6) + KUKA_LBR_param_.dblLink7CogY*cos(q6)*sin(q7))))))) - KUKA_LBR_param_.dblLink7Mass*cos(q1)*(cos(q2)*(KUKA_LBR_param_.dblLink23Len + KUKA_LBR_param_.dblLink7CogY*cos(q7)*sin(q4)*sin(q5) + KUKA_LBR_param_.dblLink7CogX*sin(q4)*sin(q5)*sin(q7) + cos(q5)*sin(q4)*(-(KUKA_LBR_param_.dblLink7CogX*cos(q6)*cos(q7)) + KUKA_LBR_param_.dblLink7CogZ*sin(q6) + KUKA_LBR_param_.dblLink7CogY*cos(q6)*sin(q7)) + cos(q4)*(KUKA_LBR_param_.dblLink45Len + KUKA_LBR_param_.dblLink7CogZ*cos(q6) + KUKA_LBR_param_.dblLink7CogX*cos(q7)*sin(q6) - KUKA_LBR_param_.dblLink7CogY*sin(q6)*sin(q7))) + sin(q2)*(-(sin(q3)*(cos(q5)*(KUKA_LBR_param_.dblLink7CogY*cos(q7) + KUKA_LBR_param_.dblLink7CogX*sin(q7)) + sin(q5)*(KUKA_LBR_param_.dblLink7CogX*cos(q6)*cos(q7) - KUKA_LBR_param_.dblLink7CogZ*sin(q6) - KUKA_LBR_param_.dblLink7CogY*cos(q6)*sin(q7)))) + cos(q3)*(sin(q4)*(KUKA_LBR_param_.dblLink45Len + KUKA_LBR_param_.dblLink7CogZ*cos(q6) + KUKA_LBR_param_.dblLink7CogX*cos(q7)*sin(q6) - KUKA_LBR_param_.dblLink7CogY*sin(q6)*sin(q7)) - cos(q4)*(sin(q5)*(KUKA_LBR_param_.dblLink7CogY*cos(q7) + KUKA_LBR_param_.dblLink7CogX*sin(q7)) + cos(q5)*(-(KUKA_LBR_param_.dblLink7CogX*cos(q6)*cos(q7)) + KUKA_LBR_param_.dblLink7CogZ*sin(q6) + KUKA_LBR_param_.dblLink7CogY*cos(q6)*sin(q7))))))*(cos(q1)*(-(cos(q3)*(cos(q5)*(KUKA_LBR_param_.dblLink7CogY*cos(q7) + KUKA_LBR_param_.dblLink7CogX*sin(q7)) + sin(q5)*(KUKA_LBR_param_.dblLink7CogX*cos(q6)*cos(q7) - KUKA_LBR_param_.dblLink7CogZ*sin(q6) - KUKA_LBR_param_.dblLink7CogY*cos(q6)*sin(q7)))) + sin(q3)*(-(sin(q4)*(KUKA_LBR_param_.dblLink45Len + KUKA_LBR_param_.dblLink7CogZ*cos(q6) + KUKA_LBR_param_.dblLink7CogX*cos(q7)*sin(q6) - KUKA_LBR_param_.dblLink7CogY*sin(q6)*sin(q7))) + cos(q4)*(sin(q5)*(KUKA_LBR_param_.dblLink7CogY*cos(q7) + KUKA_LBR_param_.dblLink7CogX*sin(q7)) + cos(q5)*(-(KUKA_LBR_param_.dblLink7CogX*cos(q6)*cos(q7)) + KUKA_LBR_param_.dblLink7CogZ*sin(q6) + KUKA_LBR_param_.dblLink7CogY*cos(q6)*sin(q7))))) + sin(q1)*(sin(q2)*(KUKA_LBR_param_.dblLink23Len + KUKA_LBR_param_.dblLink7CogY*cos(q7)*sin(q4)*sin(q5) + KUKA_LBR_param_.dblLink7CogX*sin(q4)*sin(q5)*sin(q7) + cos(q5)*sin(q4)*(-(KUKA_LBR_param_.dblLink7CogX*cos(q6)*cos(q7)) + KUKA_LBR_param_.dblLink7CogZ*sin(q6) + KUKA_LBR_param_.dblLink7CogY*cos(q6)*sin(q7)) + cos(q4)*(KUKA_LBR_param_.dblLink45Len + KUKA_LBR_param_.dblLink7CogZ*cos(q6) + KUKA_LBR_param_.dblLink7CogX*cos(q7)*sin(q6) - KUKA_LBR_param_.dblLink7CogY*sin(q6)*sin(q7))) + cos(q2)*(sin(q3)*(cos(q5)*(KUKA_LBR_param_.dblLink7CogY*cos(q7) + KUKA_LBR_param_.dblLink7CogX*sin(q7)) + sin(q5)*(KUKA_LBR_param_.dblLink7CogX*cos(q6)*cos(q7) - KUKA_LBR_param_.dblLink7CogZ*sin(q6) - KUKA_LBR_param_.dblLink7CogY*cos(q6)*sin(q7))) + cos(q3)*(-(sin(q4)*(KUKA_LBR_param_.dblLink45Len + KUKA_LBR_param_.dblLink7CogZ*cos(q6) + KUKA_LBR_param_.dblLink7CogX*cos(q7)*sin(q6) - KUKA_LBR_param_.dblLink7CogY*sin(q6)*sin(q7))) + cos(q4)*(sin(q5)*(KUKA_LBR_param_.dblLink7CogY*cos(q7) + KUKA_LBR_param_.dblLink7CogX*sin(q7)) + cos(q5)*(-(KUKA_LBR_param_.dblLink7CogX*cos(q6)*cos(q7)) + KUKA_LBR_param_.dblLink7CogZ*sin(q6) + KUKA_LBR_param_.dblLink7CogY*cos(q6)*sin(q7)))))));
dblMassInertFullRow2Col2 = sin(q1)*(-(KUKA_LBR_param_.dblLink5InertXY*cos(q1)) + KUKA_LBR_param_.dblLink5InertXX*sin(q1)) + cos(q1)*(KUKA_LBR_param_.dblLink5InertYY*cos(q1) - KUKA_LBR_param_.dblLink5InertXY*sin(q1)) + sin(q1)*(-(KUKA_LBR_param_.dblLink6InertXY*cos(q1)) + KUKA_LBR_param_.dblLink6InertXX*sin(q1)) + cos(q1)*(KUKA_LBR_param_.dblLink6InertYY*cos(q1) - KUKA_LBR_param_.dblLink6InertXY*sin(q1)) + sin(q1)*(-(KUKA_LBR_param_.dblLink7InertXY*cos(q1)) + KUKA_LBR_param_.dblLink7InertXX*sin(q1)) + cos(q1)*(KUKA_LBR_param_.dblLink7InertYY*cos(q1) - KUKA_LBR_param_.dblLink7InertXY*sin(q1)) + (KUKA_LBR_param_.dblLink2InertXX + KUKA_LBR_param_.dblLink2InertYY + 2*power(KUKA_LBR_param_.dblLink2CogX,2)*KUKA_LBR_param_.dblLink2Mass + 2*power(KUKA_LBR_param_.dblLink2CogY,2)*KUKA_LBR_param_.dblLink2Mass + (-KUKA_LBR_param_.dblLink2InertXX + KUKA_LBR_param_.dblLink2InertYY)*cos(2*q1) - 2*KUKA_LBR_param_.dblLink2InertXY*sin(2*q1))/2.0 + (KUKA_LBR_param_.dblLink3InertXX + KUKA_LBR_param_.dblLink3InertYY + 2*power(KUKA_LBR_param_.dblLink23Len,2)*KUKA_LBR_param_.dblLink3Mass + power(KUKA_LBR_param_.dblLink3CogX,2)*KUKA_LBR_param_.dblLink3Mass + power(KUKA_LBR_param_.dblLink3CogY,2)*KUKA_LBR_param_.dblLink3Mass + 4*KUKA_LBR_param_.dblLink23Len*KUKA_LBR_param_.dblLink3CogZ*KUKA_LBR_param_.dblLink3Mass + 2*power(KUKA_LBR_param_.dblLink3CogZ,2)*KUKA_LBR_param_.dblLink3Mass + (-KUKA_LBR_param_.dblLink3InertXX + KUKA_LBR_param_.dblLink3InertYY)*cos(2*q1) + (power(KUKA_LBR_param_.dblLink3CogX,2) - power(KUKA_LBR_param_.dblLink3CogY,2))*KUKA_LBR_param_.dblLink3Mass*cos(2*q3) - 2*KUKA_LBR_param_.dblLink3InertXY*sin(2*q1) - 2*KUKA_LBR_param_.dblLink3CogX*KUKA_LBR_param_.dblLink3CogY*KUKA_LBR_param_.dblLink3Mass*sin(2*q3))/2.0 + (4*KUKA_LBR_param_.dblLink4InertXX + 4*KUKA_LBR_param_.dblLink4InertYY + 8*power(KUKA_LBR_param_.dblLink23Len,2)*KUKA_LBR_param_.dblLink4Mass + 6*power(KUKA_LBR_param_.dblLink4CogX,2)*KUKA_LBR_param_.dblLink4Mass + 6*power(KUKA_LBR_param_.dblLink4CogY,2)*KUKA_LBR_param_.dblLink4Mass + 4*power(KUKA_LBR_param_.dblLink4CogZ,2)*KUKA_LBR_param_.dblLink4Mass - 4*(KUKA_LBR_param_.dblLink4InertXX - KUKA_LBR_param_.dblLink4InertYY)*cos(2*q1) + 2*(power(KUKA_LBR_param_.dblLink4CogX,2) + power(KUKA_LBR_param_.dblLink4CogY,2) - 2*power(KUKA_LBR_param_.dblLink4CogZ,2))*KUKA_LBR_param_.dblLink4Mass*cos(2*q3) + power(KUKA_LBR_param_.dblLink4CogX,2)*KUKA_LBR_param_.dblLink4Mass*cos(2*(q3 - q4)) - power(KUKA_LBR_param_.dblLink4CogY,2)*KUKA_LBR_param_.dblLink4Mass*cos(2*(q3 - q4)) + 4*KUKA_LBR_param_.dblLink4CogY*KUKA_LBR_param_.dblLink4CogZ*KUKA_LBR_param_.dblLink4Mass*cos(2*q3 - q4) - 16*KUKA_LBR_param_.dblLink23Len*KUKA_LBR_param_.dblLink4CogY*KUKA_LBR_param_.dblLink4Mass*cos(q4) - 2*power(KUKA_LBR_param_.dblLink4CogX,2)*KUKA_LBR_param_.dblLink4Mass*cos(2*q4) + 2*power(KUKA_LBR_param_.dblLink4CogY,2)*KUKA_LBR_param_.dblLink4Mass*cos(2*q4) + power(KUKA_LBR_param_.dblLink4CogX,2)*KUKA_LBR_param_.dblLink4Mass*cos(2*(q3 + q4)) - power(KUKA_LBR_param_.dblLink4CogY,2)*KUKA_LBR_param_.dblLink4Mass*cos(2*(q3 + q4)) - 4*KUKA_LBR_param_.dblLink4CogY*KUKA_LBR_param_.dblLink4CogZ*KUKA_LBR_param_.dblLink4Mass*cos(2*q3 + q4) - 8*KUKA_LBR_param_.dblLink4InertXY*sin(2*q1) + 2*KUKA_LBR_param_.dblLink4CogX*KUKA_LBR_param_.dblLink4CogY*KUKA_LBR_param_.dblLink4Mass*sin(2*(q3 - q4)) - 4*KUKA_LBR_param_.dblLink4CogX*KUKA_LBR_param_.dblLink4CogZ*KUKA_LBR_param_.dblLink4Mass*sin(2*q3 - q4) - 16*KUKA_LBR_param_.dblLink23Len*KUKA_LBR_param_.dblLink4CogX*KUKA_LBR_param_.dblLink4Mass*sin(q4) + 4*KUKA_LBR_param_.dblLink4CogX*KUKA_LBR_param_.dblLink4CogY*KUKA_LBR_param_.dblLink4Mass*sin(2*q4) - 2*KUKA_LBR_param_.dblLink4CogX*KUKA_LBR_param_.dblLink4CogY*KUKA_LBR_param_.dblLink4Mass*sin(2*(q3 + q4)) - 4*KUKA_LBR_param_.dblLink4CogX*KUKA_LBR_param_.dblLink4CogZ*KUKA_LBR_param_.dblLink4Mass*sin(2*q3 + q4))/8.0 + KUKA_LBR_param_.dblLink5Mass*power(sin(q2)*(KUKA_LBR_param_.dblLink23Len + (KUKA_LBR_param_.dblLink45Len + KUKA_LBR_param_.dblLink5CogZ)*cos(q4) - KUKA_LBR_param_.dblLink5CogX*cos(q5)*sin(q4) + KUKA_LBR_param_.dblLink5CogY*sin(q4)*sin(q5)) + cos(q2)*(sin(q3)*(KUKA_LBR_param_.dblLink5CogY*cos(q5) + KUKA_LBR_param_.dblLink5CogX*sin(q5)) - cos(q3)*((KUKA_LBR_param_.dblLink45Len + KUKA_LBR_param_.dblLink5CogZ)*sin(q4) + cos(q4)*(KUKA_LBR_param_.dblLink5CogX*cos(q5) - KUKA_LBR_param_.dblLink5CogY*sin(q5)))),2) + KUKA_LBR_param_.dblLink5Mass*power(cos(q1),2)*power(cos(q2)*(KUKA_LBR_param_.dblLink23Len + (KUKA_LBR_param_.dblLink45Len + KUKA_LBR_param_.dblLink5CogZ)*cos(q4) - KUKA_LBR_param_.dblLink5CogX*cos(q5)*sin(q4) + KUKA_LBR_param_.dblLink5CogY*sin(q4)*sin(q5)) + sin(q2)*(-(sin(q3)*(KUKA_LBR_param_.dblLink5CogY*cos(q5) + KUKA_LBR_param_.dblLink5CogX*sin(q5))) + cos(q3)*((KUKA_LBR_param_.dblLink45Len + KUKA_LBR_param_.dblLink5CogZ)*sin(q4) + cos(q4)*(KUKA_LBR_param_.dblLink5CogX*cos(q5) - KUKA_LBR_param_.dblLink5CogY*sin(q5)))),2) + KUKA_LBR_param_.dblLink5Mass*power(sin(q1),2)*power(cos(q2)*(KUKA_LBR_param_.dblLink23Len + (KUKA_LBR_param_.dblLink45Len + KUKA_LBR_param_.dblLink5CogZ)*cos(q4) - KUKA_LBR_param_.dblLink5CogX*cos(q5)*sin(q4) + KUKA_LBR_param_.dblLink5CogY*sin(q4)*sin(q5)) + sin(q2)*(-(sin(q3)*(KUKA_LBR_param_.dblLink5CogY*cos(q5) + KUKA_LBR_param_.dblLink5CogX*sin(q5))) + cos(q3)*((KUKA_LBR_param_.dblLink45Len + KUKA_LBR_param_.dblLink5CogZ)*sin(q4) + cos(q4)*(KUKA_LBR_param_.dblLink5CogX*cos(q5) - KUKA_LBR_param_.dblLink5CogY*sin(q5)))),2) + KUKA_LBR_param_.dblLink6Mass*power(sin(q2)*(KUKA_LBR_param_.dblLink23Len - KUKA_LBR_param_.dblLink6CogX*cos(q5)*cos(q6)*sin(q4) - KUKA_LBR_param_.dblLink6CogZ*sin(q4)*sin(q5) + KUKA_LBR_param_.dblLink6CogY*cos(q5)*sin(q4)*sin(q6) + cos(q4)*(KUKA_LBR_param_.dblLink45Len + KUKA_LBR_param_.dblLink6CogY*cos(q6) + KUKA_LBR_param_.dblLink6CogX*sin(q6))) - cos(q2)*(sin(q3)*(KUKA_LBR_param_.dblLink6CogZ*cos(q5) + sin(q5)*(-(KUKA_LBR_param_.dblLink6CogX*cos(q6)) + KUKA_LBR_param_.dblLink6CogY*sin(q6))) + cos(q3)*(sin(q4)*(KUKA_LBR_param_.dblLink45Len + KUKA_LBR_param_.dblLink6CogY*cos(q6) + KUKA_LBR_param_.dblLink6CogX*sin(q6)) + cos(q4)*(KUKA_LBR_param_.dblLink6CogX*cos(q5)*cos(q6) + KUKA_LBR_param_.dblLink6CogZ*sin(q5) - KUKA_LBR_param_.dblLink6CogY*cos(q5)*sin(q6)))),2) + KUKA_LBR_param_.dblLink6Mass*power(cos(q1),2)*power(cos(q2)*(KUKA_LBR_param_.dblLink23Len - KUKA_LBR_param_.dblLink6CogX*cos(q5)*cos(q6)*sin(q4) - KUKA_LBR_param_.dblLink6CogZ*sin(q4)*sin(q5) + KUKA_LBR_param_.dblLink6CogY*cos(q5)*sin(q4)*sin(q6) + cos(q4)*(KUKA_LBR_param_.dblLink45Len + KUKA_LBR_param_.dblLink6CogY*cos(q6) + KUKA_LBR_param_.dblLink6CogX*sin(q6))) + sin(q2)*(sin(q3)*(KUKA_LBR_param_.dblLink6CogZ*cos(q5) + sin(q5)*(-(KUKA_LBR_param_.dblLink6CogX*cos(q6)) + KUKA_LBR_param_.dblLink6CogY*sin(q6))) + cos(q3)*(sin(q4)*(KUKA_LBR_param_.dblLink45Len + KUKA_LBR_param_.dblLink6CogY*cos(q6) + KUKA_LBR_param_.dblLink6CogX*sin(q6)) + cos(q4)*(KUKA_LBR_param_.dblLink6CogX*cos(q5)*cos(q6) + KUKA_LBR_param_.dblLink6CogZ*sin(q5) - KUKA_LBR_param_.dblLink6CogY*cos(q5)*sin(q6)))),2) + KUKA_LBR_param_.dblLink6Mass*power(sin(q1),2)*power(cos(q2)*(KUKA_LBR_param_.dblLink23Len - KUKA_LBR_param_.dblLink6CogX*cos(q5)*cos(q6)*sin(q4) - KUKA_LBR_param_.dblLink6CogZ*sin(q4)*sin(q5) + KUKA_LBR_param_.dblLink6CogY*cos(q5)*sin(q4)*sin(q6) + cos(q4)*(KUKA_LBR_param_.dblLink45Len + KUKA_LBR_param_.dblLink6CogY*cos(q6) + KUKA_LBR_param_.dblLink6CogX*sin(q6))) + sin(q2)*(sin(q3)*(KUKA_LBR_param_.dblLink6CogZ*cos(q5) + sin(q5)*(-(KUKA_LBR_param_.dblLink6CogX*cos(q6)) + KUKA_LBR_param_.dblLink6CogY*sin(q6))) + cos(q3)*(sin(q4)*(KUKA_LBR_param_.dblLink45Len + KUKA_LBR_param_.dblLink6CogY*cos(q6) + KUKA_LBR_param_.dblLink6CogX*sin(q6)) + cos(q4)*(KUKA_LBR_param_.dblLink6CogX*cos(q5)*cos(q6) + KUKA_LBR_param_.dblLink6CogZ*sin(q5) - KUKA_LBR_param_.dblLink6CogY*cos(q5)*sin(q6)))),2) + KUKA_LBR_param_.dblLink7Mass*power(sin(q2)*(KUKA_LBR_param_.dblLink23Len + KUKA_LBR_param_.dblLink7CogY*cos(q7)*sin(q4)*sin(q5) + KUKA_LBR_param_.dblLink7CogX*sin(q4)*sin(q5)*sin(q7) + cos(q5)*sin(q4)*(-(KUKA_LBR_param_.dblLink7CogX*cos(q6)*cos(q7)) + KUKA_LBR_param_.dblLink7CogZ*sin(q6) + KUKA_LBR_param_.dblLink7CogY*cos(q6)*sin(q7)) + cos(q4)*(KUKA_LBR_param_.dblLink45Len + KUKA_LBR_param_.dblLink7CogZ*cos(q6) + KUKA_LBR_param_.dblLink7CogX*cos(q7)*sin(q6) - KUKA_LBR_param_.dblLink7CogY*sin(q6)*sin(q7))) - cos(q2)*(-(sin(q3)*(cos(q5)*(KUKA_LBR_param_.dblLink7CogY*cos(q7) + KUKA_LBR_param_.dblLink7CogX*sin(q7)) + sin(q5)*(KUKA_LBR_param_.dblLink7CogX*cos(q6)*cos(q7) - KUKA_LBR_param_.dblLink7CogZ*sin(q6) - KUKA_LBR_param_.dblLink7CogY*cos(q6)*sin(q7)))) + cos(q3)*(sin(q4)*(KUKA_LBR_param_.dblLink45Len + KUKA_LBR_param_.dblLink7CogZ*cos(q6) + KUKA_LBR_param_.dblLink7CogX*cos(q7)*sin(q6) - KUKA_LBR_param_.dblLink7CogY*sin(q6)*sin(q7)) - cos(q4)*(sin(q5)*(KUKA_LBR_param_.dblLink7CogY*cos(q7) + KUKA_LBR_param_.dblLink7CogX*sin(q7)) + cos(q5)*(-(KUKA_LBR_param_.dblLink7CogX*cos(q6)*cos(q7)) + KUKA_LBR_param_.dblLink7CogZ*sin(q6) + KUKA_LBR_param_.dblLink7CogY*cos(q6)*sin(q7))))),2) + KUKA_LBR_param_.dblLink7Mass*power(cos(q1),2)*power(cos(q2)*(KUKA_LBR_param_.dblLink23Len + KUKA_LBR_param_.dblLink7CogY*cos(q7)*sin(q4)*sin(q5) + KUKA_LBR_param_.dblLink7CogX*sin(q4)*sin(q5)*sin(q7) + cos(q5)*sin(q4)*(-(KUKA_LBR_param_.dblLink7CogX*cos(q6)*cos(q7)) + KUKA_LBR_param_.dblLink7CogZ*sin(q6) + KUKA_LBR_param_.dblLink7CogY*cos(q6)*sin(q7)) + cos(q4)*(KUKA_LBR_param_.dblLink45Len + KUKA_LBR_param_.dblLink7CogZ*cos(q6) + KUKA_LBR_param_.dblLink7CogX*cos(q7)*sin(q6) - KUKA_LBR_param_.dblLink7CogY*sin(q6)*sin(q7))) + sin(q2)*(-(sin(q3)*(cos(q5)*(KUKA_LBR_param_.dblLink7CogY*cos(q7) + KUKA_LBR_param_.dblLink7CogX*sin(q7)) + sin(q5)*(KUKA_LBR_param_.dblLink7CogX*cos(q6)*cos(q7) - KUKA_LBR_param_.dblLink7CogZ*sin(q6) - KUKA_LBR_param_.dblLink7CogY*cos(q6)*sin(q7)))) + cos(q3)*(sin(q4)*(KUKA_LBR_param_.dblLink45Len + KUKA_LBR_param_.dblLink7CogZ*cos(q6) + KUKA_LBR_param_.dblLink7CogX*cos(q7)*sin(q6) - KUKA_LBR_param_.dblLink7CogY*sin(q6)*sin(q7)) - cos(q4)*(sin(q5)*(KUKA_LBR_param_.dblLink7CogY*cos(q7) + KUKA_LBR_param_.dblLink7CogX*sin(q7)) + cos(q5)*(-(KUKA_LBR_param_.dblLink7CogX*cos(q6)*cos(q7)) + KUKA_LBR_param_.dblLink7CogZ*sin(q6) + KUKA_LBR_param_.dblLink7CogY*cos(q6)*sin(q7))))),2) + KUKA_LBR_param_.dblLink7Mass*power(sin(q1),2)*power(cos(q2)*(KUKA_LBR_param_.dblLink23Len + KUKA_LBR_param_.dblLink7CogY*cos(q7)*sin(q4)*sin(q5) + KUKA_LBR_param_.dblLink7CogX*sin(q4)*sin(q5)*sin(q7) + cos(q5)*sin(q4)*(-(KUKA_LBR_param_.dblLink7CogX*cos(q6)*cos(q7)) + KUKA_LBR_param_.dblLink7CogZ*sin(q6) + KUKA_LBR_param_.dblLink7CogY*cos(q6)*sin(q7)) + cos(q4)*(KUKA_LBR_param_.dblLink45Len + KUKA_LBR_param_.dblLink7CogZ*cos(q6) + KUKA_LBR_param_.dblLink7CogX*cos(q7)*sin(q6) - KUKA_LBR_param_.dblLink7CogY*sin(q6)*sin(q7))) + sin(q2)*(-(sin(q3)*(cos(q5)*(KUKA_LBR_param_.dblLink7CogY*cos(q7) + KUKA_LBR_param_.dblLink7CogX*sin(q7)) + sin(q5)*(KUKA_LBR_param_.dblLink7CogX*cos(q6)*cos(q7) - KUKA_LBR_param_.dblLink7CogZ*sin(q6) - KUKA_LBR_param_.dblLink7CogY*cos(q6)*sin(q7)))) + cos(q3)*(sin(q4)*(KUKA_LBR_param_.dblLink45Len + KUKA_LBR_param_.dblLink7CogZ*cos(q6) + KUKA_LBR_param_.dblLink7CogX*cos(q7)*sin(q6) - KUKA_LBR_param_.dblLink7CogY*sin(q6)*sin(q7)) - cos(q4)*(sin(q5)*(KUKA_LBR_param_.dblLink7CogY*cos(q7) + KUKA_LBR_param_.dblLink7CogX*sin(q7)) + cos(q5)*(-(KUKA_LBR_param_.dblLink7CogX*cos(q6)*cos(q7)) + KUKA_LBR_param_.dblLink7CogZ*sin(q6) + KUKA_LBR_param_.dblLink7CogY*cos(q6)*sin(q7))))),2);
dblMassInertFullRow2Col3 = KUKA_LBR_param_.dblLink3CogY*(KUKA_LBR_param_.dblLink23Len + KUKA_LBR_param_.dblLink3CogZ)*KUKA_LBR_param_.dblLink3Mass*cos(q3) - KUKA_LBR_param_.dblLink3InertXZ*cos(q2)*sin(q1) - KUKA_LBR_param_.dblLink4InertXZ*cos(q2)*sin(q1) + cos(q2)*(KUKA_LBR_param_.dblLink7InertYZ*cos(q1) - KUKA_LBR_param_.dblLink7InertXZ*sin(q1)) + KUKA_LBR_param_.dblLink3InertXY*power(cos(q1),2)*sin(q2) + KUKA_LBR_param_.dblLink4InertXY*power(cos(q1),2)*sin(q2) + KUKA_LBR_param_.dblLink5InertXY*power(cos(q1),2)*sin(q2) - KUKA_LBR_param_.dblLink3InertXY*power(sin(q1),2)*sin(q2) - KUKA_LBR_param_.dblLink4InertXY*power(sin(q1),2)*sin(q2) + cos(q1)*(KUKA_LBR_param_.dblLink7InertXY*cos(q1) - KUKA_LBR_param_.dblLink7InertXX*sin(q1))*sin(q2) + sin(q1)*(KUKA_LBR_param_.dblLink7InertYY*cos(q1) - KUKA_LBR_param_.dblLink7InertXY*sin(q1))*sin(q2) + cos(q1)*(KUKA_LBR_param_.dblLink3InertYZ*cos(q2) + (-KUKA_LBR_param_.dblLink3InertXX + KUKA_LBR_param_.dblLink3InertYY)*sin(q1)*sin(q2)) + cos(q1)*(KUKA_LBR_param_.dblLink4InertYZ*cos(q2) + (-KUKA_LBR_param_.dblLink4InertXX + KUKA_LBR_param_.dblLink4InertYY)*sin(q1)*sin(q2)) + cos(q1)*(KUKA_LBR_param_.dblLink5InertYZ*cos(q2) + (-KUKA_LBR_param_.dblLink5InertXX + KUKA_LBR_param_.dblLink5InertYY)*sin(q1)*sin(q2)) + KUKA_LBR_param_.dblLink23Len*KUKA_LBR_param_.dblLink3CogX*KUKA_LBR_param_.dblLink3Mass*sin(q3) + KUKA_LBR_param_.dblLink3CogX*KUKA_LBR_param_.dblLink3CogZ*KUKA_LBR_param_.dblLink3Mass*sin(q3) + KUKA_LBR_param_.dblLink23Len*KUKA_LBR_param_.dblLink4CogX*KUKA_LBR_param_.dblLink4Mass*cos(q4)*sin(q3) - KUKA_LBR_param_.dblLink4CogX*KUKA_LBR_param_.dblLink4CogY*KUKA_LBR_param_.dblLink4Mass*power(cos(q4),2)*sin(q3) - KUKA_LBR_param_.dblLink23Len*KUKA_LBR_param_.dblLink4CogY*KUKA_LBR_param_.dblLink4Mass*sin(q3)*sin(q4) - power(KUKA_LBR_param_.dblLink4CogX,2)*KUKA_LBR_param_.dblLink4Mass*cos(q4)*sin(q3)*sin(q4) + power(KUKA_LBR_param_.dblLink4CogY,2)*KUKA_LBR_param_.dblLink4Mass*cos(q4)*sin(q3)*sin(q4) + KUKA_LBR_param_.dblLink4CogX*KUKA_LBR_param_.dblLink4CogY*KUKA_LBR_param_.dblLink4Mass*sin(q3)*power(sin(q4),2) + KUKA_LBR_param_.dblLink4CogZ*KUKA_LBR_param_.dblLink4Mass*cos(q3)*(KUKA_LBR_param_.dblLink23Len - KUKA_LBR_param_.dblLink4CogY*cos(q4) - KUKA_LBR_param_.dblLink4CogX*sin(q4)) + KUKA_LBR_param_.dblLink5Mass*cos(q3)*(KUKA_LBR_param_.dblLink5CogY*cos(q5) + KUKA_LBR_param_.dblLink5CogX*sin(q5))*(KUKA_LBR_param_.dblLink23Len + (KUKA_LBR_param_.dblLink45Len + KUKA_LBR_param_.dblLink5CogZ)*cos(q4) - KUKA_LBR_param_.dblLink5CogX*cos(q5)*sin(q4) + KUKA_LBR_param_.dblLink5CogY*sin(q4)*sin(q5)) + (-2*KUKA_LBR_param_.dblLink5InertXZ*cos(q2)*sin(q1) - 2*KUKA_LBR_param_.dblLink5InertXY*power(sin(q1),2)*sin(q2) + 2*KUKA_LBR_param_.dblLink5Mass*sin(q3)*(KUKA_LBR_param_.dblLink23Len + (KUKA_LBR_param_.dblLink45Len + KUKA_LBR_param_.dblLink5CogZ)*cos(q4) - KUKA_LBR_param_.dblLink5CogX*cos(q5)*sin(q4) + KUKA_LBR_param_.dblLink5CogY*sin(q4)*sin(q5))*((KUKA_LBR_param_.dblLink45Len + KUKA_LBR_param_.dblLink5CogZ)*sin(q4) + cos(q4)*(KUKA_LBR_param_.dblLink5CogX*cos(q5) - KUKA_LBR_param_.dblLink5CogY*sin(q5))))/2.0 + (-4*KUKA_LBR_param_.dblLink6InertXZ*cos(q2)*sin(q1) + 4*KUKA_LBR_param_.dblLink6InertXY*power(cos(q1),2)*sin(q2) - 4*KUKA_LBR_param_.dblLink6InertXY*power(sin(q1),2)*sin(q2) + 4*cos(q1)*(KUKA_LBR_param_.dblLink6InertYZ*cos(q2) + (-KUKA_LBR_param_.dblLink6InertXX + KUKA_LBR_param_.dblLink6InertYY)*sin(q1)*sin(q2)) + 4*KUKA_LBR_param_.dblLink23Len*KUKA_LBR_param_.dblLink6CogX*KUKA_LBR_param_.dblLink6Mass*cos(q4)*cos(q5)*cos(q6)*sin(q3) + 4*KUKA_LBR_param_.dblLink45Len*KUKA_LBR_param_.dblLink6CogX*KUKA_LBR_param_.dblLink6Mass*power(cos(q4),2)*cos(q5)*cos(q6)*sin(q3) + 4*KUKA_LBR_param_.dblLink6CogX*KUKA_LBR_param_.dblLink6CogY*KUKA_LBR_param_.dblLink6Mass*power(cos(q4),2)*cos(q5)*power(cos(q6),2)*sin(q3) + 4*KUKA_LBR_param_.dblLink23Len*KUKA_LBR_param_.dblLink45Len*KUKA_LBR_param_.dblLink6Mass*sin(q3)*sin(q4) + 4*power(KUKA_LBR_param_.dblLink45Len,2)*KUKA_LBR_param_.dblLink6Mass*cos(q4)*sin(q3)*sin(q4) + power(KUKA_LBR_param_.dblLink6CogX,2)*KUKA_LBR_param_.dblLink6Mass*cos(q4)*sin(q3)*sin(q4) + power(KUKA_LBR_param_.dblLink6CogY,2)*KUKA_LBR_param_.dblLink6Mass*cos(q4)*sin(q3)*sin(q4) - 2*power(KUKA_LBR_param_.dblLink6CogZ,2)*KUKA_LBR_param_.dblLink6Mass*cos(q4)*sin(q3)*sin(q4) - power(KUKA_LBR_param_.dblLink6CogX,2)*KUKA_LBR_param_.dblLink6Mass*cos(q4)*power(cos(q5),2)*sin(q3)*sin(q4) - power(KUKA_LBR_param_.dblLink6CogY,2)*KUKA_LBR_param_.dblLink6Mass*cos(q4)*power(cos(q5),2)*sin(q3)*sin(q4) + 4*KUKA_LBR_param_.dblLink23Len*KUKA_LBR_param_.dblLink6CogY*KUKA_LBR_param_.dblLink6Mass*cos(q6)*sin(q3)*sin(q4) + 8*KUKA_LBR_param_.dblLink45Len*KUKA_LBR_param_.dblLink6CogY*KUKA_LBR_param_.dblLink6Mass*cos(q4)*cos(q6)*sin(q3)*sin(q4) - 3*power(KUKA_LBR_param_.dblLink6CogX,2)*KUKA_LBR_param_.dblLink6Mass*cos(q4)*power(cos(q6),2)*sin(q3)*sin(q4) + 3*power(KUKA_LBR_param_.dblLink6CogY,2)*KUKA_LBR_param_.dblLink6Mass*cos(q4)*power(cos(q6),2)*sin(q3)*sin(q4) - power(KUKA_LBR_param_.dblLink6CogX,2)*KUKA_LBR_param_.dblLink6Mass*cos(q4)*power(cos(q5),2)*power(cos(q6),2)*sin(q3)*sin(q4) + power(KUKA_LBR_param_.dblLink6CogY,2)*KUKA_LBR_param_.dblLink6Mass*cos(q4)*power(cos(q5),2)*power(cos(q6),2)*sin(q3)*sin(q4) - 4*KUKA_LBR_param_.dblLink45Len*KUKA_LBR_param_.dblLink6CogX*KUKA_LBR_param_.dblLink6Mass*cos(q5)*cos(q6)*sin(q3)*power(sin(q4),2) - 4*KUKA_LBR_param_.dblLink6CogX*KUKA_LBR_param_.dblLink6CogY*KUKA_LBR_param_.dblLink6Mass*cos(q5)*power(cos(q6),2)*sin(q3)*power(sin(q4),2) + power(KUKA_LBR_param_.dblLink6CogZ,2)*KUKA_LBR_param_.dblLink6Mass*power(cos(q5),2)*sin(q3)*sin(2*q4) + 4*KUKA_LBR_param_.dblLink23Len*KUKA_LBR_param_.dblLink6CogZ*KUKA_LBR_param_.dblLink6Mass*cos(q4)*sin(q3)*sin(q5) + 4*KUKA_LBR_param_.dblLink45Len*KUKA_LBR_param_.dblLink6CogZ*KUKA_LBR_param_.dblLink6Mass*power(cos(q4),2)*sin(q3)*sin(q5) + 4*KUKA_LBR_param_.dblLink6CogY*KUKA_LBR_param_.dblLink6CogZ*KUKA_LBR_param_.dblLink6Mass*power(cos(q4),2)*cos(q6)*sin(q3)*sin(q5) - 8*KUKA_LBR_param_.dblLink6CogX*KUKA_LBR_param_.dblLink6CogZ*KUKA_LBR_param_.dblLink6Mass*cos(q4)*cos(q5)*cos(q6)*sin(q3)*sin(q4)*sin(q5) - 4*KUKA_LBR_param_.dblLink45Len*KUKA_LBR_param_.dblLink6CogZ*KUKA_LBR_param_.dblLink6Mass*sin(q3)*power(sin(q4),2)*sin(q5) - 4*KUKA_LBR_param_.dblLink6CogY*KUKA_LBR_param_.dblLink6CogZ*KUKA_LBR_param_.dblLink6Mass*cos(q6)*sin(q3)*power(sin(q4),2)*sin(q5) + power(KUKA_LBR_param_.dblLink6CogX,2)*KUKA_LBR_param_.dblLink6Mass*cos(q4)*sin(q3)*sin(q4)*power(sin(q5),2) + power(KUKA_LBR_param_.dblLink6CogY,2)*KUKA_LBR_param_.dblLink6Mass*cos(q4)*sin(q3)*sin(q4)*power(sin(q5),2) - 2*power(KUKA_LBR_param_.dblLink6CogZ,2)*KUKA_LBR_param_.dblLink6Mass*cos(q4)*sin(q3)*sin(q4)*power(sin(q5),2) + power(KUKA_LBR_param_.dblLink6CogX,2)*KUKA_LBR_param_.dblLink6Mass*cos(q4)*power(cos(q6),2)*sin(q3)*sin(q4)*power(sin(q5),2) - power(KUKA_LBR_param_.dblLink6CogY,2)*KUKA_LBR_param_.dblLink6Mass*cos(q4)*power(cos(q6),2)*sin(q3)*sin(q4)*power(sin(q5),2) - 4*KUKA_LBR_param_.dblLink23Len*KUKA_LBR_param_.dblLink6CogY*KUKA_LBR_param_.dblLink6Mass*cos(q4)*cos(q5)*sin(q3)*sin(q6) - 4*KUKA_LBR_param_.dblLink45Len*KUKA_LBR_param_.dblLink6CogY*KUKA_LBR_param_.dblLink6Mass*power(cos(q4),2)*cos(q5)*sin(q3)*sin(q6) + 4*power(KUKA_LBR_param_.dblLink6CogX,2)*KUKA_LBR_param_.dblLink6Mass*power(cos(q4),2)*cos(q5)*cos(q6)*sin(q3)*sin(q6) - 4*power(KUKA_LBR_param_.dblLink6CogY,2)*KUKA_LBR_param_.dblLink6Mass*power(cos(q4),2)*cos(q5)*cos(q6)*sin(q3)*sin(q6) + 4*KUKA_LBR_param_.dblLink23Len*KUKA_LBR_param_.dblLink6CogX*KUKA_LBR_param_.dblLink6Mass*sin(q3)*sin(q4)*sin(q6) + 8*KUKA_LBR_param_.dblLink45Len*KUKA_LBR_param_.dblLink6CogX*KUKA_LBR_param_.dblLink6Mass*cos(q4)*sin(q3)*sin(q4)*sin(q6) + 4*KUKA_LBR_param_.dblLink45Len*KUKA_LBR_param_.dblLink6CogY*KUKA_LBR_param_.dblLink6Mass*cos(q5)*sin(q3)*power(sin(q4),2)*sin(q6) - 4*power(KUKA_LBR_param_.dblLink6CogX,2)*KUKA_LBR_param_.dblLink6Mass*cos(q5)*cos(q6)*sin(q3)*power(sin(q4),2)*sin(q6) + 4*power(KUKA_LBR_param_.dblLink6CogY,2)*KUKA_LBR_param_.dblLink6Mass*cos(q5)*cos(q6)*sin(q3)*power(sin(q4),2)*sin(q6) + 4*KUKA_LBR_param_.dblLink6CogX*KUKA_LBR_param_.dblLink6CogZ*KUKA_LBR_param_.dblLink6Mass*power(cos(q4),2)*sin(q3)*sin(q5)*sin(q6) + 8*KUKA_LBR_param_.dblLink6CogY*KUKA_LBR_param_.dblLink6CogZ*KUKA_LBR_param_.dblLink6Mass*cos(q4)*cos(q5)*sin(q3)*sin(q4)*sin(q5)*sin(q6) - 4*KUKA_LBR_param_.dblLink6CogX*KUKA_LBR_param_.dblLink6CogZ*KUKA_LBR_param_.dblLink6Mass*sin(q3)*power(sin(q4),2)*sin(q5)*sin(q6) - 4*KUKA_LBR_param_.dblLink6CogX*KUKA_LBR_param_.dblLink6CogY*KUKA_LBR_param_.dblLink6Mass*cos(q4)*cos(q6)*sin(q3)*sin(q4)*power(sin(q5),2)*sin(q6) - 4*KUKA_LBR_param_.dblLink6CogX*KUKA_LBR_param_.dblLink6CogY*KUKA_LBR_param_.dblLink6Mass*power(cos(q4),2)*cos(q5)*sin(q3)*power(sin(q6),2) + 3*power(KUKA_LBR_param_.dblLink6CogX,2)*KUKA_LBR_param_.dblLink6Mass*cos(q4)*sin(q3)*sin(q4)*power(sin(q6),2) - 3*power(KUKA_LBR_param_.dblLink6CogY,2)*KUKA_LBR_param_.dblLink6Mass*cos(q4)*sin(q3)*sin(q4)*power(sin(q6),2) + power(KUKA_LBR_param_.dblLink6CogX,2)*KUKA_LBR_param_.dblLink6Mass*cos(q4)*power(cos(q5),2)*sin(q3)*sin(q4)*power(sin(q6),2) - power(KUKA_LBR_param_.dblLink6CogY,2)*KUKA_LBR_param_.dblLink6Mass*cos(q4)*power(cos(q5),2)*sin(q3)*sin(q4)*power(sin(q6),2) + 4*KUKA_LBR_param_.dblLink6CogX*KUKA_LBR_param_.dblLink6CogY*KUKA_LBR_param_.dblLink6Mass*cos(q5)*sin(q3)*power(sin(q4),2)*power(sin(q6),2) - power(KUKA_LBR_param_.dblLink6CogX,2)*KUKA_LBR_param_.dblLink6Mass*cos(q4)*sin(q3)*sin(q4)*power(sin(q5),2)*power(sin(q6),2) + power(KUKA_LBR_param_.dblLink6CogY,2)*KUKA_LBR_param_.dblLink6Mass*cos(q4)*sin(q3)*sin(q4)*power(sin(q5),2)*power(sin(q6),2) - 4*KUKA_LBR_param_.dblLink6Mass*cos(q3)*(KUKA_LBR_param_.dblLink23Len - KUKA_LBR_param_.dblLink6CogX*cos(q5)*cos(q6)*sin(q4) - KUKA_LBR_param_.dblLink6CogZ*sin(q4)*sin(q5) + KUKA_LBR_param_.dblLink6CogY*cos(q5)*sin(q4)*sin(q6) + cos(q4)*(KUKA_LBR_param_.dblLink45Len + KUKA_LBR_param_.dblLink6CogY*cos(q6) + KUKA_LBR_param_.dblLink6CogX*sin(q6)))*(KUKA_LBR_param_.dblLink6CogZ*cos(q5) + sin(q5)*(-(KUKA_LBR_param_.dblLink6CogX*cos(q6)) + KUKA_LBR_param_.dblLink6CogY*sin(q6))) + 3*KUKA_LBR_param_.dblLink6CogX*KUKA_LBR_param_.dblLink6CogY*KUKA_LBR_param_.dblLink6Mass*sin(q3)*sin(2*q4)*sin(2*q6) + KUKA_LBR_param_.dblLink6CogX*KUKA_LBR_param_.dblLink6CogY*KUKA_LBR_param_.dblLink6Mass*power(cos(q5),2)*sin(q3)*sin(2*q4)*sin(2*q6))/4.0 + KUKA_LBR_param_.dblLink7Mass*sin(q2)*(-(cos(q3)*(cos(q5)*(KUKA_LBR_param_.dblLink7CogY*cos(q7) + KUKA_LBR_param_.dblLink7CogX*sin(q7)) + sin(q5)*(KUKA_LBR_param_.dblLink7CogX*cos(q6)*cos(q7) - KUKA_LBR_param_.dblLink7CogZ*sin(q6) - KUKA_LBR_param_.dblLink7CogY*cos(q6)*sin(q7)))) + sin(q3)*(-(sin(q4)*(KUKA_LBR_param_.dblLink45Len + KUKA_LBR_param_.dblLink7CogZ*cos(q6) + KUKA_LBR_param_.dblLink7CogX*cos(q7)*sin(q6) - KUKA_LBR_param_.dblLink7CogY*sin(q6)*sin(q7))) + cos(q4)*(sin(q5)*(KUKA_LBR_param_.dblLink7CogY*cos(q7) + KUKA_LBR_param_.dblLink7CogX*sin(q7)) + cos(q5)*(-(KUKA_LBR_param_.dblLink7CogX*cos(q6)*cos(q7)) + KUKA_LBR_param_.dblLink7CogZ*sin(q6) + KUKA_LBR_param_.dblLink7CogY*cos(q6)*sin(q7)))))*(-(sin(q2)*(KUKA_LBR_param_.dblLink23Len + KUKA_LBR_param_.dblLink7CogY*cos(q7)*sin(q4)*sin(q5) + KUKA_LBR_param_.dblLink7CogX*sin(q4)*sin(q5)*sin(q7) + cos(q5)*sin(q4)*(-(KUKA_LBR_param_.dblLink7CogX*cos(q6)*cos(q7)) + KUKA_LBR_param_.dblLink7CogZ*sin(q6) + KUKA_LBR_param_.dblLink7CogY*cos(q6)*sin(q7)) + cos(q4)*(KUKA_LBR_param_.dblLink45Len + KUKA_LBR_param_.dblLink7CogZ*cos(q6) + KUKA_LBR_param_.dblLink7CogX*cos(q7)*sin(q6) - KUKA_LBR_param_.dblLink7CogY*sin(q6)*sin(q7)))) + cos(q2)*(-(sin(q3)*(cos(q5)*(KUKA_LBR_param_.dblLink7CogY*cos(q7) + KUKA_LBR_param_.dblLink7CogX*sin(q7)) + sin(q5)*(KUKA_LBR_param_.dblLink7CogX*cos(q6)*cos(q7) - KUKA_LBR_param_.dblLink7CogZ*sin(q6) - KUKA_LBR_param_.dblLink7CogY*cos(q6)*sin(q7)))) + cos(q3)*(sin(q4)*(KUKA_LBR_param_.dblLink45Len + KUKA_LBR_param_.dblLink7CogZ*cos(q6) + KUKA_LBR_param_.dblLink7CogX*cos(q7)*sin(q6) - KUKA_LBR_param_.dblLink7CogY*sin(q6)*sin(q7)) - cos(q4)*(sin(q5)*(KUKA_LBR_param_.dblLink7CogY*cos(q7) + KUKA_LBR_param_.dblLink7CogX*sin(q7)) + cos(q5)*(-(KUKA_LBR_param_.dblLink7CogX*cos(q6)*cos(q7)) + KUKA_LBR_param_.dblLink7CogZ*sin(q6) + KUKA_LBR_param_.dblLink7CogY*cos(q6)*sin(q7)))))) + KUKA_LBR_param_.dblLink7Mass*cos(q1)*(cos(q2)*(KUKA_LBR_param_.dblLink23Len + KUKA_LBR_param_.dblLink7CogY*cos(q7)*sin(q4)*sin(q5) + KUKA_LBR_param_.dblLink7CogX*sin(q4)*sin(q5)*sin(q7) + cos(q5)*sin(q4)*(-(KUKA_LBR_param_.dblLink7CogX*cos(q6)*cos(q7)) + KUKA_LBR_param_.dblLink7CogZ*sin(q6) + KUKA_LBR_param_.dblLink7CogY*cos(q6)*sin(q7)) + cos(q4)*(KUKA_LBR_param_.dblLink45Len + KUKA_LBR_param_.dblLink7CogZ*cos(q6) + KUKA_LBR_param_.dblLink7CogX*cos(q7)*sin(q6) - KUKA_LBR_param_.dblLink7CogY*sin(q6)*sin(q7))) + sin(q2)*(-(sin(q3)*(cos(q5)*(KUKA_LBR_param_.dblLink7CogY*cos(q7) + KUKA_LBR_param_.dblLink7CogX*sin(q7)) + sin(q5)*(KUKA_LBR_param_.dblLink7CogX*cos(q6)*cos(q7) - KUKA_LBR_param_.dblLink7CogZ*sin(q6) - KUKA_LBR_param_.dblLink7CogY*cos(q6)*sin(q7)))) + cos(q3)*(sin(q4)*(KUKA_LBR_param_.dblLink45Len + KUKA_LBR_param_.dblLink7CogZ*cos(q6) + KUKA_LBR_param_.dblLink7CogX*cos(q7)*sin(q6) - KUKA_LBR_param_.dblLink7CogY*sin(q6)*sin(q7)) - cos(q4)*(sin(q5)*(KUKA_LBR_param_.dblLink7CogY*cos(q7) + KUKA_LBR_param_.dblLink7CogX*sin(q7)) + cos(q5)*(-(KUKA_LBR_param_.dblLink7CogX*cos(q6)*cos(q7)) + KUKA_LBR_param_.dblLink7CogZ*sin(q6) + KUKA_LBR_param_.dblLink7CogY*cos(q6)*sin(q7))))))*(sin(q1)*(-(sin(q3)*(cos(q5)*(KUKA_LBR_param_.dblLink7CogY*cos(q7) + KUKA_LBR_param_.dblLink7CogX*sin(q7)) + sin(q5)*(KUKA_LBR_param_.dblLink7CogX*cos(q6)*cos(q7) - KUKA_LBR_param_.dblLink7CogZ*sin(q6) - KUKA_LBR_param_.dblLink7CogY*cos(q6)*sin(q7)))) + cos(q3)*(sin(q4)*(KUKA_LBR_param_.dblLink45Len + KUKA_LBR_param_.dblLink7CogZ*cos(q6) + KUKA_LBR_param_.dblLink7CogX*cos(q7)*sin(q6) - KUKA_LBR_param_.dblLink7CogY*sin(q6)*sin(q7)) - cos(q4)*(sin(q5)*(KUKA_LBR_param_.dblLink7CogY*cos(q7) + KUKA_LBR_param_.dblLink7CogX*sin(q7)) + cos(q5)*(-(KUKA_LBR_param_.dblLink7CogX*cos(q6)*cos(q7)) + KUKA_LBR_param_.dblLink7CogZ*sin(q6) + KUKA_LBR_param_.dblLink7CogY*cos(q6)*sin(q7))))) + cos(q1)*cos(q2)*(cos(q3)*(cos(q5)*(KUKA_LBR_param_.dblLink7CogY*cos(q7) + KUKA_LBR_param_.dblLink7CogX*sin(q7)) + sin(q5)*(KUKA_LBR_param_.dblLink7CogX*cos(q6)*cos(q7) - KUKA_LBR_param_.dblLink7CogZ*sin(q6) - KUKA_LBR_param_.dblLink7CogY*cos(q6)*sin(q7))) + sin(q3)*(sin(q4)*(KUKA_LBR_param_.dblLink45Len + KUKA_LBR_param_.dblLink7CogZ*cos(q6) + KUKA_LBR_param_.dblLink7CogX*cos(q7)*sin(q6) - KUKA_LBR_param_.dblLink7CogY*sin(q6)*sin(q7)) - cos(q4)*(sin(q5)*(KUKA_LBR_param_.dblLink7CogY*cos(q7) + KUKA_LBR_param_.dblLink7CogX*sin(q7)) + cos(q5)*(-(KUKA_LBR_param_.dblLink7CogX*cos(q6)*cos(q7)) + KUKA_LBR_param_.dblLink7CogZ*sin(q6) + KUKA_LBR_param_.dblLink7CogY*cos(q6)*sin(q7)))))) + KUKA_LBR_param_.dblLink7Mass*sin(q1)*(cos(q2)*(KUKA_LBR_param_.dblLink23Len + KUKA_LBR_param_.dblLink7CogY*cos(q7)*sin(q4)*sin(q5) + KUKA_LBR_param_.dblLink7CogX*sin(q4)*sin(q5)*sin(q7) + cos(q5)*sin(q4)*(-(KUKA_LBR_param_.dblLink7CogX*cos(q6)*cos(q7)) + KUKA_LBR_param_.dblLink7CogZ*sin(q6) + KUKA_LBR_param_.dblLink7CogY*cos(q6)*sin(q7)) + cos(q4)*(KUKA_LBR_param_.dblLink45Len + KUKA_LBR_param_.dblLink7CogZ*cos(q6) + KUKA_LBR_param_.dblLink7CogX*cos(q7)*sin(q6) - KUKA_LBR_param_.dblLink7CogY*sin(q6)*sin(q7))) + sin(q2)*(-(sin(q3)*(cos(q5)*(KUKA_LBR_param_.dblLink7CogY*cos(q7) + KUKA_LBR_param_.dblLink7CogX*sin(q7)) + sin(q5)*(KUKA_LBR_param_.dblLink7CogX*cos(q6)*cos(q7) - KUKA_LBR_param_.dblLink7CogZ*sin(q6) - KUKA_LBR_param_.dblLink7CogY*cos(q6)*sin(q7)))) + cos(q3)*(sin(q4)*(KUKA_LBR_param_.dblLink45Len + KUKA_LBR_param_.dblLink7CogZ*cos(q6) + KUKA_LBR_param_.dblLink7CogX*cos(q7)*sin(q6) - KUKA_LBR_param_.dblLink7CogY*sin(q6)*sin(q7)) - cos(q4)*(sin(q5)*(KUKA_LBR_param_.dblLink7CogY*cos(q7) + KUKA_LBR_param_.dblLink7CogX*sin(q7)) + cos(q5)*(-(KUKA_LBR_param_.dblLink7CogX*cos(q6)*cos(q7)) + KUKA_LBR_param_.dblLink7CogZ*sin(q6) + KUKA_LBR_param_.dblLink7CogY*cos(q6)*sin(q7))))))*(cos(q2)*sin(q1)*(cos(q3)*(cos(q5)*(KUKA_LBR_param_.dblLink7CogY*cos(q7) + KUKA_LBR_param_.dblLink7CogX*sin(q7)) + sin(q5)*(KUKA_LBR_param_.dblLink7CogX*cos(q6)*cos(q7) - KUKA_LBR_param_.dblLink7CogZ*sin(q6) - KUKA_LBR_param_.dblLink7CogY*cos(q6)*sin(q7))) + sin(q3)*(sin(q4)*(KUKA_LBR_param_.dblLink45Len + KUKA_LBR_param_.dblLink7CogZ*cos(q6) + KUKA_LBR_param_.dblLink7CogX*cos(q7)*sin(q6) - KUKA_LBR_param_.dblLink7CogY*sin(q6)*sin(q7)) - cos(q4)*(sin(q5)*(KUKA_LBR_param_.dblLink7CogY*cos(q7) + KUKA_LBR_param_.dblLink7CogX*sin(q7)) + cos(q5)*(-(KUKA_LBR_param_.dblLink7CogX*cos(q6)*cos(q7)) + KUKA_LBR_param_.dblLink7CogZ*sin(q6) + KUKA_LBR_param_.dblLink7CogY*cos(q6)*sin(q7))))) + cos(q1)*(sin(q3)*(cos(q5)*(KUKA_LBR_param_.dblLink7CogY*cos(q7) + KUKA_LBR_param_.dblLink7CogX*sin(q7)) + sin(q5)*(KUKA_LBR_param_.dblLink7CogX*cos(q6)*cos(q7) - KUKA_LBR_param_.dblLink7CogZ*sin(q6) - KUKA_LBR_param_.dblLink7CogY*cos(q6)*sin(q7))) + cos(q3)*(-(sin(q4)*(KUKA_LBR_param_.dblLink45Len + KUKA_LBR_param_.dblLink7CogZ*cos(q6) + KUKA_LBR_param_.dblLink7CogX*cos(q7)*sin(q6) - KUKA_LBR_param_.dblLink7CogY*sin(q6)*sin(q7))) + cos(q4)*(sin(q5)*(KUKA_LBR_param_.dblLink7CogY*cos(q7) + KUKA_LBR_param_.dblLink7CogX*sin(q7)) + cos(q5)*(-(KUKA_LBR_param_.dblLink7CogX*cos(q6)*cos(q7)) + KUKA_LBR_param_.dblLink7CogZ*sin(q6) + KUKA_LBR_param_.dblLink7CogY*cos(q6)*sin(q7))))));
